simulink model "dynamic_model"  (R2018b)
(part 9 of 13)

t6273 = t692+t693+t702+t738+t1614+t1631+t1648+t1649+t2344+t2421+t2698+t2707+t2717+t2719+t3044+t3253+t3338+t3357+t3581+t3643+t3655+t4114+t4115;
t6274 = (t5413+t4146.*(t1861-t3221)).*(t2694-t2701+t3036-t3043).*(t1513+t1879+t2598+t2820+t2834+t3117+t3118).*(-3.633675e-3);
t6275 = (t5413+t4146.*(t1861-t3221)).*(t2694-t2701+t3036-t3043).*(t1513+t1879+t2598+t2820+t2834+t3117+t3118).*3.633675e-3;
t6281 = -t27.*t2363.*(t3435-t3448+t4615+t4619+t3976.*(t1896-t3239).*5.7e-7+t3980.*(t1896-t3239).*4.0e-8);
t6282 = t27.*t2363.*(t3435-t3448+t4615+t4619+t3976.*(t1896-t3239).*5.7e-7+t3980.*(t1896-t3239).*4.0e-8);
t6291 = t3934.*t5855.*(t1513+t1879+t2598+t2820+t2834+t3117+t3118).*(-3.633675e-3);
t6293 = t3934.*t5855.*(t1513+t1879+t2598+t2820+t2834+t3117+t3118).*3.633675e-3;
t6313 = -t2998.*(t3435-t3448+t4615+t4619+t3976.*(t1896-t3239).*5.7e-7+t3980.*(t1896-t3239).*4.0e-8);
t6314 = t2998.*(t3435-t3448+t4615+t4619+t3976.*(t1896-t3239).*5.7e-7+t3980.*(t1896-t3239).*4.0e-8).*(-1.0./2.0);
t6316 = (t5480.*t5603)./2.0;
t6334 = -t3055.*(t3435-t3448+t4615+t4619+t3976.*(t1896-t3239).*5.7e-7+t3980.*(t1896-t3239).*4.0e-8);
t6336 = (t1477-t2502).*(t3435-t3448+t4615+t4619+t3976.*(t1896-t3239).*5.7e-7+t3980.*(t1896-t3239).*4.0e-8);
t6340 = t3055.*(t3435-t3448+t4615+t4619+t3976.*(t1896-t3239).*5.7e-7+t3980.*(t1896-t3239).*4.0e-8).*(-1.0./2.0);
t6350 = -t2297.*(t642+t643-t667+t674+t1587+t1606+t1608+t1609+t2295+t2671+t2683+t2684-t2695+t3279+t3297-t3303+t3597+t3603+t3609-t3614+t4053+t4054);
t6351 = -t2307.*(t642+t643-t667+t674+t1587+t1606+t1608+t1609+t2295+t2671+t2683+t2684-t2695+t3279+t3297-t3303+t3597+t3603+t3609-t3614+t4053+t4054);
t6352 = -t2338.*(t642+t643-t667+t674+t1587+t1606+t1608+t1609+t2295+t2671+t2683+t2684-t2695+t3279+t3297-t3303+t3597+t3603+t3609-t3614+t4053+t4054);
t6353 = t2338.*(t642+t643-t667+t674+t1587+t1606+t1608+t1609+t2295+t2671+t2683+t2684-t2695+t3279+t3297-t3303+t3597+t3603+t3609-t3614+t4053+t4054);
t6354 = (t5466.*t5645)./2.0;
t6376 = -t3396.*(t4617+t4635-t12.*t2363.*t3047.*1.02e-6-t17.*t2363.*t3047.*9.0e-8+t12.*t3980.*(t1896-t3239).*1.02e-6+t17.*t3980.*(t1896-t3239).*9.0e-8);
t6379 = t3396.*(t4617+t4635-t12.*t2363.*t3047.*1.02e-6-t17.*t2363.*t3047.*9.0e-8+t12.*t3980.*(t1896-t3239).*1.02e-6+t17.*t3980.*(t1896-t3239).*9.0e-8);
t6382 = t2363.*(t684+t685-t710+t724+t1686-t1690+t1700+t1701+t2371+t2698+t2707-t2716+t2719+t3329-t3337-t3351-t3641+t3643+t3655-t3659+t4114+t4115).*(-7.26735e-3);
t6383 = t2388.*(t684+t685-t710+t724+t1686-t1690+t1700+t1701+t2371+t2698+t2707-t2716+t2719+t3329-t3337-t3351-t3641+t3643+t3655-t3659+t4114+t4115).*(-7.26735e-3);
t6386 = t2419.*(t684+t685-t710+t724+t1686-t1690+t1700+t1701+t2371+t2698+t2707-t2716+t2719+t3329-t3337-t3351-t3641+t3643+t3655-t3659+t4114+t4115).*(-7.26735e-3);
t6389 = t4002+t4243+t4332+t4408+t4466+t4647;
t6390 = t4797+t4805+t4815+t4825;
t6402 = t27.*(t1896-t3239).*(t3435-t3448+t4615+t4619+t3976.*(t1896-t3239).*5.7e-7+t3980.*(t1896-t3239).*4.0e-8);
t6403 = -t27.*t3547.*(t3435-t3448+t4615+t4619+t3976.*(t1896-t3239).*5.7e-7+t3980.*(t1896-t3239).*4.0e-8);
t6405 = t27.*t3547.*(t3435-t3448+t4615+t4619+t3976.*(t1896-t3239).*5.7e-7+t3980.*(t1896-t3239).*4.0e-8);
t6407 = t3910.*t5904.*(t1488+t1874+t2519+t2740+t2747+t3096+t3097).*(-1.0./2.0);
t6408 = (t3910.*t5904.*(t1488+t1874+t2519+t2740+t2747+t3096+t3097))./2.0;
t6416 = -t27.*t2363.*(t4795+t4801+t4808+t3976.*(t2694-t2701+t3036-t3043).*5.7e-7);
t6417 = t27.*t2363.*(t4795+t4801+t4808+t3976.*(t2694-t2701+t3036-t3043).*5.7e-7);
t6422 = -t2998.*(t4795+t4801+t4808+t3976.*(t2694-t2701+t3036-t3043).*5.7e-7);
t6423 = t2998.*(t4795+t4801+t4808+t3976.*(t2694-t2701+t3036-t3043).*5.7e-7).*(-1.0./2.0);
t6424 = (t2998.*(t4795+t4801+t4808+t3976.*(t2694-t2701+t3036-t3043).*5.7e-7))./2.0;
t6426 = -t3055.*(t4795+t4801+t4808+t3976.*(t2694-t2701+t3036-t3043).*5.7e-7);
t6428 = (t1477-t2502).*(t4795+t4801+t4808+t3976.*(t2694-t2701+t3036-t3043).*5.7e-7);
t6431 = t3055.*(t4795+t4801+t4808+t3976.*(t2694-t2701+t3036-t3043).*5.7e-7).*(-1.0./2.0);
t6432 = (t3055.*(t4795+t4801+t4808+t3976.*(t2694-t2701+t3036-t3043).*5.7e-7))./2.0;
t6441 = t4577.*t6101;
t6462 = t3395.*t6388;
t6471 = -t4019.*(t3435-t3448+t4615+t4619+t3976.*(t1896-t3239).*5.7e-7+t3980.*(t1896-t3239).*4.0e-8);
t6473 = (t3242-t3554).*(t3435-t3448+t4615+t4619+t3976.*(t1896-t3239).*5.7e-7+t3980.*(t1896-t3239).*4.0e-8);
t6474 = -t4026.*(t3435-t3448+t4615+t4619+t3976.*(t1896-t3239).*5.7e-7+t3980.*(t1896-t3239).*4.0e-8);
t6477 = -t4031.*(t3435-t3448+t4615+t4619+t3976.*(t1896-t3239).*5.7e-7+t3980.*(t1896-t3239).*4.0e-8);
t6485 = t27.*(t1896-t3239).*(t4795+t4801+t4808+t3976.*(t2694-t2701+t3036-t3043).*5.7e-7);
t6486 = -t27.*t3547.*(t4795+t4801+t4808+t3976.*(t2694-t2701+t3036-t3043).*5.7e-7);
t6488 = t27.*t3547.*(t4795+t4801+t4808+t3976.*(t2694-t2701+t3036-t3043).*5.7e-7);
t6512 = (t5645.*t5782)./2.0;
t6513 = (t5646.*t5782)./2.0;
t6530 = -t4019.*(t4795+t4801+t4808+t3976.*(t2694-t2701+t3036-t3043).*5.7e-7);
t6531 = (t3242-t3554).*(t4795+t4801+t4808+t3976.*(t2694-t2701+t3036-t3043).*5.7e-7);
t6533 = -t4026.*(t4795+t4801+t4808+t3976.*(t2694-t2701+t3036-t3043).*5.7e-7);
t6537 = -t4031.*(t4795+t4801+t4808+t3976.*(t2694-t2701+t3036-t3043).*5.7e-7);
t6538 = t4026.*(t4795+t4801+t4808+t3976.*(t2694-t2701+t3036-t3043).*5.7e-7);
t6549 = t3049+t3263+t3273+t4010+t4014+t4426+t4431+t4440+t4447;
t6559 = -t4573.*(t4617+t4635-t12.*t2363.*t3047.*1.02e-6-t17.*t2363.*t3047.*9.0e-8+t12.*t3980.*(t1896-t3239).*1.02e-6+t17.*t3980.*(t1896-t3239).*9.0e-8);
t6562 = (t3563-t4051).*(t4617+t4635-t12.*t2363.*t3047.*1.02e-6-t17.*t2363.*t3047.*9.0e-8+t12.*t3980.*(t1896-t3239).*1.02e-6+t17.*t3980.*(t1896-t3239).*9.0e-8);
t6569 = (t5480.*t5901)./2.0;
t6570 = (t5483.*t5901)./2.0;
t6572 = t5902.*(t410-t5466).*(-1.0./2.0);
t6591 = -t4874.*(t3435-t3448+t4615+t4619+t3976.*(t1896-t3239).*5.7e-7+t3980.*(t1896-t3239).*4.0e-8);
t6592 = -t4880.*(t3435-t3448+t4615+t4619+t3976.*(t1896-t3239).*5.7e-7+t3980.*(t1896-t3239).*4.0e-8);
t6596 = t4577.*t6388;
t6607 = t6606./2.0;
t6615 = t3181+t3198+t4793+t4800+t5066+t5071;
t6624 = -t3055.*(t4876+t4905+t4906+t3055.*(t1456-t2355).*1.02e-6+t3047.*(t1477-t2502).*1.02e-6+t3976.*(t3242-t3554).*1.02e-6);
t6625 = t3055.*(t4876+t4905+t4906+t3055.*(t1456-t2355).*1.02e-6+t3047.*(t1477-t2502).*1.02e-6+t3976.*(t3242-t3554).*1.02e-6).*(-1.0./2.0);
et163 = -t2137+t2777+t2778+t2779-t2787+t4050-t4246+t4248+t21.*(t1959-t3313+t38.*t1022.*(t855-t878).*2.196325630278387e-1).*6.1855407534e-5;
et164 = t27.*(t1959-t3313+t38.*t1022.*(t855-t878).*2.196325630278387e-1).*1.35652563578e-4;
t6653 = t5480.*(et163+et164).*(-1.0./2.0);
et165 = -t2137+t2777+t2778+t2779-t2787+t4050-t4246+t4248+t21.*(t1959-t3313+t38.*t1022.*(t855-t878).*2.196325630278387e-1).*6.1855407534e-5;
et166 = t27.*(t1959-t3313+t38.*t1022.*(t855-t878).*2.196325630278387e-1).*1.35652563578e-4;
t6654 = (t5480.*(et165+et166))./2.0;
et167 = -t2137+t2777+t2778+t2779-t2787+t4050-t4246+t4248+t21.*(t1959-t3313+t38.*t1022.*(t855-t878).*2.196325630278387e-1).*6.1855407534e-5;
et168 = t27.*(t1959-t3313+t38.*t1022.*(t855-t878).*2.196325630278387e-1).*1.35652563578e-4;
t6655 = t5483.*(et167+et168).*(-1.0./2.0);
et169 = -t2137+t2777+t2778+t2779-t2787+t4050-t4246+t4248+t21.*(t1959-t3313+t38.*t1022.*(t855-t878).*2.196325630278387e-1).*6.1855407534e-5;
et170 = t27.*(t1959-t3313+t38.*t1022.*(t855-t878).*2.196325630278387e-1).*1.35652563578e-4;
t6656 = (t5483.*(et169+et170))./2.0;
t6658 = t6048.*(t410-t5466).*(-1.0./2.0);
t6659 = -t4874.*(t4795+t4801+t4808+t3976.*(t2694-t2701+t3036-t3043).*5.7e-7);
t6660 = -t4880.*(t4795+t4801+t4808+t3976.*(t2694-t2701+t3036-t3043).*5.7e-7);
t6672 = (t5603.*t6011)./2.0;
t6673 = (t5645.*t6002)./2.0;
t6678 = (t5646.*t6002)./2.0;
et171 = t707+t708-t721-t722-t749+t762+t768-t777-t792-t793-t801-t802-t808+t813-t819+t821-t1629+t1637-t1640-t1641-t1659-t1661+t1666+t1667+t1683+t1692+t1705-t1712+t1758+t1759+t1775+t1776+t1973+t1993+t1994+t2023+t2053+t2060-t2089-t2090+t2098+t2099-t8.*t9.*t15.*t50.*t189.*3.670836568391568e-22;
et172 = t10.*t13.*t14.*t50.*t189.*(-3.279367663374749e-19)-t8.*t9.*t11.*t15.*t50.*t189.*7.075931802640439e-19;
et173 = t8.*t11.*t14.*t15.*t50.*t189.*(-1.190170786299927e-18)-t9.*t11.*t13.*t15.*t50.*t189.*1.190170786299927e-18;
et174 = t13.*t14.*t15.*t16.*t50.*t189.*(-3.226512155691387e-19);
t6687 = t5645.*(et171+et172+et173+et174).*(-1.0./2.0);
et175 = t707+t708-t721-t722-t749+t762+t768-t777-t792-t793-t801-t802-t808+t813-t819+t821-t1629+t1637-t1640-t1641-t1659-t1661+t1666+t1667+t1683+t1692+t1705-t1712+t1758+t1759+t1775+t1776+t1973+t1993+t1994+t2023+t2053+t2060-t2089-t2090+t2098+t2099-t8.*t9.*t15.*t50.*t189.*3.670836568391568e-22;
et176 = t10.*t13.*t14.*t50.*t189.*(-3.279367663374749e-19)-t8.*t9.*t11.*t15.*t50.*t189.*7.075931802640439e-19;
et177 = t8.*t11.*t14.*t15.*t50.*t189.*(-1.190170786299927e-18)-t9.*t11.*t13.*t15.*t50.*t189.*1.190170786299927e-18;
et178 = t13.*t14.*t15.*t16.*t50.*t189.*(-3.226512155691387e-19);
t6688 = (t5645.*(et175+et176+et177+et178))./2.0;
t6715 = -t6713;
t6747 = (t3242-t3554).*(t4876+t4905+t4906+t3055.*(t1456-t2355).*1.02e-6+t3047.*(t1477-t2502).*1.02e-6+t3976.*(t3242-t3554).*1.02e-6);
t6748 = -t4026.*(t4876+t4905+t4906+t3055.*(t1456-t2355).*1.02e-6+t3047.*(t1477-t2502).*1.02e-6+t3976.*(t3242-t3554).*1.02e-6);
t6750 = t4026.*(t4876+t4905+t4906+t3055.*(t1456-t2355).*1.02e-6+t3047.*(t1477-t2502).*1.02e-6+t3976.*(t3242-t3554).*1.02e-6);
t6804 = t3055.*t6726;
t6809 = t5226+t5227+t5229+t5230;
t6859 = (t5466.*t6255)./2.0;
et179 = t1288+t1289+t1302+t1303-t1319-t1320+t1336-t1348+t1350+t1351-t1360+t1369-t1378+t1396-t1425+t1435-t2174+t2183-t2187+t2193-t2194-t2195+t2199-t2203-t2215+t2219-t2222-t2223+t2239+t2240-t2256-t2257+t2555+t2556+t2572+t2583-t2605-t2606+t2612+t2613-t2618-t2619+t2651+t2652;
et180 = t18.*t19.*t20.*t50.*t202.*(-3.566935413776081e-21);
et181 = t24.*t25.*t26.*t50.*t202.*(-3.992732227073824e-24);
et182 = t18.*t19.*t26.*t27.*t50.*t202.*(-3.509445006623964e-21);
et183 = t21.*t24.*t25.*t26.*t50.*t202.*(-7.696420262413979e-21);
t6868 = t5480.*(et179+et180+et181+et182+et183).*(-1.0./2.0);
t6881 = -t21.*t2363.*(-t4494-t4495+t4799+t4823+t3976.*(t2694-t2701+t3036-t3043).*4.0e-8+t3980.*(t2694-t2701+t3036-t3043).*2.4e-7);
t6882 = t21.*t2363.*(-t4494-t4495+t4799+t4823+t3976.*(t2694-t2701+t3036-t3043).*4.0e-8+t3980.*(t2694-t2701+t3036-t3043).*2.4e-7).*(-1.0./2.0);
t6883 = (t21.*t2363.*(-t4494-t4495+t4799+t4823+t3976.*(t2694-t2701+t3036-t3043).*4.0e-8+t3980.*(t2694-t2701+t3036-t3043).*2.4e-7))./2.0;
t6896 = -t3003.*(-t4494-t4495+t4799+t4823+t3976.*(t2694-t2701+t3036-t3043).*4.0e-8+t3980.*(t2694-t2701+t3036-t3043).*2.4e-7);
t6897 = t3003.*(-t4494-t4495+t4799+t4823+t3976.*(t2694-t2701+t3036-t3043).*4.0e-8+t3980.*(t2694-t2701+t3036-t3043).*2.4e-7).*(-1.0./2.0);
t6898 = (t3003.*(-t4494-t4495+t4799+t4823+t3976.*(t2694-t2701+t3036-t3043).*4.0e-8+t3980.*(t2694-t2701+t3036-t3043).*2.4e-7))./2.0;
t6901 = -t3055.*(-t4494-t4495+t4799+t4823+t3976.*(t2694-t2701+t3036-t3043).*4.0e-8+t3980.*(t2694-t2701+t3036-t3043).*2.4e-7);
t6902 = (t1477-t2502).*(-t4494-t4495+t4799+t4823+t3976.*(t2694-t2701+t3036-t3043).*4.0e-8+t3980.*(t2694-t2701+t3036-t3043).*2.4e-7);
t6905 = -t6726.*(t3242-t3554);
t6906 = t4026.*t6726;
t6913 = t4355+t4362+t4929+t4930+t5029+t5030;
t6914 = t5100+t5736+t5749;
t6916 = t3909+t4319+t5019+t5020+t5054+t5055;
t6921 = t21.*(t1896-t3239).*(-t4494-t4495+t4799+t4823+t3976.*(t2694-t2701+t3036-t3043).*4.0e-8+t3980.*(t2694-t2701+t3036-t3043).*2.4e-7);
t6922 = -t21.*t3547.*(-t4494-t4495+t4799+t4823+t3976.*(t2694-t2701+t3036-t3043).*4.0e-8+t3980.*(t2694-t2701+t3036-t3043).*2.4e-7);
t6943 = t3134+t3161+t3162+t3389+t4279+t4283+t4293+t4294+t4299+t4300+t4562+t4568;
t6978 = -t4019.*(-t4494-t4495+t4799+t4823+t3976.*(t2694-t2701+t3036-t3043).*4.0e-8+t3980.*(t2694-t2701+t3036-t3043).*2.4e-7);
t6979 = (t3242-t3554).*(-t4494-t4495+t4799+t4823+t3976.*(t2694-t2701+t3036-t3043).*4.0e-8+t3980.*(t2694-t2701+t3036-t3043).*2.4e-7);
t6980 = -t4026.*(-t4494-t4495+t4799+t4823+t3976.*(t2694-t2701+t3036-t3043).*4.0e-8+t3980.*(t2694-t2701+t3036-t3043).*2.4e-7);
t6984 = -t4031.*(-t4494-t4495+t4799+t4823+t3976.*(t2694-t2701+t3036-t3043).*4.0e-8+t3980.*(t2694-t2701+t3036-t3043).*2.4e-7);
t7002 = t5285+t5293+t5329+t5334;
t7010 = t4018.*(t4814.*(t1861-t3221)+t2297.*(t642+t643-t667+t674+t1587+t1606+t1608+t1609+t2295+t2671+t2683+t2684-t2695+t3279+t3297-t3303+t3597+t3603+t3609-t3614+t4053+t4054)).*(t2694-t2701+t3036-t3043).*3.633675e-3;
t7016 = t3910.*t6652.*(t1488+t1874+t2519+t2740+t2747+t3096+t3097).*(-1.0./2.0);
t7017 = (t3910.*t6652.*(t1488+t1874+t2519+t2740+t2747+t3096+t3097))./2.0;
t7018 = t4187.*(t4814.*(t1861-t3221)+t2297.*(t642+t643-t667+t674+t1587+t1606+t1608+t1609+t2295+t2671+t2683+t2684-t2695+t3279+t3297-t3303+t3597+t3603+t3609-t3614+t4053+t4054)).*(t2694-t2701+t3036-t3043).*3.633675e-3;
t7055 = t7054.*(-1.0./2.0);
t7056 = t7054./2.0;
t7059 = (t3975.*(t4853.*(t1896-t3239).*7.26735e-3+t2363.*(t684+t685-t710+t724+t1686-t1690+t1700+t1701+t2371+t2698+t2707-t2716+t2719+t3329-t3337-t3351-t3641+t3643+t3655-t3659+t4114+t4115).*7.26735e-3).*(t2674-t2676+t3022-t3027))./2.0;
t7080 = (t4146.*(t4853.*(t1896-t3239).*7.26735e-3+t2363.*(t684+t685-t710+t724+t1686-t1690+t1700+t1701+t2371+t2698+t2707-t2716+t2719+t3329-t3337-t3351-t3641+t3643+t3655-t3659+t4114+t4115).*7.26735e-3).*(t2674-t2676+t3022-t3027))./2.0;
t7082 = t5264+t5806+t5822;
t7092 = t3159+t3172+t3449+t3453+t4297+t4304+t4306+t4311+t4579+t4600+t4625+t4629;
t7100 = -t4872.*(-t4494-t4495+t4799+t4823+t3976.*(t2694-t2701+t3036-t3043).*4.0e-8+t3980.*(t2694-t2701+t3036-t3043).*2.4e-7);
et184 = t4165+t27.*(t1959-t3313+t38.*t1022.*(t855-t878).*2.196325630278387e-1);
et185 = -t4494-t4495+t4799+t4823+t3976.*(t2694-t2701+t3036-t3043).*4.0e-8+t3980.*(t2694-t2701+t3036-t3043).*2.4e-7;
t7101 = et184.*et185;
t7155 = t3577+t3578+t5315+t5316+t5323+t5324;
et186 = t3582.*1.33637554986e-4+t3716-t3717+t27.*(t1896-t3239).*4.36041e-5;
et187 = t27.*t28.*(t1896-t3239).*7.26350557185e-5;
t7159 = ((et186+et187).*(t4814.*(t1861-t3221)+t2297.*(t642+t643-t667+t674+t1587+t1606+t1608+t1609+t2295+t2671+t2683+t2684-t2695+t3279+t3297-t3303+t3597+t3603+t3609-t3614+t4053+t4054)))./2.0;
et188 = t4814.*(t1861-t3221)+t2297.*(t642+t643-t667+t674+t1587+t1606+t1608+t1609+t2295+t2671+t2683+t2684-t2695+t3279+t3297-t3303+t3597+t3603+t3609-t3614+t4053+t4054);
et189 = (t3359-t3670+t22.*(t3242-t3554).*1.33637554986e-4+t28.*(t3242-t3554).*7.26350557185e-5)./2.0;
t7162 = et188.*et189;
t7165 = t7083.*(-t1901+t3122+t3277).*(-1.0./2.0);
t7166 = t50.*t202.*t7151.*6.935255936130809e-19;
et190 = t4853.*(t1896-t3239).*7.26735e-3+t2363.*(t684+t685-t710+t724+t1686-t1690+t1700+t1701+t2371+t2698+t2707-t2716+t2719+t3329-t3337-t3351-t3641+t3643+t3655-t3659+t4114+t4115).*7.26735e-3;
et191 = (t3524.*1.838876e-2-t3591+t3592+t16.*(t1861-t3221).*(3.0./5.0e+2)+t16.*t17.*(t1861-t3221).*9.99471e-3)./2.0;
t7170 = et190.*et191;
t7178 = t5313.*(t4853.*(t1896-t3239).*7.26735e-3+t2363.*(t684+t685-t710+t724+t1686-t1690+t1700+t1701+t2371+t2698+t2707-t2716+t2719+t3329-t3337-t3351-t3641+t3643+t3655-t3659+t4114+t4115).*7.26735e-3).*(-1.0./2.0);
et192 = (t4814.*(t1861-t3221)+t2297.*(t642+t643-t667+t674+t1587+t1606+t1608+t1609+t2295+t2671+t2683+t2684-t2695+t3279+t3297-t3303+t3597+t3603+t3609-t3614+t4053+t4054)).*(t3566.*1.33637554986e-4+t4157-t4158+t28.*(t1896-t3239).*7.26350557185e-5);
et193 = 1.0./2.0;
t7197 = et192.*et193;
t7201 = t2363.*t7173.*7.26735e-3;
et194 = t4853.*(t1896-t3239).*7.26735e-3+t2363.*(t684+t685-t710+t724+t1686-t1690+t1700+t1701+t2371+t2698+t2707-t2716+t2719+t3329-t3337-t3351-t3641+t3643+t3655-t3659+t4114+t4115).*7.26735e-3;
et195 = (-t4045+t4049+t12.*(t1861-t3221).*1.838876e-2+t17.*(t1861-t3221).*9.99471e-3)./2.0;
t7204 = et194.*et195;
t7256 = ((t4673+t2363.*(t3566.*1.838876e-2+t4109-t4110+t28.*(t1896-t3239).*9.99471e-3).*7.26735e-3).*(t4814.*(t1861-t3221)+t2297.*(t642+t643-t667+t674+t1587+t1606+t1608+t1609+t2295+t2671+t2683+t2684-t2695+t3279+t3297-t3303+t3597+t3603+t3609-t3614+t4053+t4054)))./2.0;
tau_c = ft_13({dq1,dq2,dq3,dq4,dq5,dq6,t10,t1005,t1022,t1089,t11,t1104,t1105,t1108,t1115,t1121,t1158,t1159,t1196,t12,t1205,t1210,t1212,t1217,t1218,t123,t1237,t1238,t1288,t1289,t13,t1302,t1303,t1319,t1320,t1336,t1348,t1350,t1351,t1360,t1369,t1378,t1396,t14,t140,t1425,t1435,t1456,t1477,t1488,t15,t1513,t1539,t1554,t1577,t1578,t1586,t1587,t16,t1600,t1604,t1605,t1606,t1607,t1608,t1609,t1615,t1616,t1628,t1629,t1637,t1640,t1641,t1659,t1660,t1661,t1666,t1667,t1683,t1686,t1690,t1692,t17,t1700,t1701,t1705,t1712,t1717,t1741,t1742,t1750,t1754,t1758,t1759,t1775,t1776,t18,t1861,t1874,t1879,t188,t1881,t189,t1896,t19,t1901,t1941,t1959,t1973,t1993,t1994,t20,t201,t202,t2023,t2053,t2060,t2089,t2090,t2098,t2099,t21,t2117,t2120,t2122,t2123,t2139,t2140,t2147,t2152,t2154,t2155,t2159,t2165,t2174,t2183,t2187,t2193,t2194,t2195,t2199,t22,t2203,t2215,t2219,t2222,t2223,t2239,t2240,t2256,t2257,t2292,t2295,t2297,t2302,t2303,t2306,t2307,t2308,t2317,t2337,t2338,t2339,t2355,t236,t2361,t2362,t2363,t2367,t2368,t237,t2371,t2378,t238,t2388,t2399,t24,t2401,t2403,t241,t2414,t2419,t2493,t25,t2502,t2510,t2519,t2527,t2530,t2555,t2556,t2572,t2583,t2598,t26,t2605,t2606,t2612,t2613,t2618,t2619,t262,t264,t2651,t2652,t2670,t2671,t2673,t2674,t2676,t2680,t2683,t2684,t2685,t2686,t2687,t2689,t2692,t2693,t2694,t2695,t2697,t2698,t27,t2700,t2701,t2704,t2707,t2708,t2709,t2712,t2715,t2716,t2719,t2720,t2721,t2740,t2747,t2748,t2749,t2754,t2773,t2781,t2788,t28,t2801,t2804,t2813,t2814,t2820,t2831,t2834,t2835,t2838,t2850,t2851,t29,t2945,t2950,t2953,t2955,t2957,t2965,t2966,t2975,t2979,t2990,t2991,t2993,t2994,t2998,t30,t3003,t3009,t3015,t3017,t3022,t3027,t3030,t3036,t3043,t3045,t3047,t3054,t3055,t3057,t3058,t3063,t3064,t3068,t3072,t3079,t3080,t3096,t3097,t31,t3109,t3117,t3118,t3121,t3122,t3126,t3129,t313,t3130,t3131,t3132,t3133,t3135,t3136,t314,t3140,t3141,t3142,t3143,t3145,t3148,t3156,t3157,t3158,t3165,t3167,t3171,t3173,t3185,t3187,t3188,t3189,t3190,t3192,t3193,t3194,t3195,t3196,t3199,t32,t3200,t3201,t3202,t3203,t3205,t3206,t3208,t3209,t321,t3211,t3213,t3216,t3217,t3221,t3232,t3235,t3236,t3237,t3238,t3239,t3242,t3252,t3257,t3261,t3267,t3268,t3270,t3276,t3277,t3279,t3283,t329,t3290,t3297,t3298,t3299,t33,t3303,t3312,t3313,t3314,t3315,t3318,t332,t3322,t3324,t3326,t3328,t3329,t3334,t3336,t3337,t3340,t3344,t3345,t3346,t3347,t335,t3351,t3354,t3359,t3363,t3364,t3367,t3369,t3370,t3386,t3395,t3396,t34,t3405,t3409,t3415,t3416,t3420,t3421,t3423,t3426,t3428,t3430,t3431,t3432,t3434,t3435,t3439,t3443,t3444,t3446,t3448,t3451,t3455,t346,t3460,t3461,t3462,t3463,t3465,t3468,t3469,t3471,t3474,t3480,t3482,t3483,t3488,t3489,t3490,t3492,t3495,t3496,t3498,t3499,t35,t350,t3500,t3502,t3503,t3512,t3517,t3524,t3537,t354,t3541,t3543,t3545,t3546,t3547,t3549,t3550,t3551,t3552,t3554,t3558,t3561,t3563,t3566,t358,t3582,t3588,t3589,t359,t3590,t3591,t3592,t3597,t36,t3603,t3606,t3607,t3608,t3609,t3610,t3611,t3614,t3617,t3621,t3624,t3637,t3638,t3639,t3640,t3641,t3642,t3643,t3649,t3652,t3653,t3654,t3655,t3656,t3658,t3659,t366,t3660,t3662,t3664,t3670,t3678,t3684,t3688,t3689,t3690,t3692,t3693,t3695,t3696,t3697,t3699,t3701,t3702,t3703,t3704,t3705,t3706,t3707,t3708,t3709,t3710,t3712,t3713,t3716,t3717,t3728,t3729,t3731,t3732,t3735,t3736,t3737,t3738,t3739,t3741,t3746,t3747,t3752,t3755,t3759,t3765,t3766,t3770,t3771,t3772,t3774,t3775,t3777,t3779,t378,t3781,t3782,t3783,t3784,t3785,t3786,t3788,t3789,t3790,t3791,t3792,t3793,t3794,t3795,t3796,t3797,t3798,t38,t3800,t3801,t3802,t3804,t3805,t3808,t3809,t3810,t3817,t3818,t382,t3820,t3821,t3823,t3824,t3826,t3827,t3828,t3830,t3832,t3833,t3835,t3840,t3843,t3844,t3845,t3846,t3848,t3850,t3851,t3855,t3856,t3857,t3862,t3863,t387,t3873,t3876,t3877,t3878,t3879,t3880,t3889,t3890,t3891,t3893,t3895,t3896,t3897,t3898,t39,t3901,t3902,t3903,t3906,t3908,t3910,t3913,t3915,t3924,t3925,t3926,t3931,t3934,t3937,t3943,t3951,t3961,t3967,t3968,t3974,t3975,t3976,t3977,t3980,t3985,t3991,t3993,t4001,t4006,t4008,t4018,t4019,t4026,t4030,t4031,t4032,t4035,t4039,t4041,t4045,t4047,t4049,t4051,t4053,t4054,t4065,t4072,t4073,t4074,t4075,t410,t4100,t4109,t4110,t4114,t4115,t4118,t4124,t4127,t4128,t4129,t4144,t4146,t4147,t4151,t4153,t4154,t4157,t4158,t4160,t4163,t4165,t4171,t4172,t4183,t4184,t4185,t4186,t4187,t4190,t4193,t4198,t42,t4201,t4205,t4207,t4208,t4213,t4215,t4236,t4240,t4244,t4260,t4261,t4263,t4270,t4272,t4273,t4274,t4275,t4276,t4277,t4278,t4280,t4281,t4282,t4286,t4287,t4288,t4289,t4290,t4291,t4292,t4299,t43,t4300,t4301,t4303,t4307,t4308,t4310,t4312,t4313,t4314,t4318,t4321,t4324,t4325,t4326,t4330,t4332,t4334,t4337,t4339,t4341,t4342,t4343,t4344,t4345,t4346,t4352,t4356,t4358,t4359,t4361,t4364,t4368,t4371,t4372,t4373,t4375,t4406,t4413,t4415,t4416,t4417,t4427,t4429,t4430,t4432,t4435,t4441,t4450,t4451,t4458,t4459,t4461,t4464,t4465,t4467,t4468,t4470,t4476,t4479,t4482,t4486,t4488,t4489,t4493,t4494,t4495,t4496,t4497,t4501,t4502,t4504,t4515,t4518,t4520,t4522,t4532,t4534,t4537,t4545,t4553,t4556,t4559,t4562,t4563,t4567,t4570,t4571,t4573,t4574,t4576,t4577,t4578,t4580,t4582,t4583,t4586,t4588,t4592,t4594,t4597,t4598,t4599,t46,t4603,t4604,t4606,t4615,t4617,t4618,t4619,t4622,t4623,t4624,t4628,t4631,t4634,t4635,t4638,t4639,t4642,t4643,t4644,t4645,t4651,t4652,t4654,t4656,t4657,t4658,t4660,t4662,t4663,t4665,t4673,t4675,t4676,t4677,t4678,t4680,t4683,t4686,t4688,t4690,t4691,t4692,t4694,t4696,t4697,t4698,t4699,t47,t4701,t4703,t4704,t4705,t4708,t4709,t4712,t4713,t4716,t4719,t4720,t4722,t4724,t4725,t4727,t4728,t4730,t4737,t4738,t4739,t4741,t4743,t4744,t4746,t4751,t4757,t4760,t4761,t4762,t4763,t4764,t4767,t4771,t4773,t4776,t4777,t4778,t4779,t4783,t4785,t4786,t4787,t4790,t4791,t4795,t4796,t4799,t4801,t4808,t4809,t4810,t4811,t4813,t4814,t4816,t4817,t4818,t4819,t4822,t4823,t4826,t4827,t4828,t4829,t4832,t4833,t4835,t4838,t4843,t4844,t4845,t4846,t4847,t4848,t4849,t4850,t4851,t4852,t4853,t4854,t4856,t4857,t4858,t4859,t4863,t4865,t4866,t4867,t4870,t4872,t4874,t4875,t4876,t4879,t4880,t4881,t4886,t4887,t4888,t4889,t4892,t4893,t4895,t4896,t4898,t4901,t4902,t4903,t4904,t4905,t4906,t4907,t4908,t4909,t4910,t4911,t4912,t4913,t4914,t4915,t4920,t4923,t4924,t4925,t4926,t4927,t4928,t4933,t4935,t4936,t4937,t4938,t4940,t4943,t4946,t4948,t4949,t4950,t4952,t4953,t4955,t4957,t4958,t4959,t4960,t4962,t4965,t4967,t4969,t4970,t4971,t4972,t4973,t4974,t4976,t4977,t4978,t4979,t4981,t4982,t4983,t4989,t4992,t4993,t4994,t4997,t4998,t50,t5001,t5003,t5004,t5005,t5007,t5009,t5010,t5011,t5012,t5013,t5014,t5016,t5021,t5023,t5025,t5026,t5027,t5028,t5032,t5033,t5034,t5035,t5036,t5037,t5038,t5041,t5042,t5043,t5045,t5046,t5047,t5049,t5051,t5052,t5053,t5057,t5059,t5061,t5062,t5063,t5064,t5070,t5072,t5074,t5075,t5076,t5077,t5079,t5080,t5081,t5082,t5083,t5084,t5085,t5086,t5087,t5088,t5089,t5090,t5091,t5093,t5096,t5097,t5098,t5101,t5103,t5105,t5106,t5108,t5109,t5111,t5112,t5113,t5114,t5116,t5117,t5118,t5119,t5120,t5121,t5123,t5124,t5125,t5126,t5127,t5133,t5135,t5136,t5137,t5138,t5139,t5141,t5142,t5147,t5148,t5149,t5150,t5152,t5153,t5154,t5155,t5156,t5158,t5159,t5161,t5162,t5163,t5164,t5165,t5166,t5167,t5169,t5171,t5173,t5176,t5177,t5178,t5180,t5181,t5185,t5187,t5188,t5189,t5191,t5192,t5193,t5194,t5195,t5196,t5197,t5198,t5199,t5200,t5201,t5202,t5203,t5205,t5206,t5207,t5208,t5211,t5212,t5213,t5214,t5215,t5216,t5219,t5222,t5223,t5234,t5235,t5236,t5237,t5240,t5241,t5243,t5244,t5245,t5246,t5247,t5248,t5249,t5251,t5254,t5255,t5256,t5257,t5258,t5259,t5261,t5262,t5263,t5264,t5265,t5267,t5269,t5270,t5271,t5272,t5275,t5276,t5277,t5278,t5279,t5280,t5281,t5283,t5284,t5286,t5287,t5289,t5290,t5291,t5292,t5294,t5295,t5296,t5297,t5298,t5300,t5301,t5302,t5303,t5304,t5305,t5306,t5308,t5309,t5310,t5312,t5313,t5317,t5326,t5327,t5328,t5331,t5332,t5333,t5335,t5336,t5337,t5338,t5339,t5340,t5341,t5342,t5343,t5344,t5345,t5346,t5348,t5350,t5352,t5353,t5356,t5357,t5358,t5359,t5361,t5362,t5363,t5364,t5366,t5369,t5370,t5372,t5373,t5374,t5376,t5379,t5381,t5382,t5383,t5384,t5385,t5386,t5387,t5389,t5390,t5391,t5392,t5393,t5395,t5399,t5400,t5401,t5402,t5403,t5404,t5405,t5406,t5410,t5411,t5412,t5413,t5415,t5416,t5419,t5421,t5422,t5425,t5426,t5433,t5434,t5436,t5437,t5438,t5439,t5440,t5441,t5442,t5443,t5444,t5445,t5446,t5448,t5449,t5451,t5452,t5453,t5456,t5457,t5458,t5459,t5460,t5461,t5462,t5464,t5465,t5466,t5467,t5470,t5472,t5473,t5474,t5477,t5478,t5480,t5481,t5483,t5484,t5486,t5487,t5488,t5489,t5491,t5493,t5494,t5495,t5497,t5499,t5500,t5501,t5502,t5503,t5504,t5505,t5506,t5507,t5508,t5509,t5510,t5511,t5512,t5513,t5514,t5516,t5517,t5519,t5520,t5521,t5522,t5523,t5524,t5528,t5529,t5531,t5532,t5534,t5535,t5536,t5537,t5538,t5539,t5540,t5542,t5543,t5544,t5545,t5548,t5549,t5550,t5553,t5554,t5555,t5556,t5557,t5558,t5560,t5563,t5564,t5565,t5567,t5568,t5569,t5570,t5572,t5573,t5574,t5575,t5576,t5577,t5578,t5579,t5581,t5583,t5585,t5586,t5587,t5588,t5589,t5590,t5591,t5592,t5593,t5594,t5596,t5597,t5598,t5599,t56,t5600,t5601,t5602,t5603,t5604,t5605,t5606,t5607,t5608,t5609,t5611,t5612,t5613,t5614,t5615,t5616,t5618,t5619,t5622,t5623,t5624,t5625,t5629,t5630,t5631,t5632,t5633,t5634,t5635,t5636,t5637,t5638,t5640,t5645,t5646,t5647,t5649,t5650,t5651,t5652,t5653,t5655,t5657,t5658,t5659,t5660,t5661,t5662,t5663,t5667,t5672,t5675,t5677,t5678,t5679,t5680,t5681,t5682,t5683,t5684,t5685,t5686,t5687,t5688,t5689,t5690,t5691,t5694,t5695,t5698,t5699,t5700,t5703,t5707,t5710,t5712,t5714,t5717,t5718,t5719,t5720,t5721,t5722,t5723,t5724,t5725,t5727,t5730,t5731,t5734,t5735,t5738,t5739,t5740,t5741,t5742,t5745,t5746,t5747,t5750,t5751,t5753,t5754,t5756,t5757,t5758,t5759,t5760,t5761,t5762,t5763,t5764,t5765,t5766,t5768,t5769,t5770,t5772,t5773,t5775,t5776,t5777,t5778,t5779,t5781,t5782,t5783,t5784,t5787,t5788,t5790,t5792,t5793,t5794,t5795,t5801,t5802,t5804,t5809,t5810,t5813,t5814,t5816,t5821,t5824,t5825,t5826,t5828,t5829,t5831,t5832,t5833,t5834,t5835,t5836,t5838,t5839,t5840,t5842,t5844,t5845,t5846,t5849,t5851,t5852,t5853,t5855,t5857,t5858,t5863,t5864,t5866,t5867,t5868,t5871,t5872,t5874,t5875,t5876,t5877,t5878,t5879,t5884,t5886,t5887,t5888,t5890,t5891,t5892,t5893,t5894,t5896,t5897,t5899,t5900,t5901,t5902,t5904,t5905,t5907,t5908,t5909,t5913,t5914,t5915,t5916,t5917,t5918,t5919,t5920,t5922,t5923,t5924,t5925,t5926,t5927,t5928,t5930,t5931,t5933,t5934,t5938,t5939,t5941,t5942,t5943,t5945,t5946,t5949,t5950,t5951,t5954,t5955,t5959,t5960,t5963,t5965,t5966,t5967,t5968,t5971,t5973,t5974,t5975,t5978,t5979,t5980,t5981,t5983,t5984,t5985,t5990,t5992,t5993,t5996,t5998,t60,t6001,t6004,t6005,t6006,t6008,t6011,t6013,t6014,t6015,t6017,t6018,t6019,t6020,t6021,t6022,t6023,t6024,t6026,t6031,t6034,t6035,t6036,t6037,t6042,t6044,t6047,t6048,t6050,t6052,t6053,t6054,t6057,t6058,t6059,t6062,t6065,t6066,t6067,t6069,t6071,t6072,t6074,t6076,t6079,t6080,t6081,t6091,t6093,t6094,t6095,t6096,t6098,t6101,t6102,t6105,t6106,t6109,t6110,t6113,t6114,t6115,t6119,t6123,t6125,t6127,t6129,t6131,t6133,t6134,t6143,t6144,t6158,t6159,t6162,t6164,t6166,t6168,t6171,t6172,t6174,t6183,t6190,t6211,t6213,t6217,t6219,t6221,t6227,t6231,t6232,t6233,t6234,t6236,t6239,t6240,t6241,t6245,t6247,t6255,t6256,t6257,t6260,t6270,t6271,t6272,t6273,t6275,t6281,t6282,t6291,t6293,t6307,t6313,t6314,t6316,t6324,t6334,t6336,t6350,t6351,t6353,t6354,t6366,t6375,t6376,t6377,t6379,t6382,t6383,t6386,t6388,t6390,t6394,t6396,t6398,t640,t6402,t6405,t6407,t6408,t6411,t6412,t6417,t642,t6422,t6423,t6425,t6426,t6428,t643,t6431,t6432,t6438,t6440,t6441,t6442,t6460,t6461,t6462,t6471,t6473,t6474,t6477,t6482,t6483,t6484,t6485,t6488,t649,t6491,t6508,t6512,t6513,t6515,t6517,t6523,t6524,t6525,t6526,t6527,t6528,t6530,t6531,t6537,t6538,t6549,t6559,t656,t6560,t6562,t6564,t6565,t6569,t6570,t6572,t6574,t6576,t6588,t6589,t659,t6591,t6592,t6594,t6595,t6596,t660,t6601,t6602,t6606,t6607,t6615,t6622,t6623,t6624,t6625,t6651,t6652,t6654,t6656,t6658,t6659,t6660,t6661,t667,t6671,t6672,t6673,t6678,t668,t6680,t6687,t6688,t669,t67,t670,t6714,t6715,t674,t6745,t6747,t6750,t6751,t677,t68,t6804,t6809,t681,t682,t684,t685,t6858,t6859,t686,t6868,t687,t6881,t6882,t6883,t6896,t6897,t6901,t6902,t6905,t6906,t6913,t6914,t6916,t6919,t6920,t6921,t6922,t694,t6965,t6966,t6974,t6976,t6978,t6979,t6980,t6984,t6987,t7003,t7005,t7007,t7010,t7014,t7016,t7018,t7020,t7021,t7035,t7054,t7055,t7059,t707,t708,t7080,t7083,t7086,t7088,t7092,t7094,t7095,t7097,t7098,t71,t710,t7100,t7101,t7120,t7123,t7134,t7136,t7137,t7138,t7148,t715,t7150,t7153,t7155,t7158,t7159,t716,t7160,t7162,t7164,t7166,t7169,t7170,t7197,t7199,t7201,t7204,t721,t722,t724,t725,t7256,t7283,t7292,t73,t7304,t7319,t7332,t7333,t736,t7385,t740,t7400,t7401,t7403,t741,t749,t762,t768,t777,t7784,t7790,t7827,t792,t793,t8,t801,t802,t808,t813,t819,t821,t850,t855,t874,t878,t89,t9,t92,t941,t948,t951,t97});
end
function tau_c = ft_13(ct)
dq1 = ct{1};
dq2 = ct{2};
dq3 = ct{3};
dq4 = ct{4};
dq5 = ct{5};
dq6 = ct{6};
t10 = ct{7};
t1005 = ct{8};
t1022 = ct{9};
t1089 = ct{10};
t11 = ct{11};
t1104 = ct{12};
t1105 = ct{13};
t1108 = ct{14};
t1115 = ct{15};
t1121 = ct{16};
t1158 = ct{17};
t1159 = ct{18};
t1196 = ct{19};
t12 = ct{20};
t1205 = ct{21};
t1210 = ct{22};
t1212 = ct{23};
t1217 = ct{24};
t1218 = ct{25};
t123 = ct{26};
t1237 = ct{27};
t1238 = ct{28};
t1288 = ct{29};
t1289 = ct{30};
t13 = ct{31};
t1302 = ct{32};
t1303 = ct{33};
t1319 = ct{34};
t1320 = ct{35};
t1336 = ct{36};
t1348 = ct{37};
t1350 = ct{38};
t1351 = ct{39};
t1360 = ct{40};
t1369 = ct{41};
t1378 = ct{42};
t1396 = ct{43};
t14 = ct{44};
t140 = ct{45};
t1425 = ct{46};
t1435 = ct{47};
t1456 = ct{48};
t1477 = ct{49};
t1488 = ct{50};
t15 = ct{51};
t1513 = ct{52};
t1539 = ct{53};
t1554 = ct{54};
t1577 = ct{55};
t1578 = ct{56};
t1586 = ct{57};
t1587 = ct{58};
t16 = ct{59};
t1600 = ct{60};
t1604 = ct{61};
t1605 = ct{62};
t1606 = ct{63};
t1607 = ct{64};
t1608 = ct{65};
t1609 = ct{66};
t1615 = ct{67};
t1616 = ct{68};
t1628 = ct{69};
t1629 = ct{70};
t1637 = ct{71};
t1640 = ct{72};
t1641 = ct{73};
t1659 = ct{74};
t1660 = ct{75};
t1661 = ct{76};
t1666 = ct{77};
t1667 = ct{78};
t1683 = ct{79};
t1686 = ct{80};
t1690 = ct{81};
t1692 = ct{82};
t17 = ct{83};
t1700 = ct{84};
t1701 = ct{85};
t1705 = ct{86};
t1712 = ct{87};
t1717 = ct{88};
t1741 = ct{89};
t1742 = ct{90};
t1750 = ct{91};
t1754 = ct{92};
t1758 = ct{93};
t1759 = ct{94};
t1775 = ct{95};
t1776 = ct{96};
t18 = ct{97};
t1861 = ct{98};
t1874 = ct{99};
t1879 = ct{100};
t188 = ct{101};
t1881 = ct{102};
t189 = ct{103};
t1896 = ct{104};
t19 = ct{105};
t1901 = ct{106};
t1941 = ct{107};
t1959 = ct{108};
t1973 = ct{109};
t1993 = ct{110};
t1994 = ct{111};
t20 = ct{112};
t201 = ct{113};
t202 = ct{114};
t2023 = ct{115};
t2053 = ct{116};
t2060 = ct{117};
t2089 = ct{118};
t2090 = ct{119};
t2098 = ct{120};
t2099 = ct{121};
t21 = ct{122};
t2117 = ct{123};
t2120 = ct{124};
t2122 = ct{125};
t2123 = ct{126};
t2139 = ct{127};
t2140 = ct{128};
t2147 = ct{129};
t2152 = ct{130};
t2154 = ct{131};
t2155 = ct{132};
t2159 = ct{133};
t2165 = ct{134};
t2174 = ct{135};
t2183 = ct{136};
t2187 = ct{137};
t2193 = ct{138};
t2194 = ct{139};
t2195 = ct{140};
t2199 = ct{141};
t22 = ct{142};
t2203 = ct{143};
t2215 = ct{144};
t2219 = ct{145};
t2222 = ct{146};
t2223 = ct{147};
t2239 = ct{148};
t2240 = ct{149};
t2256 = ct{150};
t2257 = ct{151};
t2292 = ct{152};
t2295 = ct{153};
t2297 = ct{154};
t2302 = ct{155};
t2303 = ct{156};
t2306 = ct{157};
t2307 = ct{158};
t2308 = ct{159};
t2317 = ct{160};
t2337 = ct{161};
t2338 = ct{162};
t2339 = ct{163};
t2355 = ct{164};
t236 = ct{165};
t2361 = ct{166};
t2362 = ct{167};
t2363 = ct{168};
t2367 = ct{169};
t2368 = ct{170};
t237 = ct{171};
t2371 = ct{172};
t2378 = ct{173};
t238 = ct{174};
t2388 = ct{175};
t2399 = ct{176};
t24 = ct{177};
t2401 = ct{178};
t2403 = ct{179};
t241 = ct{180};
t2414 = ct{181};
t2419 = ct{182};
t2493 = ct{183};
t25 = ct{184};
t2502 = ct{185};
t2510 = ct{186};
t2519 = ct{187};
t2527 = ct{188};
t2530 = ct{189};
t2555 = ct{190};
t2556 = ct{191};
t2572 = ct{192};
t2583 = ct{193};
t2598 = ct{194};
t26 = ct{195};
t2605 = ct{196};
t2606 = ct{197};
t2612 = ct{198};
t2613 = ct{199};
t2618 = ct{200};
t2619 = ct{201};
t262 = ct{202};
t264 = ct{203};
t2651 = ct{204};
t2652 = ct{205};
t2670 = ct{206};
t2671 = ct{207};
t2673 = ct{208};
t2674 = ct{209};
t2676 = ct{210};
t2680 = ct{211};
t2683 = ct{212};
t2684 = ct{213};
t2685 = ct{214};
t2686 = ct{215};
t2687 = ct{216};
t2689 = ct{217};
t2692 = ct{218};
t2693 = ct{219};
t2694 = ct{220};
t2695 = ct{221};
t2697 = ct{222};
t2698 = ct{223};
t27 = ct{224};
t2700 = ct{225};
t2701 = ct{226};
t2704 = ct{227};
t2707 = ct{228};
t2708 = ct{229};
t2709 = ct{230};
t2712 = ct{231};
t2715 = ct{232};
t2716 = ct{233};
t2719 = ct{234};
t2720 = ct{235};
t2721 = ct{236};
t2740 = ct{237};
t2747 = ct{238};
t2748 = ct{239};
t2749 = ct{240};
t2754 = ct{241};
t2773 = ct{242};
t2781 = ct{243};
t2788 = ct{244};
t28 = ct{245};
t2801 = ct{246};
t2804 = ct{247};
t2813 = ct{248};
t2814 = ct{249};
t2820 = ct{250};
t2831 = ct{251};
t2834 = ct{252};
t2835 = ct{253};
t2838 = ct{254};
t2850 = ct{255};
t2851 = ct{256};
t29 = ct{257};
t2945 = ct{258};
t2950 = ct{259};
t2953 = ct{260};
t2955 = ct{261};
t2957 = ct{262};
t2965 = ct{263};
t2966 = ct{264};
t2975 = ct{265};
t2979 = ct{266};
t2990 = ct{267};
t2991 = ct{268};
t2993 = ct{269};
t2994 = ct{270};
t2998 = ct{271};
t30 = ct{272};
t3003 = ct{273};
t3009 = ct{274};
t3015 = ct{275};
t3017 = ct{276};
t3022 = ct{277};
t3027 = ct{278};
t3030 = ct{279};
t3036 = ct{280};
t3043 = ct{281};
t3045 = ct{282};
t3047 = ct{283};
t3054 = ct{284};
t3055 = ct{285};
t3057 = ct{286};
t3058 = ct{287};
t3063 = ct{288};
t3064 = ct{289};
t3068 = ct{290};
t3072 = ct{291};
t3079 = ct{292};
t3080 = ct{293};
t3096 = ct{294};
t3097 = ct{295};
t31 = ct{296};
t3109 = ct{297};
t3117 = ct{298};
t3118 = ct{299};
t3121 = ct{300};
t3122 = ct{301};
t3126 = ct{302};
t3129 = ct{303};
t313 = ct{304};
t3130 = ct{305};
t3131 = ct{306};
t3132 = ct{307};
t3133 = ct{308};
t3135 = ct{309};
t3136 = ct{310};
t314 = ct{311};
t3140 = ct{312};
t3141 = ct{313};
t3142 = ct{314};
t3143 = ct{315};
t3145 = ct{316};
t3148 = ct{317};
t3156 = ct{318};
t3157 = ct{319};
t3158 = ct{320};
t3165 = ct{321};
t3167 = ct{322};
t3171 = ct{323};
t3173 = ct{324};
t3185 = ct{325};
t3187 = ct{326};
t3188 = ct{327};
t3189 = ct{328};
t3190 = ct{329};
t3192 = ct{330};
t3193 = ct{331};
t3194 = ct{332};
t3195 = ct{333};
t3196 = ct{334};
t3199 = ct{335};
t32 = ct{336};
t3200 = ct{337};
t3201 = ct{338};
t3202 = ct{339};
t3203 = ct{340};
t3205 = ct{341};
t3206 = ct{342};
t3208 = ct{343};
t3209 = ct{344};
t321 = ct{345};
t3211 = ct{346};
t3213 = ct{347};
t3216 = ct{348};
t3217 = ct{349};
t3221 = ct{350};
t3232 = ct{351};
t3235 = ct{352};
t3236 = ct{353};
t3237 = ct{354};
t3238 = ct{355};
t3239 = ct{356};
t3242 = ct{357};
t3252 = ct{358};
t3257 = ct{359};
t3261 = ct{360};
t3267 = ct{361};
t3268 = ct{362};
t3270 = ct{363};
t3276 = ct{364};
t3277 = ct{365};
t3279 = ct{366};
t3283 = ct{367};
t329 = ct{368};
t3290 = ct{369};
t3297 = ct{370};
t3298 = ct{371};
t3299 = ct{372};
t33 = ct{373};
t3303 = ct{374};
t3312 = ct{375};
t3313 = ct{376};
t3314 = ct{377};
t3315 = ct{378};
t3318 = ct{379};
t332 = ct{380};
t3322 = ct{381};
t3324 = ct{382};
t3326 = ct{383};
t3328 = ct{384};
t3329 = ct{385};
t3334 = ct{386};
t3336 = ct{387};
t3337 = ct{388};
t3340 = ct{389};
t3344 = ct{390};
t3345 = ct{391};
t3346 = ct{392};
t3347 = ct{393};
t335 = ct{394};
t3351 = ct{395};
t3354 = ct{396};
t3359 = ct{397};
t3363 = ct{398};
t3364 = ct{399};
t3367 = ct{400};
t3369 = ct{401};
t3370 = ct{402};
t3386 = ct{403};
t3395 = ct{404};
t3396 = ct{405};
t34 = ct{406};
t3405 = ct{407};
t3409 = ct{408};
t3415 = ct{409};
t3416 = ct{410};
t3420 = ct{411};
t3421 = ct{412};
t3423 = ct{413};
t3426 = ct{414};
t3428 = ct{415};
t3430 = ct{416};
t3431 = ct{417};
t3432 = ct{418};
t3434 = ct{419};
t3435 = ct{420};
t3439 = ct{421};
t3443 = ct{422};
t3444 = ct{423};
t3446 = ct{424};
t3448 = ct{425};
t3451 = ct{426};
t3455 = ct{427};
t346 = ct{428};
t3460 = ct{429};
t3461 = ct{430};
t3462 = ct{431};
t3463 = ct{432};
t3465 = ct{433};
t3468 = ct{434};
t3469 = ct{435};
t3471 = ct{436};
t3474 = ct{437};
t3480 = ct{438};
t3482 = ct{439};
t3483 = ct{440};
t3488 = ct{441};
t3489 = ct{442};
t3490 = ct{443};
t3492 = ct{444};
t3495 = ct{445};
t3496 = ct{446};
t3498 = ct{447};
t3499 = ct{448};
t35 = ct{449};
t350 = ct{450};
t3500 = ct{451};
t3502 = ct{452};
t3503 = ct{453};
t3512 = ct{454};
t3517 = ct{455};
t3524 = ct{456};
t3537 = ct{457};
t354 = ct{458};
t3541 = ct{459};
t3543 = ct{460};
t3545 = ct{461};
t3546 = ct{462};
t3547 = ct{463};
t3549 = ct{464};
t3550 = ct{465};
t3551 = ct{466};
t3552 = ct{467};
t3554 = ct{468};
t3558 = ct{469};
t3561 = ct{470};
t3563 = ct{471};
t3566 = ct{472};
t358 = ct{473};
t3582 = ct{474};
t3588 = ct{475};
t3589 = ct{476};
t359 = ct{477};
t3590 = ct{478};
t3591 = ct{479};
t3592 = ct{480};
t3597 = ct{481};
t36 = ct{482};
t3603 = ct{483};
t3606 = ct{484};
t3607 = ct{485};
t3608 = ct{486};
t3609 = ct{487};
t3610 = ct{488};
t3611 = ct{489};
t3614 = ct{490};
t3617 = ct{491};
t3621 = ct{492};
t3624 = ct{493};
t3637 = ct{494};
t3638 = ct{495};
t3639 = ct{496};
t3640 = ct{497};
t3641 = ct{498};
t3642 = ct{499};
t3643 = ct{500};
t3649 = ct{501};
t3652 = ct{502};
t3653 = ct{503};
t3654 = ct{504};
t3655 = ct{505};
t3656 = ct{506};
t3658 = ct{507};
t3659 = ct{508};
t366 = ct{509};
t3660 = ct{510};
t3662 = ct{511};
t3664 = ct{512};
t3670 = ct{513};
t3678 = ct{514};
t3684 = ct{515};
t3688 = ct{516};
t3689 = ct{517};
t3690 = ct{518};
t3692 = ct{519};
t3693 = ct{520};
t3695 = ct{521};
t3696 = ct{522};
t3697 = ct{523};
t3699 = ct{524};
t3701 = ct{525};
t3702 = ct{526};
t3703 = ct{527};
t3704 = ct{528};
t3705 = ct{529};
t3706 = ct{530};
t3707 = ct{531};
t3708 = ct{532};
t3709 = ct{533};
t3710 = ct{534};
t3712 = ct{535};
t3713 = ct{536};
t3716 = ct{537};
t3717 = ct{538};
t3728 = ct{539};
t3729 = ct{540};
t3731 = ct{541};
t3732 = ct{542};
t3735 = ct{543};
t3736 = ct{544};
t3737 = ct{545};
t3738 = ct{546};
t3739 = ct{547};
t3741 = ct{548};
t3746 = ct{549};
t3747 = ct{550};
t3752 = ct{551};
t3755 = ct{552};
t3759 = ct{553};
t3765 = ct{554};
t3766 = ct{555};
t3770 = ct{556};
t3771 = ct{557};
t3772 = ct{558};
t3774 = ct{559};
t3775 = ct{560};
t3777 = ct{561};
t3779 = ct{562};
t378 = ct{563};
t3781 = ct{564};
t3782 = ct{565};
t3783 = ct{566};
t3784 = ct{567};
t3785 = ct{568};
t3786 = ct{569};
t3788 = ct{570};
t3789 = ct{571};
t3790 = ct{572};
t3791 = ct{573};
t3792 = ct{574};
t3793 = ct{575};
t3794 = ct{576};
t3795 = ct{577};
t3796 = ct{578};
t3797 = ct{579};
t3798 = ct{580};
t38 = ct{581};
t3800 = ct{582};
t3801 = ct{583};
t3802 = ct{584};
t3804 = ct{585};
t3805 = ct{586};
t3808 = ct{587};
t3809 = ct{588};
t3810 = ct{589};
t3817 = ct{590};
t3818 = ct{591};
t382 = ct{592};
t3820 = ct{593};
t3821 = ct{594};
t3823 = ct{595};
t3824 = ct{596};
t3826 = ct{597};
t3827 = ct{598};
t3828 = ct{599};
t3830 = ct{600};
t3832 = ct{601};
t3833 = ct{602};
t3835 = ct{603};
t3840 = ct{604};
t3843 = ct{605};
t3844 = ct{606};
t3845 = ct{607};
t3846 = ct{608};
t3848 = ct{609};
t3850 = ct{610};
t3851 = ct{611};
t3855 = ct{612};
t3856 = ct{613};
t3857 = ct{614};
t3862 = ct{615};
t3863 = ct{616};
t387 = ct{617};
t3873 = ct{618};
t3876 = ct{619};
t3877 = ct{620};
t3878 = ct{621};
t3879 = ct{622};
t3880 = ct{623};
t3889 = ct{624};
t3890 = ct{625};
t3891 = ct{626};
t3893 = ct{627};
t3895 = ct{628};
t3896 = ct{629};
t3897 = ct{630};
t3898 = ct{631};
t39 = ct{632};
t3901 = ct{633};
t3902 = ct{634};
t3903 = ct{635};
t3906 = ct{636};
t3908 = ct{637};
t3910 = ct{638};
t3913 = ct{639};
t3915 = ct{640};
t3924 = ct{641};
t3925 = ct{642};
t3926 = ct{643};
t3931 = ct{644};
t3934 = ct{645};
t3937 = ct{646};
t3943 = ct{647};
t3951 = ct{648};
t3961 = ct{649};
t3967 = ct{650};
t3968 = ct{651};
t3974 = ct{652};
t3975 = ct{653};
t3976 = ct{654};
t3977 = ct{655};
t3980 = ct{656};
t3985 = ct{657};
t3991 = ct{658};
t3993 = ct{659};
t4001 = ct{660};
t4006 = ct{661};
t4008 = ct{662};
t4018 = ct{663};
t4019 = ct{664};
t4026 = ct{665};
t4030 = ct{666};
t4031 = ct{667};
t4032 = ct{668};
t4035 = ct{669};
t4039 = ct{670};
t4041 = ct{671};
t4045 = ct{672};
t4047 = ct{673};
t4049 = ct{674};
t4051 = ct{675};
t4053 = ct{676};
t4054 = ct{677};
t4065 = ct{678};
t4072 = ct{679};
t4073 = ct{680};
t4074 = ct{681};
t4075 = ct{682};
t410 = ct{683};
t4100 = ct{684};
t4109 = ct{685};
t4110 = ct{686};
t4114 = ct{687};
t4115 = ct{688};
t4118 = ct{689};
t4124 = ct{690};
t4127 = ct{691};
t4128 = ct{692};
t4129 = ct{693};
t4144 = ct{694};
t4146 = ct{695};
t4147 = ct{696};
t4151 = ct{697};
t4153 = ct{698};
t4154 = ct{699};
t4157 = ct{700};
t4158 = ct{701};
t4160 = ct{702};
t4163 = ct{703};
t4165 = ct{704};
t4171 = ct{705};
t4172 = ct{706};
t4183 = ct{707};
t4184 = ct{708};
t4185 = ct{709};
t4186 = ct{710};
t4187 = ct{711};
t4190 = ct{712};
t4193 = ct{713};
t4198 = ct{714};
t42 = ct{715};
t4201 = ct{716};
t4205 = ct{717};
t4207 = ct{718};
t4208 = ct{719};
t4213 = ct{720};
t4215 = ct{721};
t4236 = ct{722};
t4240 = ct{723};
t4244 = ct{724};
t4260 = ct{725};
t4261 = ct{726};
t4263 = ct{727};
t4270 = ct{728};
t4272 = ct{729};
t4273 = ct{730};
t4274 = ct{731};
t4275 = ct{732};
t4276 = ct{733};
t4277 = ct{734};
t4278 = ct{735};
t4280 = ct{736};
t4281 = ct{737};
t4282 = ct{738};
t4286 = ct{739};
t4287 = ct{740};
t4288 = ct{741};
t4289 = ct{742};
t4290 = ct{743};
t4291 = ct{744};
t4292 = ct{745};
t4299 = ct{746};
t43 = ct{747};
t4300 = ct{748};
t4301 = ct{749};
t4303 = ct{750};
t4307 = ct{751};
t4308 = ct{752};
t4310 = ct{753};
t4312 = ct{754};
t4313 = ct{755};
t4314 = ct{756};
t4318 = ct{757};
t4321 = ct{758};
t4324 = ct{759};
t4325 = ct{760};
t4326 = ct{761};
t4330 = ct{762};
t4332 = ct{763};
t4334 = ct{764};
t4337 = ct{765};
t4339 = ct{766};
t4341 = ct{767};
t4342 = ct{768};
t4343 = ct{769};
t4344 = ct{770};
t4345 = ct{771};
t4346 = ct{772};
t4352 = ct{773};
t4356 = ct{774};
t4358 = ct{775};
t4359 = ct{776};
t4361 = ct{777};
t4364 = ct{778};
t4368 = ct{779};
t4371 = ct{780};
t4372 = ct{781};
t4373 = ct{782};
t4375 = ct{783};
t4406 = ct{784};
t4413 = ct{785};
t4415 = ct{786};
t4416 = ct{787};
t4417 = ct{788};
t4427 = ct{789};
t4429 = ct{790};
t4430 = ct{791};
t4432 = ct{792};
t4435 = ct{793};
t4441 = ct{794};
t4450 = ct{795};
t4451 = ct{796};
t4458 = ct{797};
t4459 = ct{798};
t4461 = ct{799};
t4464 = ct{800};
t4465 = ct{801};
t4467 = ct{802};
t4468 = ct{803};
t4470 = ct{804};
t4476 = ct{805};
t4479 = ct{806};
t4482 = ct{807};
t4486 = ct{808};
t4488 = ct{809};
t4489 = ct{810};
t4493 = ct{811};
t4494 = ct{812};
t4495 = ct{813};
t4496 = ct{814};
t4497 = ct{815};
t4501 = ct{816};
t4502 = ct{817};
t4504 = ct{818};
t4515 = ct{819};
t4518 = ct{820};
t4520 = ct{821};
t4522 = ct{822};
t4532 = ct{823};
t4534 = ct{824};
t4537 = ct{825};
t4545 = ct{826};
t4553 = ct{827};
t4556 = ct{828};
t4559 = ct{829};
t4562 = ct{830};
t4563 = ct{831};
t4567 = ct{832};
t4570 = ct{833};
t4571 = ct{834};
t4573 = ct{835};
t4574 = ct{836};
t4576 = ct{837};
t4577 = ct{838};
t4578 = ct{839};
t4580 = ct{840};
t4582 = ct{841};
t4583 = ct{842};
t4586 = ct{843};
t4588 = ct{844};
t4592 = ct{845};
t4594 = ct{846};
t4597 = ct{847};
t4598 = ct{848};
t4599 = ct{849};
t46 = ct{850};
t4603 = ct{851};
t4604 = ct{852};
t4606 = ct{853};
t4615 = ct{854};
t4617 = ct{855};
t4618 = ct{856};
t4619 = ct{857};
t4622 = ct{858};
t4623 = ct{859};
t4624 = ct{860};
t4628 = ct{861};
t4631 = ct{862};
t4634 = ct{863};
t4635 = ct{864};
t4638 = ct{865};
t4639 = ct{866};
t4642 = ct{867};
t4643 = ct{868};
t4644 = ct{869};
t4645 = ct{870};
t4651 = ct{871};
t4652 = ct{872};
t4654 = ct{873};
t4656 = ct{874};
t4657 = ct{875};
t4658 = ct{876};
t4660 = ct{877};
t4662 = ct{878};
t4663 = ct{879};
t4665 = ct{880};
t4673 = ct{881};
t4675 = ct{882};
t4676 = ct{883};
t4677 = ct{884};
t4678 = ct{885};
t4680 = ct{886};
t4683 = ct{887};
t4686 = ct{888};
t4688 = ct{889};
t4690 = ct{890};
t4691 = ct{891};
t4692 = ct{892};
t4694 = ct{893};
t4696 = ct{894};
t4697 = ct{895};
t4698 = ct{896};
t4699 = ct{897};
t47 = ct{898};
t4701 = ct{899};
t4703 = ct{900};
t4704 = ct{901};
t4705 = ct{902};
t4708 = ct{903};
t4709 = ct{904};
t4712 = ct{905};
t4713 = ct{906};
t4716 = ct{907};
t4719 = ct{908};
t4720 = ct{909};
t4722 = ct{910};
t4724 = ct{911};
t4725 = ct{912};
t4727 = ct{913};
t4728 = ct{914};
t4730 = ct{915};
t4737 = ct{916};
t4738 = ct{917};
t4739 = ct{918};
t4741 = ct{919};
t4743 = ct{920};
t4744 = ct{921};
t4746 = ct{922};
t4751 = ct{923};
t4757 = ct{924};
t4760 = ct{925};
t4761 = ct{926};
t4762 = ct{927};
t4763 = ct{928};
t4764 = ct{929};
t4767 = ct{930};
t4771 = ct{931};
t4773 = ct{932};
t4776 = ct{933};
t4777 = ct{934};
t4778 = ct{935};
t4779 = ct{936};
t4783 = ct{937};
t4785 = ct{938};
t4786 = ct{939};
t4787 = ct{940};
t4790 = ct{941};
t4791 = ct{942};
t4795 = ct{943};
t4796 = ct{944};
t4799 = ct{945};
t4801 = ct{946};
t4808 = ct{947};
t4809 = ct{948};
t4810 = ct{949};
t4811 = ct{950};
t4813 = ct{951};
t4814 = ct{952};
t4816 = ct{953};
t4817 = ct{954};
t4818 = ct{955};
t4819 = ct{956};
t4822 = ct{957};
t4823 = ct{958};
t4826 = ct{959};
t4827 = ct{960};
t4828 = ct{961};
t4829 = ct{962};
t4832 = ct{963};
t4833 = ct{964};
t4835 = ct{965};
t4838 = ct{966};
t4843 = ct{967};
t4844 = ct{968};
t4845 = ct{969};
t4846 = ct{970};
t4847 = ct{971};
t4848 = ct{972};
t4849 = ct{973};
t4850 = ct{974};
t4851 = ct{975};
t4852 = ct{976};
t4853 = ct{977};
t4854 = ct{978};
t4856 = ct{979};
t4857 = ct{980};
t4858 = ct{981};
t4859 = ct{982};
t4863 = ct{983};
t4865 = ct{984};
t4866 = ct{985};
t4867 = ct{986};
t4870 = ct{987};
t4872 = ct{988};
t4874 = ct{989};
t4875 = ct{990};
t4876 = ct{991};
t4879 = ct{992};
t4880 = ct{993};
t4881 = ct{994};
t4886 = ct{995};
t4887 = ct{996};
t4888 = ct{997};
t4889 = ct{998};
t4892 = ct{999};
t4893 = ct{1000};
t4895 = ct{1001};
t4896 = ct{1002};
t4898 = ct{1003};
t4901 = ct{1004};
t4902 = ct{1005};
t4903 = ct{1006};
t4904 = ct{1007};
t4905 = ct{1008};
t4906 = ct{1009};
t4907 = ct{1010};
t4908 = ct{1011};
t4909 = ct{1012};
t4910 = ct{1013};
t4911 = ct{1014};
t4912 = ct{1015};
t4913 = ct{1016};
t4914 = ct{1017};
t4915 = ct{1018};
t4920 = ct{1019};
t4923 = ct{1020};
t4924 = ct{1021};
t4925 = ct{1022};
t4926 = ct{1023};
t4927 = ct{1024};
t4928 = ct{1025};
t4933 = ct{1026};
t4935 = ct{1027};
t4936 = ct{1028};
t4937 = ct{1029};
t4938 = ct{1030};
t4940 = ct{1031};
t4943 = ct{1032};
t4946 = ct{1033};
t4948 = ct{1034};
t4949 = ct{1035};
t4950 = ct{1036};
t4952 = ct{1037};
t4953 = ct{1038};
t4955 = ct{1039};
t4957 = ct{1040};
t4958 = ct{1041};
t4959 = ct{1042};
t4960 = ct{1043};
t4962 = ct{1044};
t4965 = ct{1045};
t4967 = ct{1046};
t4969 = ct{1047};
t4970 = ct{1048};
t4971 = ct{1049};
t4972 = ct{1050};
t4973 = ct{1051};
t4974 = ct{1052};
t4976 = ct{1053};
t4977 = ct{1054};
t4978 = ct{1055};
t4979 = ct{1056};
t4981 = ct{1057};
t4982 = ct{1058};
t4983 = ct{1059};
t4989 = ct{1060};
t4992 = ct{1061};
t4993 = ct{1062};
t4994 = ct{1063};
t4997 = ct{1064};
t4998 = ct{1065};
t50 = ct{1066};
t5001 = ct{1067};
t5003 = ct{1068};
t5004 = ct{1069};
t5005 = ct{1070};
t5007 = ct{1071};
t5009 = ct{1072};
t5010 = ct{1073};
t5011 = ct{1074};
t5012 = ct{1075};
t5013 = ct{1076};
t5014 = ct{1077};
t5016 = ct{1078};
t5021 = ct{1079};
t5023 = ct{1080};
t5025 = ct{1081};
t5026 = ct{1082};
t5027 = ct{1083};
t5028 = ct{1084};
t5032 = ct{1085};
t5033 = ct{1086};
t5034 = ct{1087};
t5035 = ct{1088};
t5036 = ct{1089};
t5037 = ct{1090};
t5038 = ct{1091};
t5041 = ct{1092};
t5042 = ct{1093};
t5043 = ct{1094};
t5045 = ct{1095};
t5046 = ct{1096};
t5047 = ct{1097};
t5049 = ct{1098};
t5051 = ct{1099};
t5052 = ct{1100};
t5053 = ct{1101};
t5057 = ct{1102};
t5059 = ct{1103};
t5061 = ct{1104};
t5062 = ct{1105};
t5063 = ct{1106};
t5064 = ct{1107};
t5070 = ct{1108};
t5072 = ct{1109};
t5074 = ct{1110};
t5075 = ct{1111};
t5076 = ct{1112};
t5077 = ct{1113};
t5079 = ct{1114};
t5080 = ct{1115};
t5081 = ct{1116};
t5082 = ct{1117};
t5083 = ct{1118};
t5084 = ct{1119};
t5085 = ct{1120};
t5086 = ct{1121};
t5087 = ct{1122};
t5088 = ct{1123};
t5089 = ct{1124};
t5090 = ct{1125};
t5091 = ct{1126};
t5093 = ct{1127};
t5096 = ct{1128};
t5097 = ct{1129};
t5098 = ct{1130};
t5101 = ct{1131};
t5103 = ct{1132};
t5105 = ct{1133};
t5106 = ct{1134};
t5108 = ct{1135};
t5109 = ct{1136};
t5111 = ct{1137};
t5112 = ct{1138};
t5113 = ct{1139};
t5114 = ct{1140};
t5116 = ct{1141};
t5117 = ct{1142};
t5118 = ct{1143};
t5119 = ct{1144};
t5120 = ct{1145};
t5121 = ct{1146};
t5123 = ct{1147};
t5124 = ct{1148};
t5125 = ct{1149};
t5126 = ct{1150};
t5127 = ct{1151};
t5133 = ct{1152};
t5135 = ct{1153};
t5136 = ct{1154};
t5137 = ct{1155};
t5138 = ct{1156};
t5139 = ct{1157};
t5141 = ct{1158};
t5142 = ct{1159};
t5147 = ct{1160};
t5148 = ct{1161};
t5149 = ct{1162};
t5150 = ct{1163};
t5152 = ct{1164};
t5153 = ct{1165};
t5154 = ct{1166};
t5155 = ct{1167};
t5156 = ct{1168};
t5158 = ct{1169};
t5159 = ct{1170};
t5161 = ct{1171};
t5162 = ct{1172};
t5163 = ct{1173};
t5164 = ct{1174};
t5165 = ct{1175};
t5166 = ct{1176};
t5167 = ct{1177};
t5169 = ct{1178};
t5171 = ct{1179};
t5173 = ct{1180};
t5176 = ct{1181};
t5177 = ct{1182};
t5178 = ct{1183};
t5180 = ct{1184};
t5181 = ct{1185};
t5185 = ct{1186};
t5187 = ct{1187};
t5188 = ct{1188};
t5189 = ct{1189};
t5191 = ct{1190};
t5192 = ct{1191};
t5193 = ct{1192};
t5194 = ct{1193};
t5195 = ct{1194};
t5196 = ct{1195};
t5197 = ct{1196};
t5198 = ct{1197};
t5199 = ct{1198};
t5200 = ct{1199};
t5201 = ct{1200};
t5202 = ct{1201};
t5203 = ct{1202};
t5205 = ct{1203};
t5206 = ct{1204};
t5207 = ct{1205};
t5208 = ct{1206};
t5211 = ct{1207};
t5212 = ct{1208};
t5213 = ct{1209};
t5214 = ct{1210};
t5215 = ct{1211};
t5216 = ct{1212};
t5219 = ct{1213};
t5222 = ct{1214};
t5223 = ct{1215};
t5234 = ct{1216};
t5235 = ct{1217};
t5236 = ct{1218};
t5237 = ct{1219};
t5240 = ct{1220};
t5241 = ct{1221};
t5243 = ct{1222};
t5244 = ct{1223};
t5245 = ct{1224};
t5246 = ct{1225};
t5247 = ct{1226};
t5248 = ct{1227};
t5249 = ct{1228};
t5251 = ct{1229};
t5254 = ct{1230};
t5255 = ct{1231};
t5256 = ct{1232};
t5257 = ct{1233};
t5258 = ct{1234};
t5259 = ct{1235};
t5261 = ct{1236};
t5262 = ct{1237};
t5263 = ct{1238};
t5264 = ct{1239};
t5265 = ct{1240};
t5267 = ct{1241};
t5269 = ct{1242};
t5270 = ct{1243};
t5271 = ct{1244};
t5272 = ct{1245};
t5275 = ct{1246};
t5276 = ct{1247};
t5277 = ct{1248};
t5278 = ct{1249};
t5279 = ct{1250};
t5280 = ct{1251};
t5281 = ct{1252};
t5283 = ct{1253};
t5284 = ct{1254};
t5286 = ct{1255};
t5287 = ct{1256};
t5289 = ct{1257};
t5290 = ct{1258};
t5291 = ct{1259};
t5292 = ct{1260};
t5294 = ct{1261};
t5295 = ct{1262};
t5296 = ct{1263};
t5297 = ct{1264};
t5298 = ct{1265};
t5300 = ct{1266};
t5301 = ct{1267};
t5302 = ct{1268};
t5303 = ct{1269};
t5304 = ct{1270};
t5305 = ct{1271};
t5306 = ct{1272};
t5308 = ct{1273};
t5309 = ct{1274};
t5310 = ct{1275};
t5312 = ct{1276};
t5313 = ct{1277};
t5317 = ct{1278};
t5326 = ct{1279};
t5327 = ct{1280};
t5328 = ct{1281};
t5331 = ct{1282};
t5332 = ct{1283};
t5333 = ct{1284};
t5335 = ct{1285};
t5336 = ct{1286};
t5337 = ct{1287};
t5338 = ct{1288};
t5339 = ct{1289};
t5340 = ct{1290};
t5341 = ct{1291};
t5342 = ct{1292};
t5343 = ct{1293};
t5344 = ct{1294};
t5345 = ct{1295};
t5346 = ct{1296};
t5348 = ct{1297};
t5350 = ct{1298};
t5352 = ct{1299};
t5353 = ct{1300};
t5356 = ct{1301};
t5357 = ct{1302};
t5358 = ct{1303};
t5359 = ct{1304};
t5361 = ct{1305};
t5362 = ct{1306};
t5363 = ct{1307};
t5364 = ct{1308};
t5366 = ct{1309};
t5369 = ct{1310};
t5370 = ct{1311};
t5372 = ct{1312};
t5373 = ct{1313};
t5374 = ct{1314};
t5376 = ct{1315};
t5379 = ct{1316};
t5381 = ct{1317};
t5382 = ct{1318};
t5383 = ct{1319};
t5384 = ct{1320};
t5385 = ct{1321};
t5386 = ct{1322};
t5387 = ct{1323};
t5389 = ct{1324};
t5390 = ct{1325};
t5391 = ct{1326};
t5392 = ct{1327};
t5393 = ct{1328};
t5395 = ct{1329};
t5399 = ct{1330};
t5400 = ct{1331};
t5401 = ct{1332};
t5402 = ct{1333};
t5403 = ct{1334};
t5404 = ct{1335};
t5405 = ct{1336};
t5406 = ct{1337};
t5410 = ct{1338};
t5411 = ct{1339};
t5412 = ct{1340};
t5413 = ct{1341};
t5415 = ct{1342};
t5416 = ct{1343};
t5419 = ct{1344};
t5421 = ct{1345};
t5422 = ct{1346};
t5425 = ct{1347};
t5426 = ct{1348};
t5433 = ct{1349};
t5434 = ct{1350};
t5436 = ct{1351};
t5437 = ct{1352};
t5438 = ct{1353};
t5439 = ct{1354};
t5440 = ct{1355};
t5441 = ct{1356};
t5442 = ct{1357};
t5443 = ct{1358};
t5444 = ct{1359};
t5445 = ct{1360};
t5446 = ct{1361};
t5448 = ct{1362};
t5449 = ct{1363};
t5451 = ct{1364};
t5452 = ct{1365};
t5453 = ct{1366};
t5456 = ct{1367};
t5457 = ct{1368};
t5458 = ct{1369};
t5459 = ct{1370};
t5460 = ct{1371};
t5461 = ct{1372};
t5462 = ct{1373};
t5464 = ct{1374};
t5465 = ct{1375};
t5466 = ct{1376};
t5467 = ct{1377};
t5470 = ct{1378};
t5472 = ct{1379};
t5473 = ct{1380};
t5474 = ct{1381};
t5477 = ct{1382};
t5478 = ct{1383};
t5480 = ct{1384};
t5481 = ct{1385};
t5483 = ct{1386};
t5484 = ct{1387};
t5486 = ct{1388};
t5487 = ct{1389};
t5488 = ct{1390};
t5489 = ct{1391};
t5491 = ct{1392};
t5493 = ct{1393};
t5494 = ct{1394};
t5495 = ct{1395};
t5497 = ct{1396};
t5499 = ct{1397};
t5500 = ct{1398};
t5501 = ct{1399};
t5502 = ct{1400};
t5503 = ct{1401};
t5504 = ct{1402};
t5505 = ct{1403};
t5506 = ct{1404};
t5507 = ct{1405};
t5508 = ct{1406};
t5509 = ct{1407};
t5510 = ct{1408};
t5511 = ct{1409};
t5512 = ct{1410};
t5513 = ct{1411};
t5514 = ct{1412};
t5516 = ct{1413};
t5517 = ct{1414};
t5519 = ct{1415};
t5520 = ct{1416};
t5521 = ct{1417};
t5522 = ct{1418};
t5523 = ct{1419};
t5524 = ct{1420};
t5528 = ct{1421};
t5529 = ct{1422};
t5531 = ct{1423};
t5532 = ct{1424};
t5534 = ct{1425};
t5535 = ct{1426};
t5536 = ct{1427};
t5537 = ct{1428};
t5538 = ct{1429};
t5539 = ct{1430};
t5540 = ct{1431};
t5542 = ct{1432};
t5543 = ct{1433};
t5544 = ct{1434};
t5545 = ct{1435};
t5548 = ct{1436};
t5549 = ct{1437};
t5550 = ct{1438};
t5553 = ct{1439};
t5554 = ct{1440};
t5555 = ct{1441};
t5556 = ct{1442};
t5557 = ct{1443};
t5558 = ct{1444};
t5560 = ct{1445};
t5563 = ct{1446};
t5564 = ct{1447};
t5565 = ct{1448};
t5567 = ct{1449};
t5568 = ct{1450};
t5569 = ct{1451};
t5570 = ct{1452};
t5572 = ct{1453};
t5573 = ct{1454};
t5574 = ct{1455};
t5575 = ct{1456};
t5576 = ct{1457};
t5577 = ct{1458};
t5578 = ct{1459};
t5579 = ct{1460};
t5581 = ct{1461};
t5583 = ct{1462};
t5585 = ct{1463};
t5586 = ct{1464};
t5587 = ct{1465};
t5588 = ct{1466};
t5589 = ct{1467};
t5590 = ct{1468};
t5591 = ct{1469};
t5592 = ct{1470};
t5593 = ct{1471};
t5594 = ct{1472};
t5596 = ct{1473};
t5597 = ct{1474};
t5598 = ct{1475};
t5599 = ct{1476};
t56 = ct{1477};
t5600 = ct{1478};
t5601 = ct{1479};
t5602 = ct{1480};
t5603 = ct{1481};
t5604 = ct{1482};
t5605 = ct{1483};
t5606 = ct{1484};
t5607 = ct{1485};
t5608 = ct{1486};
t5609 = ct{1487};
t5611 = ct{1488};
t5612 = ct{1489};
t5613 = ct{1490};
t5614 = ct{1491};
t5615 = ct{1492};
t5616 = ct{1493};
t5618 = ct{1494};
t5619 = ct{1495};
t5622 = ct{1496};
t5623 = ct{1497};
t5624 = ct{1498};
t5625 = ct{1499};
t5629 = ct{1500};
t5630 = ct{1501};
t5631 = ct{1502};
t5632 = ct{1503};
t5633 = ct{1504};
t5634 = ct{1505};
t5635 = ct{1506};
t5636 = ct{1507};
t5637 = ct{1508};
t5638 = ct{1509};
t5640 = ct{1510};
t5645 = ct{1511};
t5646 = ct{1512};
t5647 = ct{1513};
t5649 = ct{1514};
t5650 = ct{1515};
t5651 = ct{1516};
t5652 = ct{1517};
t5653 = ct{1518};
t5655 = ct{1519};
t5657 = ct{1520};
t5658 = ct{1521};
t5659 = ct{1522};
t5660 = ct{1523};
t5661 = ct{1524};
t5662 = ct{1525};
t5663 = ct{1526};
t5667 = ct{1527};
t5672 = ct{1528};
t5675 = ct{1529};
t5677 = ct{1530};
t5678 = ct{1531};
t5679 = ct{1532};
t5680 = ct{1533};
t5681 = ct{1534};
t5682 = ct{1535};
t5683 = ct{1536};
t5684 = ct{1537};
t5685 = ct{1538};
t5686 = ct{1539};
t5687 = ct{1540};
t5688 = ct{1541};
t5689 = ct{1542};
t5690 = ct{1543};
t5691 = ct{1544};
t5694 = ct{1545};
t5695 = ct{1546};
t5698 = ct{1547};
t5699 = ct{1548};
t5700 = ct{1549};
t5703 = ct{1550};
t5707 = ct{1551};
t5710 = ct{1552};
t5712 = ct{1553};
t5714 = ct{1554};
t5717 = ct{1555};
t5718 = ct{1556};
t5719 = ct{1557};
t5720 = ct{1558};
t5721 = ct{1559};
t5722 = ct{1560};
t5723 = ct{1561};
t5724 = ct{1562};
t5725 = ct{1563};
t5727 = ct{1564};
t5730 = ct{1565};
t5731 = ct{1566};
t5734 = ct{1567};
t5735 = ct{1568};
t5738 = ct{1569};
t5739 = ct{1570};
t5740 = ct{1571};
t5741 = ct{1572};
t5742 = ct{1573};
t5745 = ct{1574};
t5746 = ct{1575};
t5747 = ct{1576};
t5750 = ct{1577};
t5751 = ct{1578};
t5753 = ct{1579};
t5754 = ct{1580};
t5756 = ct{1581};
t5757 = ct{1582};
t5758 = ct{1583};
t5759 = ct{1584};
t5760 = ct{1585};
t5761 = ct{1586};
t5762 = ct{1587};
t5763 = ct{1588};
t5764 = ct{1589};
t5765 = ct{1590};
t5766 = ct{1591};
t5768 = ct{1592};
t5769 = ct{1593};
t5770 = ct{1594};
t5772 = ct{1595};
t5773 = ct{1596};
t5775 = ct{1597};
t5776 = ct{1598};
t5777 = ct{1599};
t5778 = ct{1600};
t5779 = ct{1601};
t5781 = ct{1602};
t5782 = ct{1603};
t5783 = ct{1604};
t5784 = ct{1605};
t5787 = ct{1606};
t5788 = ct{1607};
t5790 = ct{1608};
t5792 = ct{1609};
t5793 = ct{1610};
t5794 = ct{1611};
t5795 = ct{1612};
t5801 = ct{1613};
t5802 = ct{1614};
t5804 = ct{1615};
t5809 = ct{1616};
t5810 = ct{1617};
t5813 = ct{1618};
t5814 = ct{1619};
t5816 = ct{1620};
t5821 = ct{1621};
t5824 = ct{1622};
t5825 = ct{1623};
t5826 = ct{1624};
t5828 = ct{1625};
t5829 = ct{1626};
t5831 = ct{1627};
t5832 = ct{1628};
t5833 = ct{1629};
t5834 = ct{1630};
t5835 = ct{1631};
t5836 = ct{1632};
t5838 = ct{1633};
t5839 = ct{1634};
t5840 = ct{1635};
t5842 = ct{1636};
t5844 = ct{1637};
t5845 = ct{1638};
t5846 = ct{1639};
t5849 = ct{1640};
t5851 = ct{1641};
t5852 = ct{1642};
t5853 = ct{1643};
t5855 = ct{1644};
t5857 = ct{1645};
t5858 = ct{1646};
t5863 = ct{1647};
t5864 = ct{1648};
t5866 = ct{1649};
t5867 = ct{1650};
t5868 = ct{1651};
t5871 = ct{1652};
t5872 = ct{1653};
t5874 = ct{1654};
t5875 = ct{1655};
t5876 = ct{1656};
t5877 = ct{1657};
t5878 = ct{1658};
t5879 = ct{1659};
t5884 = ct{1660};
t5886 = ct{1661};
t5887 = ct{1662};
t5888 = ct{1663};
t5890 = ct{1664};
t5891 = ct{1665};
t5892 = ct{1666};
t5893 = ct{1667};
t5894 = ct{1668};
t5896 = ct{1669};
t5897 = ct{1670};
t5899 = ct{1671};
t5900 = ct{1672};
t5901 = ct{1673};
t5902 = ct{1674};
t5904 = ct{1675};
t5905 = ct{1676};
t5907 = ct{1677};
t5908 = ct{1678};
t5909 = ct{1679};
t5913 = ct{1680};
t5914 = ct{1681};
t5915 = ct{1682};
t5916 = ct{1683};
t5917 = ct{1684};
t5918 = ct{1685};
t5919 = ct{1686};
t5920 = ct{1687};
t5922 = ct{1688};
t5923 = ct{1689};
t5924 = ct{1690};
t5925 = ct{1691};
t5926 = ct{1692};
t5927 = ct{1693};
t5928 = ct{1694};
t5930 = ct{1695};
t5931 = ct{1696};
t5933 = ct{1697};
t5934 = ct{1698};
t5938 = ct{1699};
t5939 = ct{1700};
t5941 = ct{1701};
t5942 = ct{1702};
t5943 = ct{1703};
t5945 = ct{1704};
t5946 = ct{1705};
t5949 = ct{1706};
t5950 = ct{1707};
t5951 = ct{1708};
t5954 = ct{1709};
t5955 = ct{1710};
t5959 = ct{1711};
t5960 = ct{1712};
t5963 = ct{1713};
t5965 = ct{1714};
t5966 = ct{1715};
t5967 = ct{1716};
t5968 = ct{1717};
t5971 = ct{1718};
t5973 = ct{1719};
t5974 = ct{1720};
t5975 = ct{1721};
t5978 = ct{1722};
t5979 = ct{1723};
t5980 = ct{1724};
t5981 = ct{1725};
t5983 = ct{1726};
t5984 = ct{1727};
t5985 = ct{1728};
t5990 = ct{1729};
t5992 = ct{1730};
t5993 = ct{1731};
t5996 = ct{1732};
t5998 = ct{1733};
t60 = ct{1734};
t6001 = ct{1735};
t6004 = ct{1736};
t6005 = ct{1737};
t6006 = ct{1738};
t6008 = ct{1739};
t6011 = ct{1740};
t6013 = ct{1741};
t6014 = ct{1742};
t6015 = ct{1743};
t6017 = ct{1744};
t6018 = ct{1745};
t6019 = ct{1746};
t6020 = ct{1747};
t6021 = ct{1748};
t6022 = ct{1749};
t6023 = ct{1750};
t6024 = ct{1751};
t6026 = ct{1752};
t6031 = ct{1753};
t6034 = ct{1754};
t6035 = ct{1755};
t6036 = ct{1756};
t6037 = ct{1757};
t6042 = ct{1758};
t6044 = ct{1759};
t6047 = ct{1760};
t6048 = ct{1761};
t6050 = ct{1762};
t6052 = ct{1763};
t6053 = ct{1764};
t6054 = ct{1765};
t6057 = ct{1766};
t6058 = ct{1767};
t6059 = ct{1768};
t6062 = ct{1769};
t6065 = ct{1770};
t6066 = ct{1771};
t6067 = ct{1772};
t6069 = ct{1773};
t6071 = ct{1774};
t6072 = ct{1775};
t6074 = ct{1776};
t6076 = ct{1777};
t6079 = ct{1778};
t6080 = ct{1779};
t6081 = ct{1780};
t6091 = ct{1781};
t6093 = ct{1782};
t6094 = ct{1783};
t6095 = ct{1784};
t6096 = ct{1785};
t6098 = ct{1786};
t6101 = ct{1787};
t6102 = ct{1788};
t6105 = ct{1789};
t6106 = ct{1790};
t6109 = ct{1791};
t6110 = ct{1792};
t6113 = ct{1793};
t6114 = ct{1794};
t6115 = ct{1795};
t6119 = ct{1796};
t6123 = ct{1797};
t6125 = ct{1798};
t6127 = ct{1799};
t6129 = ct{1800};
t6131 = ct{1801};
t6133 = ct{1802};
t6134 = ct{1803};
t6143 = ct{1804};
t6144 = ct{1805};
t6158 = ct{1806};
t6159 = ct{1807};
t6162 = ct{1808};
t6164 = ct{1809};
t6166 = ct{1810};
t6168 = ct{1811};
t6171 = ct{1812};
t6172 = ct{1813};
t6174 = ct{1814};
t6183 = ct{1815};
t6190 = ct{1816};
t6211 = ct{1817};
t6213 = ct{1818};
t6217 = ct{1819};
t6219 = ct{1820};
t6221 = ct{1821};
t6227 = ct{1822};
t6231 = ct{1823};
t6232 = ct{1824};
t6233 = ct{1825};
t6234 = ct{1826};
t6236 = ct{1827};
t6239 = ct{1828};
t6240 = ct{1829};
t6241 = ct{1830};
t6245 = ct{1831};
t6247 = ct{1832};
t6255 = ct{1833};
t6256 = ct{1834};
t6257 = ct{1835};
t6260 = ct{1836};
t6270 = ct{1837};
t6271 = ct{1838};
t6272 = ct{1839};
t6273 = ct{1840};
t6275 = ct{1841};
t6281 = ct{1842};
t6282 = ct{1843};
t6291 = ct{1844};
t6293 = ct{1845};
t6307 = ct{1846};
t6313 = ct{1847};
t6314 = ct{1848};
t6316 = ct{1849};
t6324 = ct{1850};
t6334 = ct{1851};
t6336 = ct{1852};
t6350 = ct{1853};
t6351 = ct{1854};
t6353 = ct{1855};
t6354 = ct{1856};
t6366 = ct{1857};
t6375 = ct{1858};
t6376 = ct{1859};
t6377 = ct{1860};
t6379 = ct{1861};
t6382 = ct{1862};
t6383 = ct{1863};
t6386 = ct{1864};
t6388 = ct{1865};
t6390 = ct{1866};
t6394 = ct{1867};
t6396 = ct{1868};
t6398 = ct{1869};
t640 = ct{1870};
t6402 = ct{1871};
t6405 = ct{1872};
t6407 = ct{1873};
t6408 = ct{1874};
t6411 = ct{1875};
t6412 = ct{1876};
t6417 = ct{1877};
t642 = ct{1878};
t6422 = ct{1879};
t6423 = ct{1880};
t6425 = ct{1881};
t6426 = ct{1882};
t6428 = ct{1883};
t643 = ct{1884};
t6431 = ct{1885};
t6432 = ct{1886};
t6438 = ct{1887};
t6440 = ct{1888};
t6441 = ct{1889};
t6442 = ct{1890};
t6460 = ct{1891};
t6461 = ct{1892};
t6462 = ct{1893};
t6471 = ct{1894};
t6473 = ct{1895};
t6474 = ct{1896};
t6477 = ct{1897};
t6482 = ct{1898};
t6483 = ct{1899};
t6484 = ct{1900};
t6485 = ct{1901};
t6488 = ct{1902};
t649 = ct{1903};
t6491 = ct{1904};
t6508 = ct{1905};
t6512 = ct{1906};
t6513 = ct{1907};
t6515 = ct{1908};
t6517 = ct{1909};
t6523 = ct{1910};
t6524 = ct{1911};
t6525 = ct{1912};
t6526 = ct{1913};
t6527 = ct{1914};
t6528 = ct{1915};
t6530 = ct{1916};
t6531 = ct{1917};
t6537 = ct{1918};
t6538 = ct{1919};
t6549 = ct{1920};
t6559 = ct{1921};
t656 = ct{1922};
t6560 = ct{1923};
t6562 = ct{1924};
t6564 = ct{1925};
t6565 = ct{1926};
t6569 = ct{1927};
t6570 = ct{1928};
t6572 = ct{1929};
t6574 = ct{1930};
t6576 = ct{1931};
t6588 = ct{1932};
t6589 = ct{1933};
t659 = ct{1934};
t6591 = ct{1935};
t6592 = ct{1936};
t6594 = ct{1937};
t6595 = ct{1938};
t6596 = ct{1939};
t660 = ct{1940};
t6601 = ct{1941};
t6602 = ct{1942};
t6606 = ct{1943};
t6607 = ct{1944};
t6615 = ct{1945};
t6622 = ct{1946};
t6623 = ct{1947};
t6624 = ct{1948};
t6625 = ct{1949};
t6651 = ct{1950};
t6652 = ct{1951};
t6654 = ct{1952};
t6656 = ct{1953};
t6658 = ct{1954};
t6659 = ct{1955};
t6660 = ct{1956};
t6661 = ct{1957};
t667 = ct{1958};
t6671 = ct{1959};
t6672 = ct{1960};
t6673 = ct{1961};
t6678 = ct{1962};
t668 = ct{1963};
t6680 = ct{1964};
t6687 = ct{1965};
t6688 = ct{1966};
t669 = ct{1967};
t67 = ct{1968};
t670 = ct{1969};
t6714 = ct{1970};
t6715 = ct{1971};
t674 = ct{1972};
t6745 = ct{1973};
t6747 = ct{1974};
t6750 = ct{1975};
t6751 = ct{1976};
t677 = ct{1977};
t68 = ct{1978};
t6804 = ct{1979};
t6809 = ct{1980};
t681 = ct{1981};
t682 = ct{1982};
t684 = ct{1983};
t685 = ct{1984};
t6858 = ct{1985};
t6859 = ct{1986};
t686 = ct{1987};
t6868 = ct{1988};
t687 = ct{1989};
t6881 = ct{1990};
t6882 = ct{1991};
t6883 = ct{1992};
t6896 = ct{1993};
t6897 = ct{1994};
t6901 = ct{1995};
t6902 = ct{1996};
t6905 = ct{1997};
t6906 = ct{1998};
t6913 = ct{1999};
t6914 = ct{2000};
t6916 = ct{2001};
t6919 = ct{2002};
t6920 = ct{2003};
t6921 = ct{2004};
t6922 = ct{2005};
t694 = ct{2006};
t6965 = ct{2007};
t6966 = ct{2008};
t6974 = ct{2009};
t6976 = ct{2010};
t6978 = ct{2011};
t6979 = ct{2012};
t6980 = ct{2013};
t6984 = ct{2014};
t6987 = ct{2015};
t7003 = ct{2016};
t7005 = ct{2017};
t7007 = ct{2018};
t7010 = ct{2019};
t7014 = ct{2020};
t7016 = ct{2021};
t7018 = ct{2022};
t7020 = ct{2023};
t7021 = ct{2024};
t7035 = ct{2025};
t7054 = ct{2026};
t7055 = ct{2027};
t7059 = ct{2028};
t707 = ct{2029};
t708 = ct{2030};
t7080 = ct{2031};
t7083 = ct{2032};
t7086 = ct{2033};
t7088 = ct{2034};
t7092 = ct{2035};
t7094 = ct{2036};
t7095 = ct{2037};
t7097 = ct{2038};
t7098 = ct{2039};
t71 = ct{2040};
t710 = ct{2041};
t7100 = ct{2042};
t7101 = ct{2043};
t7120 = ct{2044};
t7123 = ct{2045};
t7134 = ct{2046};
t7136 = ct{2047};
t7137 = ct{2048};
t7138 = ct{2049};
t7148 = ct{2050};
t715 = ct{2051};
t7150 = ct{2052};
t7153 = ct{2053};
t7155 = ct{2054};
t7158 = ct{2055};
t7159 = ct{2056};
t716 = ct{2057};
t7160 = ct{2058};
t7162 = ct{2059};
t7164 = ct{2060};
t7166 = ct{2061};
t7169 = ct{2062};
t7170 = ct{2063};
t7197 = ct{2064};
t7199 = ct{2065};
t7201 = ct{2066};
t7204 = ct{2067};
t721 = ct{2068};
t722 = ct{2069};
t724 = ct{2070};
t725 = ct{2071};
t7256 = ct{2072};
t7283 = ct{2073};
t7292 = ct{2074};
t73 = ct{2075};
t7304 = ct{2076};
t7319 = ct{2077};
t7332 = ct{2078};
t7333 = ct{2079};
t736 = ct{2080};
t7385 = ct{2081};
t740 = ct{2082};
t7400 = ct{2083};
t7401 = ct{2084};
t7403 = ct{2085};
t741 = ct{2086};
t749 = ct{2087};
t762 = ct{2088};
t768 = ct{2089};
t777 = ct{2090};
t7784 = ct{2091};
t7790 = ct{2092};
t7827 = ct{2093};
t792 = ct{2094};
t793 = ct{2095};
t8 = ct{2096};
t801 = ct{2097};
t802 = ct{2098};
t808 = ct{2099};
t813 = ct{2100};
t819 = ct{2101};
t821 = ct{2102};
t850 = ct{2103};
t855 = ct{2104};
t874 = ct{2105};
t878 = ct{2106};
t89 = ct{2107};
t9 = ct{2108};
t92 = ct{2109};
t941 = ct{2110};
t948 = ct{2111};
t951 = ct{2112};
t97 = ct{2113};
t7260 = ((t5413+t4146.*(t1861-t3221)).*(t4853.*(t1896-t3239).*7.26735e-3+t2363.*(t684+t685-t710+t724+t1686-t1690+t1700+t1701+t2371+t2698+t2707-t2716+t2719+t3329-t3337-t3351-t3641+t3643+t3655-t3659+t4114+t4115).*7.26735e-3))./2.0;
t7277 = t3017+t3079+t3156+t3167+t4479+t4482+t4532+t4534+t4767+t4771+t5059+t5061;
t7280 = t5245+t5263+t5269+t5271+t5821;
t7281 = t5244+t5267+t5270+t5272+t5824;
t7282 = t5523+t6057+t6069;
et196 = t5052+t5147+t5148+t5350.*(-t2804+t2838+t3109+t17.*(t1456-t2355).*9.3e-7)+t3063.*(t3242-t3554);
et197 = (t4893-t28.*(t1005+t20.*(t1941-t3315+t39.*t1022.*(t855-t878).*2.196325630278387e-1))).*(t2813-t2835+t12.*(t1456-t2355).*1.02e-6+t17.*(t1456-t2355).*9.0e-8);
t7293 = t3216.*(et196+et197).*(-1.0./2.0);
et198 = t5052+t5147+t5148+t5350.*(-t2804+t2838+t3109+t17.*(t1456-t2355).*9.3e-7)+t3063.*(t3242-t3554);
et199 = (t4893-t28.*(t1005+t20.*(t1941-t3315+t39.*t1022.*(t855-t878).*2.196325630278387e-1))).*(t2813-t2835+t12.*(t1456-t2355).*1.02e-6+t17.*(t1456-t2355).*9.0e-8);
t7294 = (t3216.*(et198+et199))./2.0;
t7297 = t2363.*t7292;
et200 = t5052+t5147+t5148+t5350.*(-t2804+t2838+t3109+t17.*(t1456-t2355).*9.3e-7)+t3063.*(t3242-t3554);
et201 = (t4893-t28.*(t1005+t20.*(t1941-t3315+t39.*t1022.*(t855-t878).*2.196325630278387e-1))).*(t2813-t2835+t12.*(t1456-t2355).*1.02e-6+t17.*(t1456-t2355).*9.0e-8);
t7300 = ((et200+et201).*(t1861-t3221))./2.0;
t7309 = -t7292.*(t1896-t3239);
t7310 = t3547.*t7292;
et202 = t5052+t5147+t5148+t5350.*(-t2804+t2838+t3109+t17.*(t1456-t2355).*9.3e-7)+t3063.*(t3242-t3554);
et203 = (t4893-t28.*(t1005+t20.*(t1941-t3315+t39.*t1022.*(t855-t878).*2.196325630278387e-1))).*(t2813-t2835+t12.*(t1456-t2355).*1.02e-6+t17.*(t1456-t2355).*9.0e-8);
t7311 = ((et202+et203).*(t2674-t2676+t3022-t3027))./2.0;
et204 = t5052+t5147+t5148+t5350.*(-t2804+t2838+t3109+t17.*(t1456-t2355).*9.3e-7)+t3063.*(t3242-t3554);
et205 = (t4893-t28.*(t1005+t20.*(t1941-t3315+t39.*t1022.*(t855-t878).*2.196325630278387e-1))).*(t2813-t2835+t12.*(t1456-t2355).*1.02e-6+t17.*(t1456-t2355).*9.0e-8);
t7314 = t3980.*(et204+et205).*(-1.0./2.0);
et206 = t5052+t5147+t5148+t5350.*(-t2804+t2838+t3109+t17.*(t1456-t2355).*9.3e-7)+t3063.*(t3242-t3554);
et207 = (t4893-t28.*(t1005+t20.*(t1941-t3315+t39.*t1022.*(t855-t878).*2.196325630278387e-1))).*(t2813-t2835+t12.*(t1456-t2355).*1.02e-6+t17.*(t1456-t2355).*9.0e-8);
t7315 = (t3980.*(et206+et207))./2.0;
t7322 = -t3055.*(t3131+t3132+t3171+t3446-t4281-t4282-t4301+t4303-t4308+t4310-t4583-t4594+t4623+t4639+t2388.*(t1456-t2355).*4.0e-8+(t3543.*(t1861-t3221))./1.0e+8+(t3500.*(t1896-t3239))./1.0e+8-t11.*t2297.*t2363.*2.4e-7);
t7323 = t3055.*(t3131+t3132+t3171+t3446-t4281-t4282-t4301+t4303-t4308+t4310-t4583-t4594+t4623+t4639+t2388.*(t1456-t2355).*4.0e-8+(t3543.*(t1861-t3221))./1.0e+8+(t3500.*(t1896-t3239))./1.0e+8-t11.*t2297.*t2363.*2.4e-7).*(-1.0./2.0);
et208 = (t4843+t5108+t2307.*(t642+t643-t667+t674+t1587+t1606+t1608+t1609+t2295+t2671+t2683+t2684-t2695+t3279+t3297-t3303+t3597+t3603+t3609-t3614+t4053+t4054)+t2297.*(t2292+t3290+t3524.*1.838876e-2-t3591+t3592+t3611+t16.*(t1861-t3221).*3.131399999999998e-4+t16.*t17.*(t1861-t3221).*9.99471e-3)).*(t2694-t2701+t3036-t3043).*(t1513+t1879+t2598+t2820+t2834+t3117+t3118);
et209 = -3.633675e-3;
t7335 = et208.*et209;
t7337 = (t3242-t3554).*(t3131+t3132+t3171+t3446-t4281-t4282-t4301+t4303-t4308+t4310-t4583-t4594+t4623+t4639+t2388.*(t1456-t2355).*4.0e-8+(t3543.*(t1861-t3221))./1.0e+8+(t3500.*(t1896-t3239))./1.0e+8-t11.*t2297.*t2363.*2.4e-7);
t7338 = -t4026.*(t3131+t3132+t3171+t3446-t4281-t4282-t4301+t4303-t4308+t4310-t4583-t4594+t4623+t4639+t2388.*(t1456-t2355).*4.0e-8+(t3543.*(t1861-t3221))./1.0e+8+(t3500.*(t1896-t3239))./1.0e+8-t11.*t2297.*t2363.*2.4e-7);
t7340 = t4026.*(t3131+t3132+t3171+t3446-t4281-t4282-t4301+t4303-t4308+t4310-t4583-t4594+t4623+t4639+t2388.*(t1456-t2355).*4.0e-8+(t3543.*(t1861-t3221))./1.0e+8+(t3500.*(t1896-t3239))./1.0e+8-t11.*t2297.*t2363.*2.4e-7);
t7341 = t3188+t3189+t3196+t3206+t4786+t4816+t4818+t4822+t5064+t5070+t5075+t5077;
et210 = t2363.*(t2368+t3340+t3582.*1.838876e-2-t3639+t3640+t21.*(t1896-t3239).*1.247162e-2+t27.*(t1896-t3239).*3.131399999999998e-4+t27.*t28.*(t1896-t3239).*9.99471e-3);
et211 = 7.26735e-3;
t7344 = (t4925+t5194+et210.*et211+t2388.*(t684+t685-t710+t724+t1686-t1690+t1700+t1701+t2371+t2698+t2707-t2716+t2719+t3329-t3337-t3351-t3641+t3643+t3655-t3659+t4114+t4115).*7.26735e-3).*(t2674-t2676+t3022-t3027).*(t1488+t1874+t2519+t2740+t2747+t3096+t3097).*(-1.0./2.0);
et212 = t2363.*(t2368+t3340+t3582.*1.838876e-2-t3639+t3640+t21.*(t1896-t3239).*1.247162e-2+t27.*(t1896-t3239).*3.131399999999998e-4+t27.*t28.*(t1896-t3239).*9.99471e-3);
et213 = 7.26735e-3;
t7345 = ((t4925+t5194+et212.*et213+t2388.*(t684+t685-t710+t724+t1686-t1690+t1700+t1701+t2371+t2698+t2707-t2716+t2719+t3329-t3337-t3351-t3641+t3643+t3655-t3659+t4114+t4115).*7.26735e-3).*(t2674-t2676+t3022-t3027).*(t1488+t1874+t2519+t2740+t2747+t3096+t3097))./2.0;
t7348 = -(t1477-t2502).*(-t3185-t3190-t3203+t4786+t4816+t4818+t4822+t5064+t5070+t5075+t5077-t201.*(t1456-t2355).*4.899491877593981e-7);
t7349 = (t1477-t2502).*(-t3185-t3190-t3203+t4786+t4816+t4818+t4822+t5064+t5070+t5075+t5077-t201.*(t1456-t2355).*4.899491877593981e-7).*(-1.0./2.0);
t7357 = (t4853.*(t1896-t3239).*7.26735e-3+t2363.*(t684+t685-t710+t724+t1686-t1690+t1700+t1701+t2371+t2698+t2707-t2716+t2719+t3329-t3337-t3351-t3641+t3643+t3655-t3659+t4114+t4115).*7.26735e-3).*(-t2308+t2378+t2510-t2530-t2975+t2979+t3926+t4144+t4190+t4193+t4863+t4867).*(-1.0./2.0);
t7358 = ((t4853.*(t1896-t3239).*7.26735e-3+t2363.*(t684+t685-t710+t724+t1686-t1690+t1700+t1701+t2371+t2698+t2707-t2716+t2719+t3329-t3337-t3351-t3641+t3643+t3655-t3659+t4114+t4115).*7.26735e-3).*(-t2308+t2378+t2510-t2530-t2975+t2979+t3926+t4144+t4190+t4193+t4863+t4867))./2.0;
t7360 = t6651.*(t4814.*(t1861-t3221)+t2297.*(t642+t643-t667+t674+t1587+t1606+t1608+t1609+t2295+t2671+t2683+t2684-t2695+t3279+t3297-t3303+t3597+t3603+t3609-t3614+t4053+t4054)).*(-1.0./2.0);
t7364 = t4019.*(-t3185-t3190-t3203+t4786+t4816+t4818+t4822+t5064+t5070+t5075+t5077-t201.*(t1456-t2355).*4.899491877593981e-7);
t7366 = t4031.*(-t3185-t3190-t3203+t4786+t4816+t4818+t4822+t5064+t5070+t5075+t5077-t201.*(t1456-t2355).*4.899491877593981e-7);
t7374 = t3326+t3354+t3462+t3465+t4933+t4940+t4946+t4948+t5165+t5173+t5177+t5180;
t7379 = t5461+t5522+t5524+t5532+t6071;
t7380 = t5462+t5528+t5529+t5531+t6072;
t7381 = t4886+t4892+t5215+t5219+t5276+t5277+t5326+t5327;
t7386 = t7385.*(-1.0./2.0);
t7402 = -t7400;
t7435 = (t1477-t2502).*(t5287+t5291-t5328+t5333+t5337-t5340+t4835.*(t2694-t2701+t3036-t3043).*5.7e-7+t4838.*(t2694-t2701+t3036-t3043).*4.0e-8);
t7457 = -t4019.*(t5287+t5291-t5328+t5333+t5337-t5340+t4835.*(t2694-t2701+t3036-t3043).*5.7e-7+t4838.*(t2694-t2701+t3036-t3043).*4.0e-8);
t7458 = t4019.*(t5287+t5291-t5328+t5333+t5337-t5340+t4835.*(t2694-t2701+t3036-t3043).*5.7e-7+t4838.*(t2694-t2701+t3036-t3043).*4.0e-8);
t7459 = -t4031.*(t5287+t5291-t5328+t5333+t5337-t5340+t4835.*(t2694-t2701+t3036-t3043).*5.7e-7+t4838.*(t2694-t2701+t3036-t3043).*4.0e-8);
et214 = t4853.*(t1896-t3239).*7.26735e-3+t2363.*(t684+t685-t710+t724+t1686-t1690+t1700+t1701+t2371+t2698+t2707-t2716+t2719+t3329-t3337-t3351-t3641+t3643+t3655-t3659+t4114+t4115).*7.26735e-3;
et215 = (t4843+t5108+t2307.*(t642+t643-t667+t674+t1587+t1606+t1608+t1609+t2295+t2671+t2683+t2684-t2695+t3279+t3297-t3303+t3597+t3603+t3609-t3614+t4053+t4054)+t2297.*(t2292+t3290+t3524.*1.838876e-2-t3591+t3592+t3611+t16.*(t1861-t3221).*3.131399999999998e-4+t16.*t17.*(t1861-t3221).*9.99471e-3))./2.0;
t7500 = et214.*et215;
et216 = t2363.*(t2368+t3340+t3582.*1.838876e-2-t3639+t3640+t21.*(t1896-t3239).*1.247162e-2+t27.*(t1896-t3239).*3.131399999999998e-4+t27.*t28.*(t1896-t3239).*9.99471e-3);
et217 = 7.26735e-3;
t7513 = ((t4814.*(t1861-t3221)+t2297.*(t642+t643-t667+t674+t1587+t1606+t1608+t1609+t2295+t2671+t2683+t2684-t2695+t3279+t3297-t3303+t3597+t3603+t3609-t3614+t4053+t4054)).*(t4925+t5194+et216.*et217+t2388.*(t684+t685-t710+t724+t1686-t1690+t1700+t1701+t2371+t2698+t2707-t2716+t2719+t3329-t3337-t3351-t3641+t3643+t3655-t3659+t4114+t4115).*7.26735e-3))./2.0;
t7522 = t3140+t3141+t3336+t3345+t3455+t3469+t4654+t4656+t4657+t4660+t4937+t4938+t4943+t4949+t5171+t5176+t5178+t5181;
t7640 = -t3055.*(-t5202+t5286+t5297+t5331-t5332-t5336+t5341+(t4920.*(t1861-t3221))./1.0e+8+(t3934.*(t951+t10.*(-t1881+t3121+t3276)))./1.0e+8+(t4118.*(t2694-t2701+t3036-t3043))./1.0e+8+t4835.*(t2694-t2701+t3036-t3043).*4.0e-8+t4838.*(t2694-t2701+t3036-t3043).*2.4e-7);
t7641 = t3055.*(-t5202+t5286+t5297+t5331-t5332-t5336+t5341+(t4920.*(t1861-t3221))./1.0e+8+(t3934.*(t951+t10.*(-t1881+t3121+t3276)))./1.0e+8+(t4118.*(t2694-t2701+t3036-t3043))./1.0e+8+t4835.*(t2694-t2701+t3036-t3043).*4.0e-8+t4838.*(t2694-t2701+t3036-t3043).*2.4e-7);
t7658 = (t3242-t3554).*(-t5202+t5286+t5297+t5331-t5332-t5336+t5341+(t4920.*(t1861-t3221))./1.0e+8+(t3934.*(t951+t10.*(-t1881+t3121+t3276)))./1.0e+8+(t4118.*(t2694-t2701+t3036-t3043))./1.0e+8+t4835.*(t2694-t2701+t3036-t3043).*4.0e-8+t4838.*(t2694-t2701+t3036-t3043).*2.4e-7);
t7659 = -t4026.*(-t5202+t5286+t5297+t5331-t5332-t5336+t5341+(t4920.*(t1861-t3221))./1.0e+8+(t3934.*(t951+t10.*(-t1881+t3121+t3276)))./1.0e+8+(t4118.*(t2694-t2701+t3036-t3043))./1.0e+8+t4835.*(t2694-t2701+t3036-t3043).*4.0e-8+t4838.*(t2694-t2701+t3036-t3043).*2.4e-7);
et218 = t5080-t7199+t4853.*(t1005+t20.*(t1941-t3315+t39.*t1022.*(t855-t878).*2.196325630278387e-1)).*7.26735e-3;
et219 = t2419.*(t684+t685-t710+t724+t1686-t1690+t1700+t1701+t2371+t2698+t2707-t2716+t2719+t3329-t3337-t3351-t3641+t3643+t3655-t3659+t4114+t4115).*7.26735e-3;
t7692 = ((et218+et219).*(t4814.*(t1861-t3221)+t2297.*(t642+t643-t667+t674+t1587+t1606+t1608+t1609+t2295+t2671+t2683+t2684-t2695+t3279+t3297-t3303+t3597+t3603+t3609-t3614+t4053+t4054)))./2.0;
t7733 = t5101+t5727+t5750+t6123+t7094+t7097;
t7785 = t5426+t5866+t5887+t6221+t7136+t7153;
t7789 = (t3217.*t7784)./2.0;
t7828 = t5657+t6127+t6158+t6661+t7332+t7333;
t4080 = -t4072;
t4081 = -t4073;
t4082 = -t4074;
t4134 = -t4127;
t4135 = -t4128;
t4136 = -t4129;
t4191 = -t4185;
t4700 = -t4699;
t4702 = -t4701;
t4860 = t3237.*t4556.*9.3e-7;
t4861 = t3237.*t4556.*1.02e-6;
t4864 = t3237.*t4556.*9.0e-8;
t4961 = -t4960;
t4963 = -t4962;
t4984 = t3547.*t4556.*9.3e-7;
t4985 = t3547.*t4556.*1.02e-6;
t4986 = t3550.*t4556.*9.3e-7;
t4987 = t3547.*t4556.*9.0e-8;
t4991 = t3550.*t4556.*9.0e-8;
t4996 = t21.*t4989;
t4999 = t21.*t4994;
t5031 = t3759.*t4604;
t5056 = t3873.*t4604;
t5128 = t3934.*t4556.*9.3e-7;
t5129 = t3934.*t4556.*1.02e-6;
t5130 = t3937.*t4556.*9.3e-7;
t5131 = t3934.*t4556.*9.0e-8;
t5134 = t3937.*t4556.*9.0e-8;
t5151 = t3977.*t4604;
t5182 = t4026.*t4556.*9.3e-7;
t5183 = t4026.*t4556.*1.02e-6;
t5184 = t4026.*t4556.*9.0e-8;
t5186 = t4031.*t4556.*9.3e-7;
t5190 = t4031.*t4556.*9.0e-8;
t5220 = t4151.*t4556.*9.3e-7;
t5221 = t4151.*t4556.*9.0e-8;
t5231 = t4160.*t4604;
t5232 = -t4604.*(-t2804+t2838+t3109+t17.*(t1456-t2355).*9.3e-7);
t5233 = -t4604.*(t2813-t2835+t12.*(t1456-t2355).*1.02e-6+t17.*(t1456-t2355).*9.0e-8);
t5238 = -t5235;
t5365 = -t5364;
t5367 = -t5366;
t5380 = -t5379;
t5427 = t2363.*t5382;
t5455 = t5453./2.0;
t5468 = t5467./2.0;
t5475 = t4556.*t4872.*9.3e-7;
t5476 = t4556.*t4872.*9.0e-8;
t5490 = t3055.*t5406;
t5515 = t4556.*t4915.*9.3e-7;
t5518 = t4556.*t4915.*9.0e-8;
t5546 = t2363.*t5484;
t5551 = -t5382.*(t1896-t3239);
t5552 = t3547.*t5382;
t5559 = t4764+t4773;
t5571 = t4777+t4819;
t5580 = t3055.*t5534;
t5626 = t5622.*(-1.0./2.0);
t5628 = t5622./2.0;
t5641 = -t5640;
t5642 = t5640./2.0;
t5668 = -t5484.*(t1896-t3239);
t5669 = t3547.*t5484;
t5670 = t5484.*(t1896-t3239);
t5673 = t5672./2.0;
t5706 = t50.*t189.*t5667.*9.543032792050485e-17;
t5709 = -t5707;
t5711 = -t5406.*(t3242-t3554);
t5713 = t4026.*t5406;
t5716 = -t5714;
t5774 = -t5773;
t5796 = -t5534.*(t3242-t3554);
t5798 = t4026.*t5534;
t5799 = t5534.*(t3242-t3554);
t5817 = -t5816;
t5819 = t5816./2.0;
t5827 = t5826./2.0;
t5837 = -t5834;
t5856 = t67+t68+t89+t92+t2673+t2685+t2687+t2692+t3232+t3537+t3606+t3621+t4073+t4074;
t5869 = t3755.*t3934.*t5491.*5.43845e-3;
t5880 = (t3503.*t5809)./2.0;
t5881 = t3810.*t3934.*t5491.*5.43845e-3;
t5898 = -t5897;
t5906 = -t5905;
t5910 = t5491.*(t3421-t3731+t3737+t20.*t50.*t202.*(t46-t47).*8.687615694748404e-39).*(-1.0./2.0);
t5911 = t358+t359+t378+t382+t2945+t2950+t2955+t2957+t3364+t3684+t3735+t3741+t4183+t4186;
t5912 = (t5491.*(t3421-t3731+t3737+t20.*t50.*t202.*(t46-t47).*8.687615694748404e-39))./2.0;
t5935 = -t5934;
t5936 = t5809.*(-t1901+t3122+t3277).*(-1.0./2.0);
t5937 = (t5809.*(-t1901+t3122+t3277))./2.0;
t5947 = t4215.*t5491.*(t2694-t2701+t3036-t3043).*(-5.43845e-3);
t5948 = t4215.*t5491.*(t2694-t2701+t3036-t3043).*5.43845e-3;
t5956 = (t3712.*t3910.*t5647)./2.0;
t5976 = (t3808.*t3910.*t5647)./2.0;
t5982 = t5809.*(t951+t10.*(-t1881+t3121+t3276)).*(-1.0./2.0);
t5986 = t5984./2.0;
t5988 = t5985./2.0;
t5997 = -t5996;
t5999 = -t5998;
t6000 = (t5026.*t5491)./2.0;
t6007 = -t6006;
t6009 = (t4712.*t5647)./2.0;
t6027 = -t6026;
t6028 = t4172.*t5647.*(t2674-t2676+t3022-t3027).*(-1.0./2.0);
t6029 = (t4172.*t5647.*(t2674-t2676+t3022-t3027))./2.0;
t6038 = -t6036;
t6039 = t4739+t5700;
t6041 = t4737+t5703;
t6043 = -t6042;
t6045 = -t6044;
t6046 = (t4950.*t5647)./2.0;
t6055 = -t6053;
t6060 = t4743+t5746;
t6064 = t4826+t5740;
t6082 = t2363.*t6058;
t6083 = t2388.*t6058;
t6084 = t2419.*t6058;
t6099 = t3261+t3270+t4427+t4430+t4435+t4451;
t6100 = t3267+t3268+t4429+t4432+t4441+t4450;
t6107 = -t6105;
t6111 = t3055.*t6065;
et220 = -t2306-t2317+t3145+t3148+t35.*t941.*t948.*(t850-t874).*3.775747223193135e-1;
et221 = t36.*t941.*t948.*(t850-t874).*2.244797987218524e-1;
t6116 = t5809.*(et220+et221).*(-1.0./2.0);
et222 = -t2306-t2317+t3145+t3148+t35.*t941.*t948.*(t850-t874).*3.775747223193135e-1;
et223 = t36.*t941.*t948.*(t850-t874).*2.244797987218524e-1;
t6117 = (t5809.*(et222+et223))./2.0;
t6120 = t27.*t2363.*t6098;
t6135 = t3543.*t6058;
t6136 = -t6058.*(t1896-t3239);
t6137 = t3547.*t6058;
t6138 = t3550.*t6058;
t6140 = t2998.*t6098;
t6145 = t3055.*t6098;
t6146 = -t6098.*(t1477-t2502);
t6148 = t6098.*(t1477-t2502);
t6169 = t3951.*t5857.*(t2694-t2701+t3036-t3043).*(-3.633675e-3);
t6170 = t3951.*t5858.*(t2694-t2701+t3036-t3043).*(-3.633675e-3);
t6173 = -t6171;
t6175 = -t6174;
t6180 = (t5278.*t5647)./2.0;
t6184 = t4018.*t5857.*(t2694-t2701+t3036-t3043).*(-3.633675e-3);
t6185 = t4018.*t5857.*(t2694-t2701+t3036-t3043).*3.633675e-3;
t6186 = t4018.*t5858.*(t2694-t2701+t3036-t3043).*(-3.633675e-3);
t6187 = t4018.*t5858.*(t2694-t2701+t3036-t3043).*3.633675e-3;
t6191 = -t6190;
t6192 = t6190./2.0;
t6193 = t3396.*t6102;
t6196 = t2363.*t6159;
t6197 = t2388.*t6159;
t6199 = t2419.*t6159;
t6205 = t4187.*t5857.*(t2694-t2701+t3036-t3043).*(-3.633675e-3);
t6206 = t4187.*t5857.*(t2694-t2701+t3036-t3043).*3.633675e-3;
t6207 = t4187.*t5858.*(t2694-t2701+t3036-t3043).*(-3.633675e-3);
t6208 = t4187.*t5858.*(t2694-t2701+t3036-t3043).*3.633675e-3;
t6214 = -t27.*t6098.*(t1896-t3239);
t6215 = t27.*t3547.*t6098;
t6216 = t27.*t6098.*(t1896-t3239);
t6223 = t3503.*(t4359-t5236+t4604.*(-t2804+t2838+t3109+t17.*(t1456-t2355).*9.3e-7)).*(-1.0./2.0);
t6224 = t11.*t3502.*(t4359-t5236+t4604.*(-t2804+t2838+t3109+t17.*(t1456-t2355).*9.3e-7)).*(-1.0./2.0);
t6225 = (t3503.*(t4359-t5236+t4604.*(-t2804+t2838+t3109+t17.*(t1456-t2355).*9.3e-7)))./2.0;
t6226 = (t11.*t3502.*(t4359-t5236+t4604.*(-t2804+t2838+t3109+t17.*(t1456-t2355).*9.3e-7)))./2.0;
t6228 = t5810.*(t2694-t2701+t3036-t3043).*(t1513+t1879+t2598+t2820+t2834+t3117+t3118).*3.633675e-3;
t6235 = -t6234;
t6237 = (t5491.*t5540)./2.0;
t6242 = t656+t659+t660+t681+t1577+t1578+t1586+t1600+t2303+t2339+t2673+t2685+t2686+t2687+t3030+t3232+t3299+t3312+t3537+t3606+t3621+t4073+t4074;
t6243 = t3430+t3432+t4570+t4580+t4586+t4603;
t6244 = t3426+t3444+t4571+t4574+t4592+t4597;
t6246 = t3443+t3448+t4578+t4599+t4624+t4628;
t6250 = (t5838.*(t2674-t2676+t3022-t3027).*(t1488+t1874+t2519+t2740+t2747+t3096+t3097))./2.0;
t6251 = t4151.*t6058;
t6252 = -t6058.*(t1005+t20.*(t1941-t3315+t39.*t1022.*(t855-t878).*2.196325630278387e-1));
t6254 = t188.*t6236.*8.595599785252598e-1;
t6262 = -t6065.*(t3242-t3554);
t6263 = t4026.*t6065;
t6267 = t50.*t189.*t6236.*9.543032792050485e-17;
t6276 = t694+t736+t740+t741+t1615+t1616+t1660+t1717+t2403+t2493+t2704+t2708+t2709+t2720+t3045+t3252+t3347+t3363+t3589+t3652+t3662+t4128+t4129;
t6283 = t6282.*(-1.0./2.0);
t6284 = t6282./2.0;
t6285 = t3543.*t6159;
t6286 = -t6159.*(t1896-t3239);
t6287 = t3547.*t6159;
t6288 = t3550.*t6159;
t6290 = t3925.*t5946.*(t2674-t2676+t3022-t3027).*(-1.0./2.0);
t6292 = t3925.*t5949.*(t2674-t2676+t3022-t3027).*(-1.0./2.0);
t6294 = t201.*t6273.*6.246723209935546e-3;
t6303 = t3975.*t5946.*(t2674-t2676+t3022-t3027).*(-1.0./2.0);
t6304 = (t3975.*t5946.*(t2674-t2676+t3022-t3027))./2.0;
t6306 = t3975.*t5949.*(t2674-t2676+t3022-t3027).*(-1.0./2.0);
t6308 = (t3975.*t5949.*(t2674-t2676+t3022-t3027))./2.0;
t6310 = t50.*t202.*t6273.*6.935255936130809e-19;
t6311 = ((-t1901+t3122+t3277).*(t4359-t5236+t4604.*(-t2804+t2838+t3109+t17.*(t1456-t2355).*9.3e-7)))./2.0;
t6317 = t3934.*t5857.*(t1513+t1879+t2598+t2820+t2834+t3117+t3118).*(-3.633675e-3);
t6318 = (t5491.*t5594)./2.0;
t6325 = t4019.*t6098;
t6327 = -t6098.*(t3242-t3554);
t6329 = t4026.*t6098;
t6331 = t4031.*t6098;
t6335 = -t6245.*(t1477-t2502);
t6337 = t6245.*(t1477-t2502);
t6338 = t3055.*t6247;
t6339 = -t6336;
t6342 = t4146.*t5946.*(t2674-t2676+t3022-t3027).*(-1.0./2.0);
t6343 = t4001.*(t4359-t5236+t4604.*(-t2804+t2838+t3109+t17.*(t1456-t2355).*9.3e-7)).*(-1.0./2.0);
t6345 = (t4146.*t5946.*(t2674-t2676+t3022-t3027))./2.0;
t6347 = t4146.*t5949.*(t2674-t2676+t3022-t3027).*(-1.0./2.0);
t6348 = (t4146.*t5949.*(t2674-t2676+t3022-t3027))./2.0;
t6356 = (t5465.*t5647)./2.0;
t6360 = t3055.*t6260;
t6367 = ((t951+t10.*(-t1881+t3121+t3276)).*(t4359-t5236+t4604.*(-t2804+t2838+t3109+t17.*(t1456-t2355).*9.3e-7)))./2.0;
t6369 = -t3395.*(t3428-t3432-t4570+t4576+t4582-t4603);
t6370 = t3395.*(t3428-t3432-t4570+t4576+t4582-t4603).*(-1.0./2.0);
t6380 = t6379.*(-1.0./2.0);
t6384 = t4779+t4783+t4791+t4829;
t6385 = t4776+t4787+t4811+t4817;
t6387 = t4778+t4795+t4801+t4827;
t6404 = -t6402;
t6406 = t3889+t4686+t4688+t4690+t4738;
t6413 = t4151.*t6159;
t6414 = -t6159.*(t1005+t20.*(t1941-t3315+t39.*t1022.*(t855-t878).*2.196325630278387e-1));
t6418 = t6417.*(-1.0./2.0);
t6419 = t6417./2.0;
t6420 = t3910.*t5946.*(t1488+t1874+t2519+t2740+t2747+t3096+t3097).*(-1.0./2.0);
t6430 = -t6428;
t6439 = t4573.*t6102;
t6443 = t4604.*t6101;
t6444 = -t6102.*(t3563-t4051);
et224 = t3582.*1.33637554986e-4+t3716-t3717+t27.*(t1896-t3239).*4.36041e-5;
et225 = t27.*t28.*(t1896-t3239).*7.26350557185e-5;
t6445 = t5857.*(et224+et225).*(-1.0./2.0);
et226 = t3582.*1.33637554986e-4+t3716-t3717+t27.*(t1896-t3239).*4.36041e-5;
et227 = t27.*t28.*(t1896-t3239).*7.26350557185e-5;
t6446 = (t5857.*(et226+et227))./2.0;
et228 = t3582.*1.33637554986e-4+t3716-t3717+t27.*(t1896-t3239).*4.36041e-5;
et229 = t27.*t28.*(t1896-t3239).*7.26350557185e-5;
t6447 = t5858.*(et228+et229).*(-1.0./2.0);
t6454 = t5857.*(t3359-t3670+t22.*(t3242-t3554).*1.33637554986e-4+t28.*(t3242-t3554).*7.26350557185e-5).*(-1.0./2.0);
t6455 = (t5857.*(t3359-t3670+t22.*(t3242-t3554).*1.33637554986e-4+t28.*(t3242-t3554).*7.26350557185e-5))./2.0;
t6456 = t5858.*(t3359-t3670+t22.*(t3242-t3554).*1.33637554986e-4+t28.*(t3242-t3554).*7.26350557185e-5).*(-1.0./2.0);
t6457 = (t5858.*(t3359-t3670+t22.*(t3242-t3554).*1.33637554986e-4+t28.*(t3242-t3554).*7.26350557185e-5))./2.0;
t6463 = -t6462;
t6464 = t3396.*t6390;
t6465 = t6462./2.0;
t6470 = t4019.*t6245;
t6475 = -t6247.*(t3242-t3554);
t6476 = t4031.*t6245;
t6478 = t4026.*t6247;
t6479 = -t6260.*(t3242-t3554);
t6480 = t4026.*t6260;
t6481 = t6260.*(t3242-t3554);
t6487 = -t6485;
t6495 = t5857.*(t3566.*1.33637554986e-4+t4157-t4158+t28.*(t1896-t3239).*7.26350557185e-5).*(-1.0./2.0);
t6496 = (t5857.*(t3566.*1.33637554986e-4+t4157-t4158+t28.*(t1896-t3239).*7.26350557185e-5))./2.0;
t6497 = t5858.*(t3566.*1.33637554986e-4+t4157-t4158+t28.*(t1896-t3239).*7.26350557185e-5).*(-1.0./2.0);
t6498 = (t5858.*(t3566.*1.33637554986e-4+t4157-t4158+t28.*(t1896-t3239).*7.26350557185e-5))./2.0;
t6501 = t5946.*(t3524.*1.838876e-2-t3591+t3592+t16.*(t1861-t3221).*(3.0./5.0e+2)+t16.*t17.*(t1861-t3221).*9.99471e-3).*(-1.0./2.0);
t6502 = (t5946.*(t3524.*1.838876e-2-t3591+t3592+t16.*(t1861-t3221).*(3.0./5.0e+2)+t16.*t17.*(t1861-t3221).*9.99471e-3))./2.0;
t6503 = t5949.*(t3524.*1.838876e-2-t3591+t3592+t16.*(t1861-t3221).*(3.0./5.0e+2)+t16.*t17.*(t1861-t3221).*9.99471e-3).*(-1.0./2.0);
t6509 = ((t11.*((t237.*(t42-t43))./9.007199254740992e+15+t15.*(-t1881+t3121+t3276))+t16.*(-t1901+t3122+t3277)).*(t4359-t5236+t4604.*(-t2804+t2838+t3109+t17.*(t1456-t2355).*9.3e-7)))./2.0;
t6510 = t4874.*t6098;
t6511 = t4880.*t6098;
t6514 = (t5647.*t5783)./2.0;
et230 = -t2306-t2317+t3145+t3148+t35.*t941.*t948.*(t850-t874).*3.775747223193135e-1;
et231 = t36.*t941.*t948.*(t850-t874).*2.244797987218524e-1;
t6518 = ((et230+et231).*(t4359-t5236+t4604.*(-t2804+t2838+t3109+t17.*(t1456-t2355).*9.3e-7)))./2.0;
t6519 = (t5313.*t5946)./2.0;
t6520 = (t5313.*t5949)./2.0;
t6541 = t5946.*(-t4045+t4049+t12.*(t1861-t3221).*1.838876e-2+t17.*(t1861-t3221).*9.99471e-3).*(-1.0./2.0);
t6542 = (t5946.*(-t4045+t4049+t12.*(t1861-t3221).*1.838876e-2+t17.*(t1861-t3221).*9.99471e-3))./2.0;
t6543 = t5949.*(-t4045+t4049+t12.*(t1861-t3221).*1.838876e-2+t17.*(t1861-t3221).*9.99471e-3).*(-1.0./2.0);
t6544 = (t5949.*(-t4045+t4049+t12.*(t1861-t3221).*1.838876e-2+t17.*(t1861-t3221).*9.99471e-3))./2.0;
t6547 = -t4577.*(t3428-t3432-t4570+t4576+t4582-t4603);
t6550 = -t4604.*(t3428-t3432-t4570+t4576+t4582-t4603);
t6561 = -t4604.*(t4618+t4634-t12.*t2363.*t3047.*9.0e-8-t17.*t2363.*t3047.*9.3e-7+t12.*t3980.*(t1896-t3239).*9.0e-8+t17.*t3980.*(t1896-t3239).*9.3e-7);
t6566 = t21.*t2363.*t6549;
t6571 = (t5491.*t5902)./2.0;
t6573 = t3003.*t6549;
t6578 = t3055.*t6549;
t6579 = -t6549.*(t1477-t2502);
t6580 = t6549.*(t1477-t2502).*(-1.0./2.0);
t6582 = (t6549.*(t1477-t2502))./2.0;
t6590 = t3701+t3702+t4875+t4881+t4909+t4910;
t6593 = t4573.*t6390;
t6598 = -t6596;
t6599 = t4604.*t6388;
t6600 = -t6390.*(t3563-t4051);
t6604 = -t21.*t6549.*(t1896-t3239);
t6605 = t21.*t3547.*t6549;
t6608 = -t6607;
t6645 = (t5790.*t5857)./2.0;
t6646 = (t5790.*t5858)./2.0;
t6657 = (t5491.*t6048)./2.0;
t6663 = t3055.*t6615;
t6665 = t4019.*t6549;
t6666 = -t6549.*(t3242-t3554);
t6667 = t4026.*t6549;
t6668 = t6549.*(t3242-t3554);
t6669 = t4031.*t6549;
t6679 = t5647.*(t1554+t2361+t2362+t2367+t2414+t3961+t3968+t4198+t4201+t11.*(-t1901+t3122+t3277).*5.68686e-3).*(-1.0./2.0);
t6681 = t3130+t3439+t3461+t4278+t4280+t4588+t4598+t4622+t4638;
t6690 = (t5647.*t6011)./2.0;
t6692 = (t5838.*t5857)./2.0;
t6693 = (t5838.*t5858)./2.0;
t6710 = t5111+t6350;
t6731 = t5857.*(t4673+t2363.*(t3566.*1.838876e-2+t4109-t4110+t28.*(t1896-t3239).*9.99471e-3).*7.26735e-3).*(-1.0./2.0);
t6732 = t5858.*(t4673+t2363.*(t3566.*1.838876e-2+t4109-t4110+t28.*(t1896-t3239).*9.99471e-3).*7.26735e-3).*(-1.0./2.0);
t6788 = (t5810.*t5946)./2.0;
t6789 = (t5810.*t5949)./2.0;
t6790 = t5195+t6382;
t6808 = t6804./2.0;
t6810 = -t6615.*(t3242-t3554);
t6811 = t4026.*t6615;
t6830 = t5946.*(t5413+t4146.*(t1861-t3221)).*(-1.0./2.0);
t6831 = (t5946.*(t5413+t4146.*(t1861-t3221)))./2.0;
t6832 = t5949.*(t5413+t4146.*(t1861-t3221)).*(-1.0./2.0);
t6833 = (t5949.*(t5413+t4146.*(t1861-t3221)))./2.0;
t6856 = t4494+t4495+t4779+t4785+t4810+t4829;
t6860 = t4872.*t6549;
t6861 = -t6549.*(t4165+t27.*(t1959-t3313+t38.*t1022.*(t855-t878).*2.196325630278387e-1));
t6869 = (t5491.*t6255)./2.0;
t6877 = (t3216.*t6809)./2.0;
t6894 = t6809.*(t1861-t3221).*(-1.0./2.0);
t6895 = (t6809.*(t1861-t3221))./2.0;
t6903 = t6902./2.0;
t6918 = t188.*t6914.*4.297799892626299e-1;
t6923 = t6809.*(t2674-t2676+t3022-t3027).*(-1.0./2.0);
t6924 = (t6809.*(t2674-t2676+t3022-t3027))./2.0;
t6941 = (t3980.*t6809)./2.0;
t6962 = (t3216.*t6913)./2.0;
t6963 = t4207+t4643+t4662+t4720+t5241+t5261;
t6968 = (t3216.*t6916)./2.0;
t6977 = t6913.*(t1861-t3221).*(-1.0./2.0);
t6981 = -t6979;
t6994 = t6916.*(t1861-t3221).*(-1.0./2.0);
t7011 = -t7010;
t7019 = -t7018;
t7028 = t6913.*(t2674-t2676+t3022-t3027).*(-1.0./2.0);
t7029 = (t6913.*(t2674-t2676+t3022-t3027))./2.0;
t7041 = (t3980.*t6913)./2.0;
t7042 = t6916.*(t2674-t2676+t3022-t3027).*(-1.0./2.0);
t7043 = (t6916.*(t2674-t2676+t3022-t3027))./2.0;
t7057 = (t3980.*t6916)./2.0;
t7081 = -t7080;
t7126 = -t7092.*(t1477-t2502);
t7127 = t7092.*(t1477-t2502).*(-1.0./2.0);
t7163 = -t7162;
t7168 = -t7166;
t7171 = -t7170;
t7195 = t3055.*t7155;
t7198 = -t7197;
t7203 = -t7201;
t7205 = -t7204;
t7208 = t4019.*t7092;
t7210 = t4031.*t7092;
t7211 = -t7155.*(t3242-t3554);
t7212 = t4026.*t7155;
t7213 = t7155.*(t3242-t3554);
t7223 = (t5857.*t6651)./2.0;
t7225 = (t5858.*t6651)./2.0;
t7232 = (t5946.*(-t2308+t2378+t2510-t2530-t2975+t2979+t3926+t4144+t4190+t4193+t4863+t4867))./2.0;
t7233 = (t5949.*(-t2308+t2378+t2510-t2530-t2975+t2979+t3926+t4144+t4190+t4193+t4863+t4867))./2.0;
t7246 = t5838.*(t4814.*(t1861-t3221)+t2297.*(t642+t643-t667+t674+t1587+t1606+t1608+t1609+t2295+t2671+t2683+t2684-t2695+t3279+t3297-t3303+t3597+t3603+t3609-t3614+t4053+t4054)).*(-1.0./2.0);
t7252 = t5810.*(t4853.*(t1896-t3239).*7.26735e-3+t2363.*(t684+t685-t710+t724+t1686-t1690+t1700+t1701+t2371+t2698+t2707-t2716+t2719+t3329-t3337-t3351-t3641+t3643+t3655-t3659+t4114+t4115).*7.26735e-3).*(-1.0./2.0);
t7253 = (t5810.*(t4853.*(t1896-t3239).*7.26735e-3+t2363.*(t684+t685-t710+t724+t1686-t1690+t1700+t1701+t2371+t2698+t2707-t2716+t2719+t3329-t3337-t3351-t3641+t3643+t3655-t3659+t4114+t4115).*7.26735e-3))./2.0;
t7278 = t2363.*t7277;
t7284 = t4845+t5114+t5719+t6351;
t7286 = -t7277.*(t1896-t3239);
t7287 = t3547.*t7277;
t7288 = t4926+t5196+t5757+t6383;
t7290 = t4344+t5053+t5149+t5150+t5660+t5662;
t7298 = t7297./2.0;
t7301 = -t7300;
t7313 = t3135+t3136+t3165+t3173+t3451+t3460+t4276+t4277+t4281+t4282+t4301+t4307+t4308+t4312+t4583+t4594+t4631+t4642;
t7339 = -t7337;
t7365 = -t7364;
t7375 = -t7374.*(t1477-t2502);
t7376 = t7374.*(t1477-t2502);
t7387 = t4019.*t7374;
t7388 = t4031.*t7374;
t7404 = t7379.*(t2674-t2676+t3022-t3027).*(-1.0./2.0);
t7405 = (t7379.*(t2674-t2676+t3022-t3027))./2.0;
t7406 = (t3910.*t7380)./2.0;
et232 = t2363.*(t2368+t3340+t3582.*1.838876e-2-t3639+t3640+t21.*(t1896-t3239).*1.247162e-2+t27.*(t1896-t3239).*3.131399999999998e-4+t27.*t28.*(t1896-t3239).*9.99471e-3);
et233 = 7.26735e-3;
t7410 = t5857.*(t4925+t5194+et232.*et233+t2388.*(t684+t685-t710+t724+t1686-t1690+t1700+t1701+t2371+t2698+t2707-t2716+t2719+t3329-t3337-t3351-t3641+t3643+t3655-t3659+t4114+t4115).*7.26735e-3).*(-1.0./2.0);
et234 = t2363.*(t2368+t3340+t3582.*1.838876e-2-t3639+t3640+t21.*(t1896-t3239).*1.247162e-2+t27.*(t1896-t3239).*3.131399999999998e-4+t27.*t28.*(t1896-t3239).*9.99471e-3);
et235 = 7.26735e-3;
t7411 = (t5857.*(t4925+t5194+et234.*et235+t2388.*(t684+t685-t710+t724+t1686-t1690+t1700+t1701+t2371+t2698+t2707-t2716+t2719+t3329-t3337-t3351-t3641+t3643+t3655-t3659+t4114+t4115).*7.26735e-3))./2.0;
et236 = t2363.*(t2368+t3340+t3582.*1.838876e-2-t3639+t3640+t21.*(t1896-t3239).*1.247162e-2+t27.*(t1896-t3239).*3.131399999999998e-4+t27.*t28.*(t1896-t3239).*9.99471e-3);
et237 = 7.26735e-3;
t7412 = t5858.*(t4925+t5194+et236.*et237+t2388.*(t684+t685-t710+t724+t1686-t1690+t1700+t1701+t2371+t2698+t2707-t2716+t2719+t3329-t3337-t3351-t3641+t3643+t3655-t3659+t4114+t4115).*7.26735e-3).*(-1.0./2.0);
et238 = t2363.*(t2368+t3340+t3582.*1.838876e-2-t3639+t3640+t21.*(t1896-t3239).*1.247162e-2+t27.*(t1896-t3239).*3.131399999999998e-4+t27.*t28.*(t1896-t3239).*9.99471e-3);
et239 = 7.26735e-3;
t7413 = (t5858.*(t4925+t5194+et238.*et239+t2388.*(t684+t685-t710+t724+t1686-t1690+t1700+t1701+t2371+t2698+t2707-t2716+t2719+t3329-t3337-t3351-t3641+t3643+t3655-t3659+t4114+t4115).*7.26735e-3))./2.0;
t7416 = t5946.*(t4843+t5108+t2307.*(t642+t643-t667+t674+t1587+t1606+t1608+t1609+t2295+t2671+t2683+t2684-t2695+t3279+t3297-t3303+t3597+t3603+t3609-t3614+t4053+t4054)+t2297.*(t2292+t3290+t3524.*1.838876e-2-t3591+t3592+t3611+t16.*(t1861-t3221).*3.131399999999998e-4+t16.*t17.*(t1861-t3221).*9.99471e-3)).*(-1.0./2.0);
t7417 = t5949.*(t4843+t5108+t2307.*(t642+t643-t667+t674+t1587+t1606+t1608+t1609+t2295+t2671+t2683+t2684-t2695+t3279+t3297-t3303+t3597+t3603+t3609-t3614+t4053+t4054)+t2297.*(t2292+t3290+t3524.*1.838876e-2-t3591+t3592+t3611+t16.*(t1861-t3221).*3.131399999999998e-4+t16.*t17.*(t1861-t3221).*9.99471e-3)).*(-1.0./2.0);
t7434 = t5284+t5292+t5295+t5298+t5328+t5338+t5339+t5340;
t7436 = t7435./2.0;
t7468 = t2993+t3054+t3187+t3192+t3199+t3202+t4465+t4467+t4496+t4497+t4790+t4796+t4813+t4832+t5072+t5074+t5076+t5079;
t7479 = t5047+t5310+t6353+t7158;
t7501 = -t7500;
t7504 = t5081+t5357+t6386+t7199;
t7514 = -t7513;
t7531 = t3055.*t7522;
t7553 = -t7522.*(t3242-t3554);
t7554 = t4026.*t7522;
t7555 = t7522.*(t3242-t3554);
t7560 = t3500.*(t6979+t4019.*(t4795+t4801+t4808+t3976.*(t2694-t2701+t3036-t3043).*5.7e-7)+t6159.*(t1896-t3239)).*(-1.0./2.0);
t7561 = (t3500.*(t6979+t4019.*(t4795+t4801+t4808+t3976.*(t2694-t2701+t3036-t3043).*5.7e-7)+t6159.*(t1896-t3239)))./2.0;
et240 = t5080-t7199+t4853.*(t1005+t20.*(t1941-t3315+t39.*t1022.*(t855-t878).*2.196325630278387e-1)).*7.26735e-3;
et241 = t2419.*(t684+t685-t710+t724+t1686-t1690+t1700+t1701+t2371+t2698+t2707-t2716+t2719+t3329-t3337-t3351-t3641+t3643+t3655-t3659+t4114+t4115).*7.26735e-3;
t7624 = t5857.*(et240+et241).*(-1.0./2.0);
et242 = t5080-t7199+t4853.*(t1005+t20.*(t1941-t3315+t39.*t1022.*(t855-t878).*2.196325630278387e-1)).*7.26735e-3;
et243 = t2419.*(t684+t685-t710+t724+t1686-t1690+t1700+t1701+t2371+t2698+t2707-t2716+t2719+t3329-t3337-t3351-t3641+t3643+t3655-t3659+t4114+t4115).*7.26735e-3;
t7626 = t5858.*(et242+et243).*(-1.0./2.0);
t7637 = t4848+t4849+t5202+t5203+t5289+t5290+t5294+t5300+t5332+t5335+t5336+t5342;
t7642 = t7641.*(-1.0./2.0);
t7737 = t50.*t189.*t7733.*4.771516396025243e-17;
t4862 = -t4861;
t4868 = -t4864;
t4990 = t21.*t4984;
t4995 = t21.*t4987;
t5377 = t3607+t3608+t4075+t4080;
t5398 = t3653+t3654+t4124+t4134;
tau_c = ft_14({dq1,dq2,dq3,dq4,dq5,dq6,t10,t1005,t1022,t1089,t11,t1104,t1105,t1108,t1115,t1121,t1158,t1159,t1196,t12,t1205,t1210,t1212,t1217,t1218,t123,t1237,t1238,t1288,t1289,t13,t1302,t1303,t1319,t1320,t1336,t1348,t1350,t1351,t1360,t1369,t1378,t1396,t14,t140,t1425,t1435,t1456,t1477,t1488,t15,t1513,t1539,t1554,t1577,t1578,t1586,t1587,t16,t1600,t1604,t1605,t1606,t1607,t1608,t1609,t1628,t1629,t1637,t1640,t1641,t1659,t1661,t1666,t1667,t1683,t1686,t1690,t1692,t17,t1700,t1701,t1705,t1712,t1741,t1742,t1750,t1754,t1758,t1759,t1775,t1776,t18,t1861,t1874,t1879,t188,t1881,t189,t1896,t19,t1901,t1941,t1959,t1973,t1993,t1994,t20,t201,t202,t2023,t2053,t2060,t2089,t2090,t2098,t2099,t21,t2117,t2120,t2122,t2123,t2139,t2140,t2147,t2152,t2154,t2155,t2159,t2165,t2174,t2183,t2187,t2193,t2194,t2195,t2199,t22,t2203,t2215,t2219,t2222,t2223,t2239,t2240,t2256,t2257,t2292,t2295,t2297,t2302,t2303,t2306,t2307,t2308,t2317,t2337,t2338,t2339,t2355,t236,t2361,t2362,t2363,t2367,t2368,t237,t2371,t2378,t238,t2388,t2399,t24,t2401,t241,t2414,t2419,t25,t2502,t2510,t2519,t2527,t2530,t2555,t2556,t2572,t2583,t2598,t26,t2605,t2606,t2612,t2613,t2618,t2619,t262,t264,t2651,t2652,t2670,t2671,t2674,t2676,t2680,t2683,t2684,t2689,t2693,t2694,t2695,t2697,t2698,t27,t2700,t2701,t2707,t2712,t2715,t2716,t2719,t2721,t2740,t2747,t2748,t2749,t2754,t2773,t2781,t2788,t28,t2801,t2804,t2813,t2814,t2820,t2831,t2834,t2835,t2838,t2850,t2851,t29,t2953,t2965,t2966,t2975,t2979,t2990,t2991,t2994,t30,t3003,t3009,t3015,t3022,t3027,t3030,t3036,t3043,t3047,t3055,t3057,t3058,t3064,t3068,t3072,t3080,t3096,t3097,t31,t3109,t3117,t3118,t3121,t3122,t3126,t3129,t313,t3131,t3132,t3133,t314,t3142,t3143,t3145,t3148,t3157,t3158,t3171,t3193,t3194,t3195,t32,t3200,t3201,t3205,t3208,t3209,t321,t3211,t3213,t3216,t3217,t3221,t3235,t3236,t3237,t3238,t3239,t3242,t3257,t3276,t3277,t3279,t3283,t329,t3290,t3297,t3298,t3299,t33,t3303,t3312,t3313,t3314,t3315,t3318,t332,t3322,t3324,t3328,t3329,t3334,t3337,t3340,t3344,t3346,t335,t3351,t3359,t3367,t3369,t3370,t3386,t3395,t3396,t34,t3405,t3409,t3415,t3416,t3420,t3423,t3428,t3431,t3432,t3434,t3435,t3446,t3448,t346,t3463,t3468,t3471,t3474,t3480,t3482,t3483,t3488,t3489,t3490,t3492,t3495,t3496,t3498,t3499,t35,t350,t3500,t3502,t3503,t3512,t3517,t3524,t354,t3541,t3543,t3545,t3546,t3547,t3549,t3551,t3552,t3554,t3558,t3561,t3563,t3566,t3582,t3588,t3590,t3591,t3592,t3597,t36,t3603,t3609,t3610,t3611,t3614,t3617,t3624,t3637,t3638,t3639,t3640,t3641,t3642,t3643,t3649,t3655,t3656,t3658,t3659,t366,t3660,t3664,t3670,t3678,t3688,t3689,t3690,t3692,t3693,t3695,t3696,t3697,t3699,t3703,t3704,t3705,t3706,t3707,t3708,t3709,t3710,t3712,t3713,t3716,t3717,t3728,t3729,t3732,t3736,t3738,t3739,t3746,t3747,t3752,t3755,t3765,t3766,t3770,t3771,t3772,t3774,t3775,t3777,t3779,t3781,t3782,t3783,t3784,t3785,t3786,t3788,t3789,t3790,t3791,t3792,t3793,t3794,t3795,t3796,t3797,t3798,t38,t3800,t3801,t3802,t3804,t3805,t3808,t3809,t3810,t3817,t3818,t3820,t3821,t3823,t3824,t3826,t3827,t3828,t3830,t3832,t3833,t3835,t3840,t3843,t3844,t3845,t3846,t3848,t3850,t3851,t3855,t3856,t3857,t3862,t3863,t387,t3876,t3877,t3878,t3879,t3880,t3890,t3891,t3893,t3895,t3896,t3897,t3898,t39,t3901,t3902,t3903,t3906,t3908,t3910,t3913,t3915,t3924,t3925,t3926,t3931,t3934,t3937,t3943,t3951,t3961,t3967,t3968,t3974,t3975,t3976,t3980,t3985,t3991,t3993,t4001,t4006,t4008,t4018,t4019,t4026,t4030,t4031,t4032,t4035,t4039,t4041,t4045,t4047,t4049,t4051,t4053,t4054,t4065,t4081,t4082,t410,t4100,t4109,t4110,t4114,t4115,t4118,t4135,t4136,t4144,t4146,t4147,t4151,t4153,t4154,t4157,t4158,t4163,t4165,t4171,t4172,t4184,t4187,t4190,t4191,t4193,t4198,t42,t4201,t4205,t4208,t4213,t4215,t4236,t4240,t4244,t4260,t4261,t4263,t4270,t4272,t4273,t4274,t4275,t4281,t4282,t4286,t4287,t4288,t4289,t4290,t4291,t4292,t4299,t43,t4300,t4301,t4303,t4308,t4310,t4313,t4314,t4318,t4321,t4324,t4325,t4326,t4330,t4332,t4334,t4337,t4339,t4341,t4342,t4343,t4345,t4346,t4352,t4356,t4358,t4359,t4361,t4364,t4368,t4371,t4372,t4373,t4375,t4406,t4413,t4415,t4416,t4417,t4458,t4459,t4461,t4464,t4468,t4470,t4476,t4486,t4488,t4489,t4493,t4494,t4495,t4501,t4502,t4504,t4515,t4518,t4520,t4522,t4537,t4545,t4553,t4559,t4562,t4563,t4567,t4570,t4573,t4576,t4577,t4582,t4583,t4594,t46,t4603,t4604,t4606,t4615,t4617,t4618,t4619,t4623,t4634,t4635,t4639,t4644,t4645,t4651,t4652,t4658,t4663,t4665,t4673,t4675,t4676,t4677,t4678,t4680,t4683,t4691,t4692,t4694,t4696,t4697,t4698,t47,t4700,t4702,t4703,t4704,t4705,t4708,t4709,t4713,t4716,t4719,t4722,t4724,t4725,t4727,t4728,t4730,t4741,t4744,t4746,t4751,t4757,t4760,t4761,t4762,t4763,t4795,t4799,t4801,t4808,t4809,t4814,t4823,t4828,t4833,t4835,t4838,t4843,t4844,t4846,t4847,t4850,t4851,t4852,t4853,t4854,t4856,t4857,t4858,t4859,t4860,t4862,t4863,t4864,t4865,t4866,t4867,t4868,t4870,t4872,t4874,t4876,t4879,t4880,t4887,t4888,t4889,t4893,t4895,t4896,t4898,t4901,t4902,t4903,t4904,t4905,t4906,t4907,t4908,t4911,t4912,t4913,t4914,t4915,t4920,t4923,t4924,t4925,t4927,t4928,t4935,t4936,t4950,t4952,t4953,t4955,t4957,t4958,t4959,t4961,t4963,t4965,t4967,t4969,t4970,t4971,t4972,t4973,t4974,t4976,t4977,t4978,t4979,t4981,t4982,t4983,t4984,t4985,t4986,t4987,t4989,t4990,t4991,t4992,t4993,t4994,t4995,t4996,t4997,t4998,t4999,t50,t5001,t5003,t5004,t5005,t5007,t5009,t5010,t5011,t5012,t5013,t5014,t5016,t5021,t5023,t5025,t5026,t5027,t5028,t5031,t5032,t5033,t5034,t5035,t5036,t5037,t5038,t5041,t5042,t5043,t5045,t5046,t5049,t5051,t5056,t5057,t5062,t5063,t5080,t5082,t5083,t5084,t5085,t5086,t5087,t5088,t5089,t5090,t5091,t5093,t5096,t5097,t5098,t5103,t5105,t5106,t5108,t5109,t5112,t5113,t5116,t5117,t5118,t5119,t5120,t5121,t5123,t5124,t5125,t5126,t5127,t5128,t5129,t5130,t5131,t5133,t5134,t5135,t5136,t5137,t5138,t5139,t5141,t5142,t5151,t5152,t5153,t5154,t5155,t5156,t5158,t5159,t5161,t5162,t5163,t5164,t5166,t5167,t5169,t5182,t5183,t5184,t5185,t5186,t5187,t5188,t5189,t5190,t5191,t5192,t5193,t5194,t5197,t5198,t5199,t5200,t5201,t5202,t5205,t5206,t5207,t5208,t5211,t5212,t5213,t5214,t5216,t5220,t5221,t5222,t5223,t5231,t5232,t5233,t5234,t5235,t5236,t5237,t5238,t5240,t5243,t5246,t5247,t5248,t5249,t5251,t5254,t5255,t5256,t5257,t5258,t5259,t5262,t5264,t5265,t5275,t5278,t5279,t5280,t5281,t5283,t5286,t5287,t5291,t5296,t5297,t5301,t5302,t5303,t5304,t5305,t5306,t5308,t5309,t5312,t5313,t5317,t5328,t5331,t5332,t5333,t5336,t5337,t5340,t5341,t5343,t5344,t5345,t5346,t5348,t5350,t5352,t5353,t5356,t5358,t5359,t5361,t5362,t5363,t5365,t5367,t5369,t5370,t5372,t5373,t5374,t5376,t5377,t5380,t5381,t5382,t5383,t5384,t5385,t5386,t5387,t5389,t5390,t5391,t5392,t5393,t5395,t5398,t5399,t5400,t5401,t5402,t5403,t5404,t5405,t5410,t5411,t5412,t5413,t5415,t5416,t5419,t5421,t5422,t5425,t5427,t5433,t5434,t5436,t5437,t5438,t5439,t5440,t5441,t5442,t5443,t5444,t5445,t5446,t5448,t5449,t5451,t5452,t5453,t5455,t5456,t5457,t5458,t5459,t5460,t5464,t5465,t5466,t5467,t5468,t5470,t5472,t5473,t5474,t5475,t5476,t5477,t5478,t5480,t5481,t5483,t5486,t5487,t5488,t5489,t5490,t5491,t5493,t5494,t5495,t5497,t5499,t5500,t5501,t5502,t5503,t5504,t5505,t5506,t5507,t5508,t5509,t5510,t5511,t5512,t5513,t5514,t5515,t5516,t5517,t5518,t5519,t5520,t5521,t5523,t5535,t5536,t5537,t5538,t5539,t5542,t5543,t5544,t5545,t5546,t5548,t5549,t5550,t5551,t5552,t5553,t5554,t5555,t5556,t5557,t5558,t5560,t5563,t5564,t5565,t5567,t5568,t5569,t5570,t5572,t5573,t5574,t5575,t5576,t5577,t5578,t5579,t5580,t5581,t5583,t5585,t5586,t5587,t5588,t5589,t5590,t5591,t5592,t5593,t5594,t5596,t5597,t5598,t5599,t56,t5600,t5601,t5602,t5603,t5604,t5605,t5606,t5607,t5608,t5609,t5611,t5612,t5613,t5614,t5615,t5616,t5618,t5619,t5622,t5623,t5624,t5625,t5626,t5628,t5629,t5630,t5631,t5632,t5633,t5634,t5635,t5636,t5637,t5638,t5641,t5642,t5645,t5646,t5647,t5649,t5650,t5651,t5652,t5653,t5655,t5658,t5659,t5661,t5663,t5669,t5670,t5672,t5673,t5675,t5677,t5678,t5679,t5680,t5681,t5682,t5683,t5684,t5685,t5686,t5687,t5688,t5689,t5690,t5691,t5694,t5695,t5698,t5699,t5706,t5709,t5710,t5711,t5712,t5713,t5714,t5716,t5717,t5718,t5720,t5721,t5722,t5723,t5724,t5725,t5730,t5731,t5734,t5735,t5738,t5739,t5741,t5742,t5745,t5747,t5751,t5753,t5754,t5756,t5758,t5759,t5760,t5761,t5762,t5763,t5764,t5765,t5766,t5768,t5769,t5770,t5772,t5773,t5774,t5775,t5776,t5777,t5778,t5779,t5781,t5782,t5783,t5784,t5787,t5788,t5790,t5792,t5793,t5794,t5795,t5796,t5798,t5799,t5801,t5802,t5804,t5809,t5810,t5813,t5814,t5816,t5817,t5819,t5821,t5825,t5826,t5827,t5828,t5829,t5831,t5832,t5833,t5835,t5836,t5837,t5838,t5839,t5840,t5842,t5844,t5845,t5846,t5849,t5851,t5852,t5853,t5855,t5856,t5857,t5858,t5863,t5864,t5867,t5868,t5869,t5871,t5872,t5874,t5875,t5876,t5877,t5878,t5879,t5880,t5881,t5884,t5886,t5888,t5890,t5891,t5892,t5893,t5894,t5896,t5897,t5898,t5899,t5900,t5901,t5902,t5904,t5905,t5906,t5907,t5908,t5909,t5910,t5911,t5912,t5913,t5914,t5915,t5916,t5917,t5918,t5919,t5920,t5922,t5923,t5924,t5925,t5926,t5927,t5928,t5930,t5931,t5933,t5934,t5935,t5937,t5938,t5939,t5941,t5942,t5943,t5945,t5946,t5947,t5948,t5949,t5950,t5951,t5954,t5955,t5956,t5959,t5960,t5963,t5965,t5966,t5967,t5968,t5971,t5973,t5974,t5975,t5976,t5978,t5979,t5980,t5981,t5982,t5983,t5984,t5985,t5986,t5988,t5990,t5992,t5993,t5997,t5999,t60,t6000,t6001,t6004,t6005,t6006,t6007,t6008,t6009,t6011,t6013,t6014,t6015,t6017,t6018,t6019,t6020,t6021,t6022,t6023,t6024,t6026,t6027,t6028,t6029,t6031,t6034,t6035,t6037,t6038,t6039,t6041,t6043,t6045,t6046,t6047,t6050,t6052,t6053,t6054,t6055,t6058,t6059,t6060,t6062,t6064,t6065,t6066,t6067,t6074,t6076,t6079,t6080,t6081,t6082,t6083,t6084,t6091,t6093,t6094,t6095,t6096,t6098,t6099,t6100,t6102,t6106,t6107,t6109,t6110,t6111,t6113,t6114,t6115,t6116,t6119,t6120,t6125,t6129,t6131,t6133,t6134,t6135,t6136,t6137,t6138,t6140,t6143,t6144,t6145,t6148,t6159,t6162,t6164,t6166,t6168,t6169,t6170,t6171,t6172,t6173,t6174,t6175,t6180,t6183,t6184,t6185,t6186,t6187,t6190,t6191,t6192,t6193,t6196,t6197,t6199,t6205,t6206,t6207,t6208,t6211,t6213,t6215,t6216,t6217,t6219,t6223,t6225,t6226,t6227,t6228,t6231,t6232,t6233,t6234,t6237,t6239,t6240,t6241,t6242,t6244,t6250,t6251,t6252,t6254,t6255,t6256,t6257,t6262,t6263,t6267,t6270,t6271,t6272,t6275,t6276,t6281,t6282,t6283,t6284,t6285,t6286,t6287,t6288,t6290,t6291,t6292,t6293,t6294,t6303,t6304,t6306,t6307,t6308,t6310,t6311,t6313,t6314,t6316,t6317,t6318,t6324,t6325,t6327,t6329,t6331,t6334,t6337,t6338,t6339,t6342,t6343,t6345,t6347,t6348,t6354,t6356,t6360,t6366,t6367,t6369,t6375,t6376,t6377,t6379,t6384,t6387,t6394,t6396,t6398,t640,t6402,t6404,t6405,t6406,t6407,t6408,t6411,t6412,t6413,t6414,t6417,t6418,t6419,t642,t6420,t6422,t6423,t6425,t6426,t6428,t643,t6430,t6431,t6432,t6438,t6439,t6440,t6441,t6442,t6443,t6444,t6445,t6446,t6447,t6455,t6457,t6460,t6461,t6462,t6463,t6464,t6465,t6470,t6471,t6473,t6474,t6475,t6476,t6477,t6478,t6480,t6481,t6482,t6483,t6484,t6487,t6488,t649,t6491,t6496,t6498,t6501,t6502,t6503,t6508,t6509,t6510,t6511,t6512,t6513,t6514,t6515,t6517,t6518,t6519,t6520,t6523,t6524,t6525,t6526,t6527,t6528,t6530,t6531,t6537,t6538,t6542,t6544,t6547,t6549,t6550,t6559,t6560,t6561,t6562,t6564,t6565,t6566,t6569,t6570,t6571,t6572,t6573,t6574,t6576,t6578,t6579,t6580,t6582,t6588,t6589,t6591,t6592,t6593,t6594,t6595,t6596,t6598,t6599,t6600,t6601,t6602,t6604,t6605,t6606,t6607,t6608,t6622,t6623,t6624,t6625,t6645,t6646,t6651,t6652,t6654,t6656,t6657,t6658,t6659,t6660,t6663,t6665,t6667,t6668,t6669,t667,t6671,t6672,t6673,t6678,t6679,t668,t6680,t6681,t6687,t6688,t669,t6690,t6692,t6693,t670,t6714,t6715,t6731,t6732,t674,t6745,t6747,t6750,t6751,t677,t6788,t6789,t6804,t6808,t6810,t6811,t682,t6831,t6833,t684,t685,t6858,t6859,t686,t6860,t6861,t6868,t6869,t687,t6877,t6881,t6882,t6883,t6894,t6896,t6897,t6901,t6902,t6903,t6905,t6906,t6913,t6916,t6918,t6919,t6920,t6921,t6922,t6923,t6924,t6941,t6962,t6963,t6965,t6966,t6968,t6974,t6976,t6978,t6979,t6980,t6981,t6984,t6987,t6994,t7003,t7005,t7007,t7010,t7011,t7014,t7016,t7019,t7020,t7021,t7028,t7029,t7035,t7041,t7042,t7043,t7054,t7055,t7057,t7059,t707,t708,t7080,t7083,t7086,t7088,t7092,t7095,t7098,t71,t710,t7100,t7101,t7120,t7123,t7126,t7127,t7134,t7137,t7138,t7148,t715,t7150,t7159,t716,t7160,t7162,t7164,t7166,t7168,t7169,t7170,t7171,t7195,t7197,t7199,t7203,t7204,t7205,t7208,t721,t7210,t7211,t7212,t7213,t722,t7223,t7225,t7232,t7233,t724,t7246,t725,t7253,t7256,t7260,t7277,t7278,t7281,t7283,t7286,t7287,t7292,t7294,t7297,t7298,t73,t7300,t7301,t7304,t7309,t7310,t7311,t7315,t7319,t7322,t7323,t7335,t7337,t7339,t7340,t7344,t7345,t7348,t7349,t7358,t7360,t7364,t7365,t7366,t7376,t7379,t7380,t7385,t7387,t7388,t7401,t7402,t7403,t7404,t7405,t7406,t7410,t7411,t7412,t7413,t7416,t7417,t7435,t7436,t7458,t7459,t7468,t7479,t749,t7501,t7514,t7531,t7553,t7554,t7555,t7560,t7561,t762,t7624,t7626,t7641,t7658,t7659,t768,t7692,t7737,t777,t7784,t7789,t7790,t7827,t7828,t792,t793,t8,t801,t802,t808,t813,t819,t821,t850,t855,t874,t878,t9,t941,t948,t951,t97});
end
function tau_c = ft_14(ct)
dq1 = ct{1};
dq2 = ct{2};
dq3 = ct{3};
dq4 = ct{4};
dq5 = ct{5};
dq6 = ct{6};
t10 = ct{7};
t1005 = ct{8};
t1022 = ct{9};
t1089 = ct{10};
t11 = ct{11};
t1104 = ct{12};
t1105 = ct{13};
t1108 = ct{14};
t1115 = ct{15};
t1121 = ct{16};
t1158 = ct{17};
t1159 = ct{18};
t1196 = ct{19};
t12 = ct{20};
t1205 = ct{21};
t1210 = ct{22};
t1212 = ct{23};
t1217 = ct{24};
t1218 = ct{25};
t123 = ct{26};
t1237 = ct{27};
t1238 = ct{28};
t1288 = ct{29};
t1289 = ct{30};
t13 = ct{31};
t1302 = ct{32};
t1303 = ct{33};
t1319 = ct{34};
t1320 = ct{35};
t1336 = ct{36};
t1348 = ct{37};
t1350 = ct{38};
t1351 = ct{39};
t1360 = ct{40};
t1369 = ct{41};
t1378 = ct{42};
t1396 = ct{43};
t14 = ct{44};
t140 = ct{45};
t1425 = ct{46};
t1435 = ct{47};
t1456 = ct{48};
t1477 = ct{49};
t1488 = ct{50};
t15 = ct{51};
t1513 = ct{52};
t1539 = ct{53};
t1554 = ct{54};
t1577 = ct{55};
t1578 = ct{56};
t1586 = ct{57};
t1587 = ct{58};
t16 = ct{59};
t1600 = ct{60};
t1604 = ct{61};
t1605 = ct{62};
t1606 = ct{63};
t1607 = ct{64};
t1608 = ct{65};
t1609 = ct{66};
t1628 = ct{67};
t1629 = ct{68};
t1637 = ct{69};
t1640 = ct{70};
t1641 = ct{71};
t1659 = ct{72};
t1661 = ct{73};
t1666 = ct{74};
t1667 = ct{75};
t1683 = ct{76};
t1686 = ct{77};
t1690 = ct{78};
t1692 = ct{79};
t17 = ct{80};
t1700 = ct{81};
t1701 = ct{82};
t1705 = ct{83};
t1712 = ct{84};
t1741 = ct{85};
t1742 = ct{86};
t1750 = ct{87};
t1754 = ct{88};
t1758 = ct{89};
t1759 = ct{90};
t1775 = ct{91};
t1776 = ct{92};
t18 = ct{93};
t1861 = ct{94};
t1874 = ct{95};
t1879 = ct{96};
t188 = ct{97};
t1881 = ct{98};
t189 = ct{99};
t1896 = ct{100};
t19 = ct{101};
t1901 = ct{102};
t1941 = ct{103};
t1959 = ct{104};
t1973 = ct{105};
t1993 = ct{106};
t1994 = ct{107};
t20 = ct{108};
t201 = ct{109};
t202 = ct{110};
t2023 = ct{111};
t2053 = ct{112};
t2060 = ct{113};
t2089 = ct{114};
t2090 = ct{115};
t2098 = ct{116};
t2099 = ct{117};
t21 = ct{118};
t2117 = ct{119};
t2120 = ct{120};
t2122 = ct{121};
t2123 = ct{122};
t2139 = ct{123};
t2140 = ct{124};
t2147 = ct{125};
t2152 = ct{126};
t2154 = ct{127};
t2155 = ct{128};
t2159 = ct{129};
t2165 = ct{130};
t2174 = ct{131};
t2183 = ct{132};
t2187 = ct{133};
t2193 = ct{134};
t2194 = ct{135};
t2195 = ct{136};
t2199 = ct{137};
t22 = ct{138};
t2203 = ct{139};
t2215 = ct{140};
t2219 = ct{141};
t2222 = ct{142};
t2223 = ct{143};
t2239 = ct{144};
t2240 = ct{145};
t2256 = ct{146};
t2257 = ct{147};
t2292 = ct{148};
t2295 = ct{149};
t2297 = ct{150};
t2302 = ct{151};
t2303 = ct{152};
t2306 = ct{153};
t2307 = ct{154};
t2308 = ct{155};
t2317 = ct{156};
t2337 = ct{157};
t2338 = ct{158};
t2339 = ct{159};
t2355 = ct{160};
t236 = ct{161};
t2361 = ct{162};
t2362 = ct{163};
t2363 = ct{164};
t2367 = ct{165};
t2368 = ct{166};
t237 = ct{167};
t2371 = ct{168};
t2378 = ct{169};
t238 = ct{170};
t2388 = ct{171};
t2399 = ct{172};
t24 = ct{173};
t2401 = ct{174};
t241 = ct{175};
t2414 = ct{176};
t2419 = ct{177};
t25 = ct{178};
t2502 = ct{179};
t2510 = ct{180};
t2519 = ct{181};
t2527 = ct{182};
t2530 = ct{183};
t2555 = ct{184};
t2556 = ct{185};
t2572 = ct{186};
t2583 = ct{187};
t2598 = ct{188};
t26 = ct{189};
t2605 = ct{190};
t2606 = ct{191};
t2612 = ct{192};
t2613 = ct{193};
t2618 = ct{194};
t2619 = ct{195};
t262 = ct{196};
t264 = ct{197};
t2651 = ct{198};
t2652 = ct{199};
t2670 = ct{200};
t2671 = ct{201};
t2674 = ct{202};
t2676 = ct{203};
t2680 = ct{204};
t2683 = ct{205};
t2684 = ct{206};
t2689 = ct{207};
t2693 = ct{208};
t2694 = ct{209};
t2695 = ct{210};
t2697 = ct{211};
t2698 = ct{212};
t27 = ct{213};
t2700 = ct{214};
t2701 = ct{215};
t2707 = ct{216};
t2712 = ct{217};
t2715 = ct{218};
t2716 = ct{219};
t2719 = ct{220};
t2721 = ct{221};
t2740 = ct{222};
t2747 = ct{223};
t2748 = ct{224};
t2749 = ct{225};
t2754 = ct{226};
t2773 = ct{227};
t2781 = ct{228};
t2788 = ct{229};
t28 = ct{230};
t2801 = ct{231};
t2804 = ct{232};
t2813 = ct{233};
t2814 = ct{234};
t2820 = ct{235};
t2831 = ct{236};
t2834 = ct{237};
t2835 = ct{238};
t2838 = ct{239};
t2850 = ct{240};
t2851 = ct{241};
t29 = ct{242};
t2953 = ct{243};
t2965 = ct{244};
t2966 = ct{245};
t2975 = ct{246};
t2979 = ct{247};
t2990 = ct{248};
t2991 = ct{249};
t2994 = ct{250};
t30 = ct{251};
t3003 = ct{252};
t3009 = ct{253};
t3015 = ct{254};
t3022 = ct{255};
t3027 = ct{256};
t3030 = ct{257};
t3036 = ct{258};
t3043 = ct{259};
t3047 = ct{260};
t3055 = ct{261};
t3057 = ct{262};
t3058 = ct{263};
t3064 = ct{264};
t3068 = ct{265};
t3072 = ct{266};
t3080 = ct{267};
t3096 = ct{268};
t3097 = ct{269};
t31 = ct{270};
t3109 = ct{271};
t3117 = ct{272};
t3118 = ct{273};
t3121 = ct{274};
t3122 = ct{275};
t3126 = ct{276};
t3129 = ct{277};
t313 = ct{278};
t3131 = ct{279};
t3132 = ct{280};
t3133 = ct{281};
t314 = ct{282};
t3142 = ct{283};
t3143 = ct{284};
t3145 = ct{285};
t3148 = ct{286};
t3157 = ct{287};
t3158 = ct{288};
t3171 = ct{289};
t3193 = ct{290};
t3194 = ct{291};
t3195 = ct{292};
t32 = ct{293};
t3200 = ct{294};
t3201 = ct{295};
t3205 = ct{296};
t3208 = ct{297};
t3209 = ct{298};
t321 = ct{299};
t3211 = ct{300};
t3213 = ct{301};
t3216 = ct{302};
t3217 = ct{303};
t3221 = ct{304};
t3235 = ct{305};
t3236 = ct{306};
t3237 = ct{307};
t3238 = ct{308};
t3239 = ct{309};
t3242 = ct{310};
t3257 = ct{311};
t3276 = ct{312};
t3277 = ct{313};
t3279 = ct{314};
t3283 = ct{315};
t329 = ct{316};
t3290 = ct{317};
t3297 = ct{318};
t3298 = ct{319};
t3299 = ct{320};
t33 = ct{321};
t3303 = ct{322};
t3312 = ct{323};
t3313 = ct{324};
t3314 = ct{325};
t3315 = ct{326};
t3318 = ct{327};
t332 = ct{328};
t3322 = ct{329};
t3324 = ct{330};
t3328 = ct{331};
t3329 = ct{332};
t3334 = ct{333};
t3337 = ct{334};
t3340 = ct{335};
t3344 = ct{336};
t3346 = ct{337};
t335 = ct{338};
t3351 = ct{339};
t3359 = ct{340};
t3367 = ct{341};
t3369 = ct{342};
t3370 = ct{343};
t3386 = ct{344};
t3395 = ct{345};
t3396 = ct{346};
t34 = ct{347};
t3405 = ct{348};
t3409 = ct{349};
t3415 = ct{350};
t3416 = ct{351};
t3420 = ct{352};
t3423 = ct{353};
t3428 = ct{354};
t3431 = ct{355};
t3432 = ct{356};
t3434 = ct{357};
t3435 = ct{358};
t3446 = ct{359};
t3448 = ct{360};
t346 = ct{361};
t3463 = ct{362};
t3468 = ct{363};
t3471 = ct{364};
t3474 = ct{365};
t3480 = ct{366};
t3482 = ct{367};
t3483 = ct{368};
t3488 = ct{369};
t3489 = ct{370};
t3490 = ct{371};
t3492 = ct{372};
t3495 = ct{373};
t3496 = ct{374};
t3498 = ct{375};
t3499 = ct{376};
t35 = ct{377};
t350 = ct{378};
t3500 = ct{379};
t3502 = ct{380};
t3503 = ct{381};
t3512 = ct{382};
t3517 = ct{383};
t3524 = ct{384};
t354 = ct{385};
t3541 = ct{386};
t3543 = ct{387};
t3545 = ct{388};
t3546 = ct{389};
t3547 = ct{390};
t3549 = ct{391};
t3551 = ct{392};
t3552 = ct{393};
t3554 = ct{394};
t3558 = ct{395};
t3561 = ct{396};
t3563 = ct{397};
t3566 = ct{398};
t3582 = ct{399};
t3588 = ct{400};
t3590 = ct{401};
t3591 = ct{402};
t3592 = ct{403};
t3597 = ct{404};
t36 = ct{405};
t3603 = ct{406};
t3609 = ct{407};
t3610 = ct{408};
t3611 = ct{409};
t3614 = ct{410};
t3617 = ct{411};
t3624 = ct{412};
t3637 = ct{413};
t3638 = ct{414};
t3639 = ct{415};
t3640 = ct{416};
t3641 = ct{417};
t3642 = ct{418};
t3643 = ct{419};
t3649 = ct{420};
t3655 = ct{421};
t3656 = ct{422};
t3658 = ct{423};
t3659 = ct{424};
t366 = ct{425};
t3660 = ct{426};
t3664 = ct{427};
t3670 = ct{428};
t3678 = ct{429};
t3688 = ct{430};
t3689 = ct{431};
t3690 = ct{432};
t3692 = ct{433};
t3693 = ct{434};
t3695 = ct{435};
t3696 = ct{436};
t3697 = ct{437};
t3699 = ct{438};
t3703 = ct{439};
t3704 = ct{440};
t3705 = ct{441};
t3706 = ct{442};
t3707 = ct{443};
t3708 = ct{444};
t3709 = ct{445};
t3710 = ct{446};
t3712 = ct{447};
t3713 = ct{448};
t3716 = ct{449};
t3717 = ct{450};
t3728 = ct{451};
t3729 = ct{452};
t3732 = ct{453};
t3736 = ct{454};
t3738 = ct{455};
t3739 = ct{456};
t3746 = ct{457};
t3747 = ct{458};
t3752 = ct{459};
t3755 = ct{460};
t3765 = ct{461};
t3766 = ct{462};
t3770 = ct{463};
t3771 = ct{464};
t3772 = ct{465};
t3774 = ct{466};
t3775 = ct{467};
t3777 = ct{468};
t3779 = ct{469};
t3781 = ct{470};
t3782 = ct{471};
t3783 = ct{472};
t3784 = ct{473};
t3785 = ct{474};
t3786 = ct{475};
t3788 = ct{476};
t3789 = ct{477};
t3790 = ct{478};
t3791 = ct{479};
t3792 = ct{480};
t3793 = ct{481};
t3794 = ct{482};
t3795 = ct{483};
t3796 = ct{484};
t3797 = ct{485};
t3798 = ct{486};
t38 = ct{487};
t3800 = ct{488};
t3801 = ct{489};
t3802 = ct{490};
t3804 = ct{491};
t3805 = ct{492};
t3808 = ct{493};
t3809 = ct{494};
t3810 = ct{495};
t3817 = ct{496};
t3818 = ct{497};
t3820 = ct{498};
t3821 = ct{499};
t3823 = ct{500};
t3824 = ct{501};
t3826 = ct{502};
t3827 = ct{503};
t3828 = ct{504};
t3830 = ct{505};
t3832 = ct{506};
t3833 = ct{507};
t3835 = ct{508};
t3840 = ct{509};
t3843 = ct{510};
t3844 = ct{511};
t3845 = ct{512};
t3846 = ct{513};
t3848 = ct{514};
t3850 = ct{515};
t3851 = ct{516};
t3855 = ct{517};
t3856 = ct{518};
t3857 = ct{519};
t3862 = ct{520};
t3863 = ct{521};
t387 = ct{522};
t3876 = ct{523};
t3877 = ct{524};
t3878 = ct{525};
t3879 = ct{526};
t3880 = ct{527};
t3890 = ct{528};
t3891 = ct{529};
t3893 = ct{530};
t3895 = ct{531};
t3896 = ct{532};
t3897 = ct{533};
t3898 = ct{534};
t39 = ct{535};
t3901 = ct{536};
t3902 = ct{537};
t3903 = ct{538};
t3906 = ct{539};
t3908 = ct{540};
t3910 = ct{541};
t3913 = ct{542};
t3915 = ct{543};
t3924 = ct{544};
t3925 = ct{545};
t3926 = ct{546};
t3931 = ct{547};
t3934 = ct{548};
t3937 = ct{549};
t3943 = ct{550};
t3951 = ct{551};
t3961 = ct{552};
t3967 = ct{553};
t3968 = ct{554};
t3974 = ct{555};
t3975 = ct{556};
t3976 = ct{557};
t3980 = ct{558};
t3985 = ct{559};
t3991 = ct{560};
t3993 = ct{561};
t4001 = ct{562};
t4006 = ct{563};
t4008 = ct{564};
t4018 = ct{565};
t4019 = ct{566};
t4026 = ct{567};
t4030 = ct{568};
t4031 = ct{569};
t4032 = ct{570};
t4035 = ct{571};
t4039 = ct{572};
t4041 = ct{573};
t4045 = ct{574};
t4047 = ct{575};
t4049 = ct{576};
t4051 = ct{577};
t4053 = ct{578};
t4054 = ct{579};
t4065 = ct{580};
t4081 = ct{581};
t4082 = ct{582};
t410 = ct{583};
t4100 = ct{584};
t4109 = ct{585};
t4110 = ct{586};
t4114 = ct{587};
t4115 = ct{588};
t4118 = ct{589};
t4135 = ct{590};
t4136 = ct{591};
t4144 = ct{592};
t4146 = ct{593};
t4147 = ct{594};
t4151 = ct{595};
t4153 = ct{596};
t4154 = ct{597};
t4157 = ct{598};
t4158 = ct{599};
t4163 = ct{600};
t4165 = ct{601};
t4171 = ct{602};
t4172 = ct{603};
t4184 = ct{604};
t4187 = ct{605};
t4190 = ct{606};
t4191 = ct{607};
t4193 = ct{608};
t4198 = ct{609};
t42 = ct{610};
t4201 = ct{611};
t4205 = ct{612};
t4208 = ct{613};
t4213 = ct{614};
t4215 = ct{615};
t4236 = ct{616};
t4240 = ct{617};
t4244 = ct{618};
t4260 = ct{619};
t4261 = ct{620};
t4263 = ct{621};
t4270 = ct{622};
t4272 = ct{623};
t4273 = ct{624};
t4274 = ct{625};
t4275 = ct{626};
t4281 = ct{627};
t4282 = ct{628};
t4286 = ct{629};
t4287 = ct{630};
t4288 = ct{631};
t4289 = ct{632};
t4290 = ct{633};
t4291 = ct{634};
t4292 = ct{635};
t4299 = ct{636};
t43 = ct{637};
t4300 = ct{638};
t4301 = ct{639};
t4303 = ct{640};
t4308 = ct{641};
t4310 = ct{642};
t4313 = ct{643};
t4314 = ct{644};
t4318 = ct{645};
t4321 = ct{646};
t4324 = ct{647};
t4325 = ct{648};
t4326 = ct{649};
t4330 = ct{650};
t4332 = ct{651};
t4334 = ct{652};
t4337 = ct{653};
t4339 = ct{654};
t4341 = ct{655};
t4342 = ct{656};
t4343 = ct{657};
t4345 = ct{658};
t4346 = ct{659};
t4352 = ct{660};
t4356 = ct{661};
t4358 = ct{662};
t4359 = ct{663};
t4361 = ct{664};
t4364 = ct{665};
t4368 = ct{666};
t4371 = ct{667};
t4372 = ct{668};
t4373 = ct{669};
t4375 = ct{670};
t4406 = ct{671};
t4413 = ct{672};
t4415 = ct{673};
t4416 = ct{674};
t4417 = ct{675};
t4458 = ct{676};
t4459 = ct{677};
t4461 = ct{678};
t4464 = ct{679};
t4468 = ct{680};
t4470 = ct{681};
t4476 = ct{682};
t4486 = ct{683};
t4488 = ct{684};
t4489 = ct{685};
t4493 = ct{686};
t4494 = ct{687};
t4495 = ct{688};
t4501 = ct{689};
t4502 = ct{690};
t4504 = ct{691};
t4515 = ct{692};
t4518 = ct{693};
t4520 = ct{694};
t4522 = ct{695};
t4537 = ct{696};
t4545 = ct{697};
t4553 = ct{698};
t4559 = ct{699};
t4562 = ct{700};
t4563 = ct{701};
t4567 = ct{702};
t4570 = ct{703};
t4573 = ct{704};
t4576 = ct{705};
t4577 = ct{706};
t4582 = ct{707};
t4583 = ct{708};
t4594 = ct{709};
t46 = ct{710};
t4603 = ct{711};
t4604 = ct{712};
t4606 = ct{713};
t4615 = ct{714};
t4617 = ct{715};
t4618 = ct{716};
t4619 = ct{717};
t4623 = ct{718};
t4634 = ct{719};
t4635 = ct{720};
t4639 = ct{721};
t4644 = ct{722};
t4645 = ct{723};
t4651 = ct{724};
t4652 = ct{725};
t4658 = ct{726};
t4663 = ct{727};
t4665 = ct{728};
t4673 = ct{729};
t4675 = ct{730};
t4676 = ct{731};
t4677 = ct{732};
t4678 = ct{733};
t4680 = ct{734};
t4683 = ct{735};
t4691 = ct{736};
t4692 = ct{737};
t4694 = ct{738};
t4696 = ct{739};
t4697 = ct{740};
t4698 = ct{741};
t47 = ct{742};
t4700 = ct{743};
t4702 = ct{744};
t4703 = ct{745};
t4704 = ct{746};
t4705 = ct{747};
t4708 = ct{748};
t4709 = ct{749};
t4713 = ct{750};
t4716 = ct{751};
t4719 = ct{752};
t4722 = ct{753};
t4724 = ct{754};
t4725 = ct{755};
t4727 = ct{756};
t4728 = ct{757};
t4730 = ct{758};
t4741 = ct{759};
t4744 = ct{760};
t4746 = ct{761};
t4751 = ct{762};
t4757 = ct{763};
t4760 = ct{764};
t4761 = ct{765};
t4762 = ct{766};
t4763 = ct{767};
t4795 = ct{768};
t4799 = ct{769};
t4801 = ct{770};
t4808 = ct{771};
t4809 = ct{772};
t4814 = ct{773};
t4823 = ct{774};
t4828 = ct{775};
t4833 = ct{776};
t4835 = ct{777};
t4838 = ct{778};
t4843 = ct{779};
t4844 = ct{780};
t4846 = ct{781};
t4847 = ct{782};
t4850 = ct{783};
t4851 = ct{784};
t4852 = ct{785};
t4853 = ct{786};
t4854 = ct{787};
t4856 = ct{788};
t4857 = ct{789};
t4858 = ct{790};
t4859 = ct{791};
t4860 = ct{792};
t4862 = ct{793};
t4863 = ct{794};
t4864 = ct{795};
t4865 = ct{796};
t4866 = ct{797};
t4867 = ct{798};
t4868 = ct{799};
t4870 = ct{800};
t4872 = ct{801};
t4874 = ct{802};
t4876 = ct{803};
t4879 = ct{804};
t4880 = ct{805};
t4887 = ct{806};
t4888 = ct{807};
t4889 = ct{808};
t4893 = ct{809};
t4895 = ct{810};
t4896 = ct{811};
t4898 = ct{812};
t4901 = ct{813};
t4902 = ct{814};
t4903 = ct{815};
t4904 = ct{816};
t4905 = ct{817};
t4906 = ct{818};
t4907 = ct{819};
t4908 = ct{820};
t4911 = ct{821};
t4912 = ct{822};
t4913 = ct{823};
t4914 = ct{824};
t4915 = ct{825};
t4920 = ct{826};
t4923 = ct{827};
t4924 = ct{828};
t4925 = ct{829};
t4927 = ct{830};
t4928 = ct{831};
t4935 = ct{832};
t4936 = ct{833};
t4950 = ct{834};
t4952 = ct{835};
t4953 = ct{836};
t4955 = ct{837};
t4957 = ct{838};
t4958 = ct{839};
t4959 = ct{840};
t4961 = ct{841};
t4963 = ct{842};
t4965 = ct{843};
t4967 = ct{844};
t4969 = ct{845};
t4970 = ct{846};
t4971 = ct{847};
t4972 = ct{848};
t4973 = ct{849};
t4974 = ct{850};
t4976 = ct{851};
t4977 = ct{852};
t4978 = ct{853};
t4979 = ct{854};
t4981 = ct{855};
t4982 = ct{856};
t4983 = ct{857};
t4984 = ct{858};
t4985 = ct{859};
t4986 = ct{860};
t4987 = ct{861};
t4989 = ct{862};
t4990 = ct{863};
t4991 = ct{864};
t4992 = ct{865};
t4993 = ct{866};
t4994 = ct{867};
t4995 = ct{868};
t4996 = ct{869};
t4997 = ct{870};
t4998 = ct{871};
t4999 = ct{872};
t50 = ct{873};
t5001 = ct{874};
t5003 = ct{875};
t5004 = ct{876};
t5005 = ct{877};
t5007 = ct{878};
t5009 = ct{879};
t5010 = ct{880};
t5011 = ct{881};
t5012 = ct{882};
t5013 = ct{883};
t5014 = ct{884};
t5016 = ct{885};
t5021 = ct{886};
t5023 = ct{887};
t5025 = ct{888};
t5026 = ct{889};
t5027 = ct{890};
t5028 = ct{891};
t5031 = ct{892};
t5032 = ct{893};
t5033 = ct{894};
t5034 = ct{895};
t5035 = ct{896};
t5036 = ct{897};
t5037 = ct{898};
t5038 = ct{899};
t5041 = ct{900};
t5042 = ct{901};
t5043 = ct{902};
t5045 = ct{903};
t5046 = ct{904};
t5049 = ct{905};
t5051 = ct{906};
t5056 = ct{907};
t5057 = ct{908};
t5062 = ct{909};
t5063 = ct{910};
t5080 = ct{911};
t5082 = ct{912};
t5083 = ct{913};
t5084 = ct{914};
t5085 = ct{915};
t5086 = ct{916};
t5087 = ct{917};
t5088 = ct{918};
t5089 = ct{919};
t5090 = ct{920};
t5091 = ct{921};
t5093 = ct{922};
t5096 = ct{923};
t5097 = ct{924};
t5098 = ct{925};
t5103 = ct{926};
t5105 = ct{927};
t5106 = ct{928};
t5108 = ct{929};
t5109 = ct{930};
t5112 = ct{931};
t5113 = ct{932};
t5116 = ct{933};
t5117 = ct{934};
t5118 = ct{935};
t5119 = ct{936};
t5120 = ct{937};
t5121 = ct{938};
t5123 = ct{939};
t5124 = ct{940};
t5125 = ct{941};
t5126 = ct{942};
t5127 = ct{943};
t5128 = ct{944};
t5129 = ct{945};
t5130 = ct{946};
t5131 = ct{947};
t5133 = ct{948};
t5134 = ct{949};
t5135 = ct{950};
t5136 = ct{951};
t5137 = ct{952};
t5138 = ct{953};
t5139 = ct{954};
t5141 = ct{955};
t5142 = ct{956};
t5151 = ct{957};
t5152 = ct{958};
t5153 = ct{959};
t5154 = ct{960};
t5155 = ct{961};
t5156 = ct{962};
t5158 = ct{963};
t5159 = ct{964};
t5161 = ct{965};
t5162 = ct{966};
t5163 = ct{967};
t5164 = ct{968};
t5166 = ct{969};
t5167 = ct{970};
t5169 = ct{971};
t5182 = ct{972};
t5183 = ct{973};
t5184 = ct{974};
t5185 = ct{975};
t5186 = ct{976};
t5187 = ct{977};
t5188 = ct{978};
t5189 = ct{979};
t5190 = ct{980};
t5191 = ct{981};
t5192 = ct{982};
t5193 = ct{983};
t5194 = ct{984};
t5197 = ct{985};
t5198 = ct{986};
t5199 = ct{987};
t5200 = ct{988};
t5201 = ct{989};
t5202 = ct{990};
t5205 = ct{991};
t5206 = ct{992};
t5207 = ct{993};
t5208 = ct{994};
t5211 = ct{995};
t5212 = ct{996};
t5213 = ct{997};
t5214 = ct{998};
t5216 = ct{999};
t5220 = ct{1000};
t5221 = ct{1001};
t5222 = ct{1002};
t5223 = ct{1003};
t5231 = ct{1004};
t5232 = ct{1005};
t5233 = ct{1006};
t5234 = ct{1007};
t5235 = ct{1008};
t5236 = ct{1009};
t5237 = ct{1010};
t5238 = ct{1011};
t5240 = ct{1012};
t5243 = ct{1013};
t5246 = ct{1014};
t5247 = ct{1015};
t5248 = ct{1016};
t5249 = ct{1017};
t5251 = ct{1018};
t5254 = ct{1019};
t5255 = ct{1020};
t5256 = ct{1021};
t5257 = ct{1022};
t5258 = ct{1023};
t5259 = ct{1024};
t5262 = ct{1025};
t5264 = ct{1026};
t5265 = ct{1027};
t5275 = ct{1028};
t5278 = ct{1029};
t5279 = ct{1030};
t5280 = ct{1031};
t5281 = ct{1032};
t5283 = ct{1033};
t5286 = ct{1034};
t5287 = ct{1035};
t5291 = ct{1036};
t5296 = ct{1037};
t5297 = ct{1038};
t5301 = ct{1039};
t5302 = ct{1040};
t5303 = ct{1041};
t5304 = ct{1042};
t5305 = ct{1043};
t5306 = ct{1044};
t5308 = ct{1045};
t5309 = ct{1046};
t5312 = ct{1047};
t5313 = ct{1048};
t5317 = ct{1049};
t5328 = ct{1050};
t5331 = ct{1051};
t5332 = ct{1052};
t5333 = ct{1053};
t5336 = ct{1054};
t5337 = ct{1055};
t5340 = ct{1056};
t5341 = ct{1057};
t5343 = ct{1058};
t5344 = ct{1059};
t5345 = ct{1060};
t5346 = ct{1061};
t5348 = ct{1062};
t5350 = ct{1063};
t5352 = ct{1064};
t5353 = ct{1065};
t5356 = ct{1066};
t5358 = ct{1067};
t5359 = ct{1068};
t5361 = ct{1069};
t5362 = ct{1070};
t5363 = ct{1071};
t5365 = ct{1072};
t5367 = ct{1073};
t5369 = ct{1074};
t5370 = ct{1075};
t5372 = ct{1076};
t5373 = ct{1077};
t5374 = ct{1078};
t5376 = ct{1079};
t5377 = ct{1080};
t5380 = ct{1081};
t5381 = ct{1082};
t5382 = ct{1083};
t5383 = ct{1084};
t5384 = ct{1085};
t5385 = ct{1086};
t5386 = ct{1087};
t5387 = ct{1088};
t5389 = ct{1089};
t5390 = ct{1090};
t5391 = ct{1091};
t5392 = ct{1092};
t5393 = ct{1093};
t5395 = ct{1094};
t5398 = ct{1095};
t5399 = ct{1096};
t5400 = ct{1097};
t5401 = ct{1098};
t5402 = ct{1099};
t5403 = ct{1100};
t5404 = ct{1101};
t5405 = ct{1102};
t5410 = ct{1103};
t5411 = ct{1104};
t5412 = ct{1105};
t5413 = ct{1106};
t5415 = ct{1107};
t5416 = ct{1108};
t5419 = ct{1109};
t5421 = ct{1110};
t5422 = ct{1111};
t5425 = ct{1112};
t5427 = ct{1113};
t5433 = ct{1114};
t5434 = ct{1115};
t5436 = ct{1116};
t5437 = ct{1117};
t5438 = ct{1118};
t5439 = ct{1119};
t5440 = ct{1120};
t5441 = ct{1121};
t5442 = ct{1122};
t5443 = ct{1123};
t5444 = ct{1124};
t5445 = ct{1125};
t5446 = ct{1126};
t5448 = ct{1127};
t5449 = ct{1128};
t5451 = ct{1129};
t5452 = ct{1130};
t5453 = ct{1131};
t5455 = ct{1132};
t5456 = ct{1133};
t5457 = ct{1134};
t5458 = ct{1135};
t5459 = ct{1136};
t5460 = ct{1137};
t5464 = ct{1138};
t5465 = ct{1139};
t5466 = ct{1140};
t5467 = ct{1141};
t5468 = ct{1142};
t5470 = ct{1143};
t5472 = ct{1144};
t5473 = ct{1145};
t5474 = ct{1146};
t5475 = ct{1147};
t5476 = ct{1148};
t5477 = ct{1149};
t5478 = ct{1150};
t5480 = ct{1151};
t5481 = ct{1152};
t5483 = ct{1153};
t5486 = ct{1154};
t5487 = ct{1155};
t5488 = ct{1156};
t5489 = ct{1157};
t5490 = ct{1158};
t5491 = ct{1159};
t5493 = ct{1160};
t5494 = ct{1161};
t5495 = ct{1162};
t5497 = ct{1163};
t5499 = ct{1164};
t5500 = ct{1165};
t5501 = ct{1166};
t5502 = ct{1167};
t5503 = ct{1168};
t5504 = ct{1169};
t5505 = ct{1170};
t5506 = ct{1171};
t5507 = ct{1172};
t5508 = ct{1173};
t5509 = ct{1174};
t5510 = ct{1175};
t5511 = ct{1176};
t5512 = ct{1177};
t5513 = ct{1178};
t5514 = ct{1179};
t5515 = ct{1180};
t5516 = ct{1181};
t5517 = ct{1182};
t5518 = ct{1183};
t5519 = ct{1184};
t5520 = ct{1185};
t5521 = ct{1186};
t5523 = ct{1187};
t5535 = ct{1188};
t5536 = ct{1189};
t5537 = ct{1190};
t5538 = ct{1191};
t5539 = ct{1192};
t5542 = ct{1193};
t5543 = ct{1194};
t5544 = ct{1195};
t5545 = ct{1196};
t5546 = ct{1197};
t5548 = ct{1198};
t5549 = ct{1199};
t5550 = ct{1200};
t5551 = ct{1201};
t5552 = ct{1202};
t5553 = ct{1203};
t5554 = ct{1204};
t5555 = ct{1205};
t5556 = ct{1206};
t5557 = ct{1207};
t5558 = ct{1208};
t5560 = ct{1209};
t5563 = ct{1210};
t5564 = ct{1211};
t5565 = ct{1212};
t5567 = ct{1213};
t5568 = ct{1214};
t5569 = ct{1215};
t5570 = ct{1216};
t5572 = ct{1217};
t5573 = ct{1218};
t5574 = ct{1219};
t5575 = ct{1220};
t5576 = ct{1221};
t5577 = ct{1222};
t5578 = ct{1223};
t5579 = ct{1224};
t5580 = ct{1225};
t5581 = ct{1226};
t5583 = ct{1227};
t5585 = ct{1228};
t5586 = ct{1229};
t5587 = ct{1230};
t5588 = ct{1231};
t5589 = ct{1232};
t5590 = ct{1233};
t5591 = ct{1234};
t5592 = ct{1235};
t5593 = ct{1236};
t5594 = ct{1237};
t5596 = ct{1238};
t5597 = ct{1239};
t5598 = ct{1240};
t5599 = ct{1241};
t56 = ct{1242};
t5600 = ct{1243};
t5601 = ct{1244};
t5602 = ct{1245};
t5603 = ct{1246};
t5604 = ct{1247};
t5605 = ct{1248};
t5606 = ct{1249};
t5607 = ct{1250};
t5608 = ct{1251};
t5609 = ct{1252};
t5611 = ct{1253};
t5612 = ct{1254};
t5613 = ct{1255};
t5614 = ct{1256};
t5615 = ct{1257};
t5616 = ct{1258};
t5618 = ct{1259};
t5619 = ct{1260};
t5622 = ct{1261};
t5623 = ct{1262};
t5624 = ct{1263};
t5625 = ct{1264};
t5626 = ct{1265};
t5628 = ct{1266};
t5629 = ct{1267};
t5630 = ct{1268};
t5631 = ct{1269};
t5632 = ct{1270};
t5633 = ct{1271};
t5634 = ct{1272};
t5635 = ct{1273};
t5636 = ct{1274};
t5637 = ct{1275};
t5638 = ct{1276};
t5641 = ct{1277};
t5642 = ct{1278};
t5645 = ct{1279};
t5646 = ct{1280};
t5647 = ct{1281};
t5649 = ct{1282};
t5650 = ct{1283};
t5651 = ct{1284};
t5652 = ct{1285};
t5653 = ct{1286};
t5655 = ct{1287};
t5658 = ct{1288};
t5659 = ct{1289};
t5661 = ct{1290};
t5663 = ct{1291};
t5669 = ct{1292};
t5670 = ct{1293};
t5672 = ct{1294};
t5673 = ct{1295};
t5675 = ct{1296};
t5677 = ct{1297};
t5678 = ct{1298};
t5679 = ct{1299};
t5680 = ct{1300};
t5681 = ct{1301};
t5682 = ct{1302};
t5683 = ct{1303};
t5684 = ct{1304};
t5685 = ct{1305};
t5686 = ct{1306};
t5687 = ct{1307};
t5688 = ct{1308};
t5689 = ct{1309};
t5690 = ct{1310};
t5691 = ct{1311};
t5694 = ct{1312};
t5695 = ct{1313};
t5698 = ct{1314};
t5699 = ct{1315};
t5706 = ct{1316};
t5709 = ct{1317};
t5710 = ct{1318};
t5711 = ct{1319};
t5712 = ct{1320};
t5713 = ct{1321};
t5714 = ct{1322};
t5716 = ct{1323};
t5717 = ct{1324};
t5718 = ct{1325};
t5720 = ct{1326};
t5721 = ct{1327};
t5722 = ct{1328};
t5723 = ct{1329};
t5724 = ct{1330};
t5725 = ct{1331};
t5730 = ct{1332};
t5731 = ct{1333};
t5734 = ct{1334};
t5735 = ct{1335};
t5738 = ct{1336};
t5739 = ct{1337};
t5741 = ct{1338};
t5742 = ct{1339};
t5745 = ct{1340};
t5747 = ct{1341};
t5751 = ct{1342};
t5753 = ct{1343};
t5754 = ct{1344};
t5756 = ct{1345};
t5758 = ct{1346};
t5759 = ct{1347};
t5760 = ct{1348};
t5761 = ct{1349};
t5762 = ct{1350};
t5763 = ct{1351};
t5764 = ct{1352};
t5765 = ct{1353};
t5766 = ct{1354};
t5768 = ct{1355};
t5769 = ct{1356};
t5770 = ct{1357};
t5772 = ct{1358};
t5773 = ct{1359};
t5774 = ct{1360};
t5775 = ct{1361};
t5776 = ct{1362};
t5777 = ct{1363};
t5778 = ct{1364};
t5779 = ct{1365};
t5781 = ct{1366};
t5782 = ct{1367};
t5783 = ct{1368};
t5784 = ct{1369};
t5787 = ct{1370};
t5788 = ct{1371};
t5790 = ct{1372};
t5792 = ct{1373};
t5793 = ct{1374};
t5794 = ct{1375};
t5795 = ct{1376};
t5796 = ct{1377};
t5798 = ct{1378};
t5799 = ct{1379};
t5801 = ct{1380};
t5802 = ct{1381};
t5804 = ct{1382};
t5809 = ct{1383};
t5810 = ct{1384};
t5813 = ct{1385};
t5814 = ct{1386};
t5816 = ct{1387};
t5817 = ct{1388};
t5819 = ct{1389};
t5821 = ct{1390};
t5825 = ct{1391};
t5826 = ct{1392};
t5827 = ct{1393};
t5828 = ct{1394};
t5829 = ct{1395};
t5831 = ct{1396};
t5832 = ct{1397};
t5833 = ct{1398};
t5835 = ct{1399};
t5836 = ct{1400};
t5837 = ct{1401};
t5838 = ct{1402};
t5839 = ct{1403};
t5840 = ct{1404};
t5842 = ct{1405};
t5844 = ct{1406};
t5845 = ct{1407};
t5846 = ct{1408};
t5849 = ct{1409};
t5851 = ct{1410};
t5852 = ct{1411};
t5853 = ct{1412};
t5855 = ct{1413};
t5856 = ct{1414};
t5857 = ct{1415};
t5858 = ct{1416};
t5863 = ct{1417};
t5864 = ct{1418};
t5867 = ct{1419};
t5868 = ct{1420};
t5869 = ct{1421};
t5871 = ct{1422};
t5872 = ct{1423};
t5874 = ct{1424};
t5875 = ct{1425};
t5876 = ct{1426};
t5877 = ct{1427};
t5878 = ct{1428};
t5879 = ct{1429};
t5880 = ct{1430};
t5881 = ct{1431};
t5884 = ct{1432};
t5886 = ct{1433};
t5888 = ct{1434};
t5890 = ct{1435};
t5891 = ct{1436};
t5892 = ct{1437};
t5893 = ct{1438};
t5894 = ct{1439};
t5896 = ct{1440};
t5897 = ct{1441};
t5898 = ct{1442};
t5899 = ct{1443};
t5900 = ct{1444};
t5901 = ct{1445};
t5902 = ct{1446};
t5904 = ct{1447};
t5905 = ct{1448};
t5906 = ct{1449};
t5907 = ct{1450};
t5908 = ct{1451};
t5909 = ct{1452};
t5910 = ct{1453};
t5911 = ct{1454};
t5912 = ct{1455};
t5913 = ct{1456};
t5914 = ct{1457};
t5915 = ct{1458};
t5916 = ct{1459};
t5917 = ct{1460};
t5918 = ct{1461};
t5919 = ct{1462};
t5920 = ct{1463};
t5922 = ct{1464};
t5923 = ct{1465};
t5924 = ct{1466};
t5925 = ct{1467};
t5926 = ct{1468};
t5927 = ct{1469};
t5928 = ct{1470};
t5930 = ct{1471};
t5931 = ct{1472};
t5933 = ct{1473};
t5934 = ct{1474};
t5935 = ct{1475};
t5937 = ct{1476};
t5938 = ct{1477};
t5939 = ct{1478};
t5941 = ct{1479};
t5942 = ct{1480};
t5943 = ct{1481};
t5945 = ct{1482};
t5946 = ct{1483};
t5947 = ct{1484};
t5948 = ct{1485};
t5949 = ct{1486};
t5950 = ct{1487};
t5951 = ct{1488};
t5954 = ct{1489};
t5955 = ct{1490};
t5956 = ct{1491};
t5959 = ct{1492};
t5960 = ct{1493};
t5963 = ct{1494};
t5965 = ct{1495};
t5966 = ct{1496};
t5967 = ct{1497};
t5968 = ct{1498};
t5971 = ct{1499};
t5973 = ct{1500};
t5974 = ct{1501};
t5975 = ct{1502};
t5976 = ct{1503};
t5978 = ct{1504};
t5979 = ct{1505};
t5980 = ct{1506};
t5981 = ct{1507};
t5982 = ct{1508};
t5983 = ct{1509};
t5984 = ct{1510};
t5985 = ct{1511};
t5986 = ct{1512};
t5988 = ct{1513};
t5990 = ct{1514};
t5992 = ct{1515};
t5993 = ct{1516};
t5997 = ct{1517};
t5999 = ct{1518};
t60 = ct{1519};
t6000 = ct{1520};
t6001 = ct{1521};
t6004 = ct{1522};
t6005 = ct{1523};
t6006 = ct{1524};
t6007 = ct{1525};
t6008 = ct{1526};
t6009 = ct{1527};
t6011 = ct{1528};
t6013 = ct{1529};
t6014 = ct{1530};
t6015 = ct{1531};
t6017 = ct{1532};
t6018 = ct{1533};
t6019 = ct{1534};
t6020 = ct{1535};
t6021 = ct{1536};
t6022 = ct{1537};
t6023 = ct{1538};
t6024 = ct{1539};
t6026 = ct{1540};
t6027 = ct{1541};
t6028 = ct{1542};
t6029 = ct{1543};
t6031 = ct{1544};
t6034 = ct{1545};
t6035 = ct{1546};
t6037 = ct{1547};
t6038 = ct{1548};
t6039 = ct{1549};
t6041 = ct{1550};
t6043 = ct{1551};
t6045 = ct{1552};
t6046 = ct{1553};
t6047 = ct{1554};
t6050 = ct{1555};
t6052 = ct{1556};
t6053 = ct{1557};
t6054 = ct{1558};
t6055 = ct{1559};
t6058 = ct{1560};
t6059 = ct{1561};
t6060 = ct{1562};
t6062 = ct{1563};
t6064 = ct{1564};
t6065 = ct{1565};
t6066 = ct{1566};
t6067 = ct{1567};
t6074 = ct{1568};
t6076 = ct{1569};
t6079 = ct{1570};
t6080 = ct{1571};
t6081 = ct{1572};
t6082 = ct{1573};
t6083 = ct{1574};
t6084 = ct{1575};
t6091 = ct{1576};
t6093 = ct{1577};
t6094 = ct{1578};
t6095 = ct{1579};
t6096 = ct{1580};
t6098 = ct{1581};
t6099 = ct{1582};
t6100 = ct{1583};
t6102 = ct{1584};
t6106 = ct{1585};
t6107 = ct{1586};
t6109 = ct{1587};
t6110 = ct{1588};
t6111 = ct{1589};
t6113 = ct{1590};
t6114 = ct{1591};
t6115 = ct{1592};
t6116 = ct{1593};
t6119 = ct{1594};
t6120 = ct{1595};
t6125 = ct{1596};
t6129 = ct{1597};
t6131 = ct{1598};
t6133 = ct{1599};
t6134 = ct{1600};
t6135 = ct{1601};
t6136 = ct{1602};
t6137 = ct{1603};
t6138 = ct{1604};
t6140 = ct{1605};
t6143 = ct{1606};
t6144 = ct{1607};
t6145 = ct{1608};
t6148 = ct{1609};
t6159 = ct{1610};
t6162 = ct{1611};
t6164 = ct{1612};
t6166 = ct{1613};
t6168 = ct{1614};
t6169 = ct{1615};
t6170 = ct{1616};
t6171 = ct{1617};
t6172 = ct{1618};
t6173 = ct{1619};
t6174 = ct{1620};
t6175 = ct{1621};
t6180 = ct{1622};
t6183 = ct{1623};
t6184 = ct{1624};
t6185 = ct{1625};
t6186 = ct{1626};
t6187 = ct{1627};
t6190 = ct{1628};
t6191 = ct{1629};
t6192 = ct{1630};
t6193 = ct{1631};
t6196 = ct{1632};
t6197 = ct{1633};
t6199 = ct{1634};
t6205 = ct{1635};
t6206 = ct{1636};
t6207 = ct{1637};
t6208 = ct{1638};
t6211 = ct{1639};
t6213 = ct{1640};
t6215 = ct{1641};
t6216 = ct{1642};
t6217 = ct{1643};
t6219 = ct{1644};
t6223 = ct{1645};
t6225 = ct{1646};
t6226 = ct{1647};
t6227 = ct{1648};
t6228 = ct{1649};
t6231 = ct{1650};
t6232 = ct{1651};
t6233 = ct{1652};
t6234 = ct{1653};
t6237 = ct{1654};
t6239 = ct{1655};
t6240 = ct{1656};
t6241 = ct{1657};
t6242 = ct{1658};
t6244 = ct{1659};
t6250 = ct{1660};
t6251 = ct{1661};
t6252 = ct{1662};
t6254 = ct{1663};
t6255 = ct{1664};
t6256 = ct{1665};
t6257 = ct{1666};
t6262 = ct{1667};
t6263 = ct{1668};
t6267 = ct{1669};
t6270 = ct{1670};
t6271 = ct{1671};
t6272 = ct{1672};
t6275 = ct{1673};
t6276 = ct{1674};
t6281 = ct{1675};
t6282 = ct{1676};
t6283 = ct{1677};
t6284 = ct{1678};
t6285 = ct{1679};
t6286 = ct{1680};
t6287 = ct{1681};
t6288 = ct{1682};
t6290 = ct{1683};
t6291 = ct{1684};
t6292 = ct{1685};
t6293 = ct{1686};
t6294 = ct{1687};
t6303 = ct{1688};
t6304 = ct{1689};
t6306 = ct{1690};
t6307 = ct{1691};
t6308 = ct{1692};
t6310 = ct{1693};
t6311 = ct{1694};
t6313 = ct{1695};
t6314 = ct{1696};
t6316 = ct{1697};
t6317 = ct{1698};
t6318 = ct{1699};
t6324 = ct{1700};
t6325 = ct{1701};
t6327 = ct{1702};
t6329 = ct{1703};
t6331 = ct{1704};
t6334 = ct{1705};
t6337 = ct{1706};
t6338 = ct{1707};
t6339 = ct{1708};
t6342 = ct{1709};
t6343 = ct{1710};
t6345 = ct{1711};
t6347 = ct{1712};
t6348 = ct{1713};
t6354 = ct{1714};
t6356 = ct{1715};
t6360 = ct{1716};
t6366 = ct{1717};
t6367 = ct{1718};
t6369 = ct{1719};
t6375 = ct{1720};
t6376 = ct{1721};
t6377 = ct{1722};
t6379 = ct{1723};
t6384 = ct{1724};
t6387 = ct{1725};
t6394 = ct{1726};
t6396 = ct{1727};
t6398 = ct{1728};
t640 = ct{1729};
t6402 = ct{1730};
t6404 = ct{1731};
t6405 = ct{1732};
t6406 = ct{1733};
t6407 = ct{1734};
t6408 = ct{1735};
t6411 = ct{1736};
t6412 = ct{1737};
t6413 = ct{1738};
t6414 = ct{1739};
t6417 = ct{1740};
t6418 = ct{1741};
t6419 = ct{1742};
t642 = ct{1743};
t6420 = ct{1744};
t6422 = ct{1745};
t6423 = ct{1746};
t6425 = ct{1747};
t6426 = ct{1748};
t6428 = ct{1749};
t643 = ct{1750};
t6430 = ct{1751};
t6431 = ct{1752};
t6432 = ct{1753};
t6438 = ct{1754};
t6439 = ct{1755};
t6440 = ct{1756};
t6441 = ct{1757};
t6442 = ct{1758};
t6443 = ct{1759};
t6444 = ct{1760};
t6445 = ct{1761};
t6446 = ct{1762};
t6447 = ct{1763};
t6455 = ct{1764};
t6457 = ct{1765};
t6460 = ct{1766};
t6461 = ct{1767};
t6462 = ct{1768};
t6463 = ct{1769};
t6464 = ct{1770};
t6465 = ct{1771};
t6470 = ct{1772};
t6471 = ct{1773};
t6473 = ct{1774};
t6474 = ct{1775};
t6475 = ct{1776};
t6476 = ct{1777};
t6477 = ct{1778};
t6478 = ct{1779};
t6480 = ct{1780};
t6481 = ct{1781};
t6482 = ct{1782};
t6483 = ct{1783};
t6484 = ct{1784};
t6487 = ct{1785};
t6488 = ct{1786};
t649 = ct{1787};
t6491 = ct{1788};
t6496 = ct{1789};
t6498 = ct{1790};
t6501 = ct{1791};
t6502 = ct{1792};
t6503 = ct{1793};
t6508 = ct{1794};
t6509 = ct{1795};
t6510 = ct{1796};
t6511 = ct{1797};
t6512 = ct{1798};
t6513 = ct{1799};
t6514 = ct{1800};
t6515 = ct{1801};
t6517 = ct{1802};
t6518 = ct{1803};
t6519 = ct{1804};
t6520 = ct{1805};
t6523 = ct{1806};
t6524 = ct{1807};
t6525 = ct{1808};
t6526 = ct{1809};
t6527 = ct{1810};
t6528 = ct{1811};
t6530 = ct{1812};
t6531 = ct{1813};
t6537 = ct{1814};
t6538 = ct{1815};
t6542 = ct{1816};
t6544 = ct{1817};
t6547 = ct{1818};
t6549 = ct{1819};
t6550 = ct{1820};
t6559 = ct{1821};
t6560 = ct{1822};
t6561 = ct{1823};
t6562 = ct{1824};
t6564 = ct{1825};
t6565 = ct{1826};
t6566 = ct{1827};
t6569 = ct{1828};
t6570 = ct{1829};
t6571 = ct{1830};
t6572 = ct{1831};
t6573 = ct{1832};
t6574 = ct{1833};
t6576 = ct{1834};
t6578 = ct{1835};
t6579 = ct{1836};
t6580 = ct{1837};
t6582 = ct{1838};
t6588 = ct{1839};
t6589 = ct{1840};
t6591 = ct{1841};
t6592 = ct{1842};
t6593 = ct{1843};
t6594 = ct{1844};
t6595 = ct{1845};
t6596 = ct{1846};
t6598 = ct{1847};
t6599 = ct{1848};
t6600 = ct{1849};
t6601 = ct{1850};
t6602 = ct{1851};
t6604 = ct{1852};
t6605 = ct{1853};
t6606 = ct{1854};
t6607 = ct{1855};
t6608 = ct{1856};
t6622 = ct{1857};
t6623 = ct{1858};
t6624 = ct{1859};
t6625 = ct{1860};
t6645 = ct{1861};
t6646 = ct{1862};
t6651 = ct{1863};
t6652 = ct{1864};
t6654 = ct{1865};
t6656 = ct{1866};
t6657 = ct{1867};
t6658 = ct{1868};
t6659 = ct{1869};
t6660 = ct{1870};
t6663 = ct{1871};
t6665 = ct{1872};
